simulink model "DFL_IMAP"  (R2018b)
settings: Solver=FixedStepDiscrete  StartTime=0.0  StopTime=10.0  FixedStep=0.01  RelTol=1e-3
(part 3 of 5)

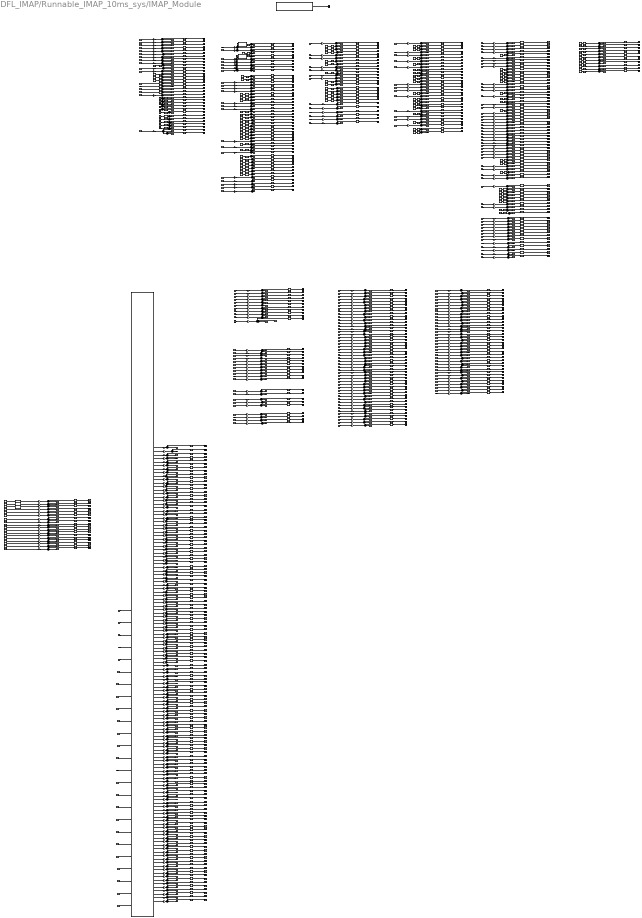
== system DFL_IMAP/Runnable_IMAP_10ms_sys/IMAP_Module ==
  note: SDFA_Lane_Back
  note: SDFA_Lane
  note: SDFA_Obj
  note: SDFA_Sensor_Status
  note: ORI
  note: EMS
  note: BCM
  note: ESC
  note: MP5
  note: EPS
  note: DMS
  SWINve_y_ABS_in_regulation : Inport
  SWINve_g_ACCEL_LONGI_CALIB : Inport  Port=2
  SWINve_y_ASR_ESP_disconnected : Inport  Port=3
  SWINve_y_ASR_in_regulation : Inport  Port=4
  SWINve_y_BCM_State_Front_Wiper : Inport  Port=5
  SWINve_y_Brake_secondary_contact : Inport  Port=6
  SWINve_y_EMS_ACC_Effecitive_EMS : Inport  Port=7
  SWINve_y_EMS_ACCcontrol_Available : Inport  Port=8
  SWINve_g_EMS_Acceleration_pedal_position : Inport  Port=9
  SWINve_g_EMS_Actual_torque : Inport  Port=10
  SWINve_d_EMS_Engine_RPM : Inport  Port=11
  SWINve_y_EMS_Engine_state : Inport  Port=12
  SWINve_g_EMS_WhlTrq_max : Inport  Port=13
  SWINve_g_EMS_WhlTrq_min : Inport  Port=14
  SWINve_y_ESP_in_regulation : Inport  Port=15
  SWINve_y_Front_Left_pulse_malfunction : Inport  Port=16
  SWINve_y_Front_right_pulse_malfunction : Inport  Port=17
  SWINve_y_GW_BCM_SEV_main_state : Inport  Port=18
  SWINve_y_GW_EMS_EMS_Status_ACC : Inport  Port=19
  SWINve_y_GW_Mp5_ISA_Switch : Inport  Port=20
  SWINve_y_GW_Mp5_TSR_Switch : Inport  Port=21
  SWINve_y_High_beam_state : Inport  Port=22
  SWINve_y_IC_Fcw_Activation_Config : Inport  Port=23
  SWINve_y_IC_FCW_Sensitivity : Inport  Port=24
  SWINve_y_IC_passengerBeltSwitchSig : Inport  Port=25
  SWINve_y_IC_seat_bealt_driver_state : Inport  Port=26
  SWINve_y_Internal_SWS_status : Inport  Port=27
  SWINve_g_Lateral_acceleration : Inport  Port=28
  SWINve_y_LC_Mode : Inport  Port=29
  SWINve_y_LKA_main_switch : Inport  Port=30
  SWINve_y_MP5_AEB_Activation_Config : Inport  Port=31
  SWINve_g_No_filtered_front_left_speed : Inport  Port=32
  SWINve_g_No_filtered_front_right_speed : Inport  Port=33
  SWINve_g_No_filtered_rear_left_speed : Inport  Port=34
  SWINve_g_No_filtered_rear_rignt_speed : Inport  Port=35
  SWINve_g_number_of_kilometer : Inport  Port=36
  SWINve_y_Park_brake_function_status : Inport  Port=37
  SWINve_g_Pulse_counter_front_left_wheel : Inport  Port=38
  SWINve_g_Pulse_counter_front_right_wheel : Inport  Port=39
  SWINve_g_Pulse_counter_rearleft_wheel : Inport  Port=40
  SWINve_g_Pulse_counter_rearright_wheel : Inport  Port=41
  SWINve_y_Rear_Left_pulse_malfunction : Inport  Port=42
  SWINve_y_Rear_Right_pulse_malfunction : Inport  Port=43
  SWINve_y_Request_to_light_fault_lamp : Inport  Port=44
  SWINve_y_State_indicating_steer_or_not : Inport  Port=45
  SWINve_y_State_of_EPS_for_LKA_function : Inport  Port=46
  SWINve_g_Steering_wheel_angle : Inport  Port=47
  SWINve_g_Steering_wheel_rotation_speed : Inport  Port=48
  SWINve_y_SWS_calibration : Inport  Port=49
  SWINve_y_SWS_trim : Inport  Port=50
  SWINve_y_TCU_AGB_Target_position : Inport  Port=51
  SWINve_y_TCU_ATFailure : Inport  Port=52
  SWINve_y_TCU_Gear_lever_position : Inport  Port=53
  SWINve_g_TMC_pressure : Inport  Port=54
  SWINve_y_Vehicle_Hold_Status : Inport  Port=55
  SWINve_g_Vehicle_speed_of_wheelsensor : Inport  Port=56
  SWINve_g_Yaw_speed : Inport  Port=57
  System_Clock : Inport  Port=58
  SDFAve_d_sensor_status : Inport  Port=59
  SDFAve_d_sen_sta_LF_radar : Inport  Port=60
  SDFAve_d_sen_sta_RF_radar : Inport  Port=61
  SDFAve_d_sen_sta_LB_radar : Inport  Port=62
  SDFAve_d_sen_sta_RB_radar : Inport  Port=63
  SDFAve_d_fusion_status : Inport  Port=64
  SDFAve_g_fusion_time_stamp : Inport  Port=65
  SDFAve_d_obj_Num : Inport  Port=66
  SDFAva_y_obj_id : Inport  Port=67
  SDFAva_g_obj_pos_x : Inport  Port=68
  SDFAva_g_obj_pos_y : Inport  Port=69
  SDFAva_g_obj_vel_x : Inport  Port=70
  SDFAva_g_obj_vel_y : Inport  Port=71
  SDFAva_g_obj_acc_x : Inport  Port=72
  SDFAva_g_obj_acc_y : Inport  Port=73
  SDFAva_g_obj_pos_var_x : Inport  Port=74
  SDFAva_g_obj_pos_var_y : Inport  Port=75
  SDFAva_g_obj_pos_var_xy : Inport  Port=76
  SDFAva_g_obj_width : Inport  Port=77
  SDFAva_g_obj_length : Inport  Port=78
  SDFAva_y_obj_class : Inport  Port=79
  SDFAva_y_obj_lane : Inport  Port=80
  SDFAva_y_obj_status : Inport  Port=81
  SDFAva_d_obj_age : Inport  Port=82
  SDFAva_y_obj_TurnLight : Inport  Port=83
  SDFAva_y_obj_BrakeLight : Inport  Port=84
  SDFAva_y_obj_MotionStatus : Inport  Port=85
  SDFAve_y_LANE_DETECT_ACTIV : Inport  Port=86
  SDFAve_y_ROAD_TYPE : Inport  Port=87
  SDFAve_y_CONSTRUCTION_AREA : Inport  Port=88
  SDFAve_g_L0_C0_COEF : Inport  Port=89
  SDFAve_g_L0_C1_COEF : Inport  Port=90
  SDFAve_g_L0_C2_COEF : Inport  Port=91
  SDFAve_g_L0_C3_COEF : Inport  Port=92
  SDFAve_g_L0_VIEW_RANGE : Inport  Port=93
  SDFAve_y_L0_DETECT_QUALITY : Inport  Port=94
  SDFAve_d_L0_LINE_TYPE : Inport  Port=95
  SDFAve_g_L0_LINE_COFIDENCE : Inport  Port=96
  SDFAve_g_L0_MARK_WIDTH : Inport  Port=97
  SDFAve_g_L0_TLC : Inport  Port=98
  SDFAve_y_L0_LANE_CHANGE : Inport  Port=99
  SDFAve_g_R0_C0_COEF : Inport  Port=100
  SDFAve_g_R0_C1_COEF : Inport  Port=101
  SDFAve_g_R0_C2_COEF : Inport  Port=102
  SDFAve_g_R0_C3_COEF : Inport  Port=103
  SDFAve_g_R0_VIEW_RANGE : Inport  Port=104
  SDFAve_y_R0_DETECT_QUALITY : Inport  Port=105
  SDFAve_d_R0_LINE_TYPE : Inport  Port=106
  SDFAve_g_R0_LINE_COFIDENCE : Inport  Port=107
  SDFAve_g_R0_MARK_WIDTH : Inport  Port=108
  SDFAve_g_R0_TLC : Inport  Port=109
  SDFAve_y_R0_LANE_CHANGE : Inport  Port=110
  SDFAve_g_L1_C0_COEF : Inport  Port=111
  SDFAve_g_L1_C1_COEF : Inport  Port=112
  SDFAve_g_L1_C2_COEF : Inport  Port=113
  SDFAve_g_L1_C3_COEF : Inport  Port=114
  SDFAve_g_L1_VIEW_RANGE : Inport  Port=115
  SDFAve_y_L1_DETECT_QUALITY : Inport  Port=116
  SDFAve_d_L1_LINE_TYPE : Inport  Port=117
  SDFAve_g_L1_LINE_COFIDENCE : Inport  Port=118
  SDFAve_g_L1_MARK_WIDTH : Inport  Port=119
  SDFAve_g_L1_TLC : Inport  Port=120
  SDFAve_y_L1_LANE_CHANGE : Inport  Port=121
  SDFAve_g_R1_C0_COEF : Inport  Port=122
  SDFAve_g_R1_C1_COEF : Inport  Port=123
  SDFAve_g_R1_C2_COEF : Inport  Port=124
  SDFAve_g_R1_C3_COEF : Inport  Port=125
  SDFAve_g_R1_VIEW_RANGE : Inport  Port=126
  SDFAve_y_R1_DETECT_QUALITY : Inport  Port=127
  SDFAve_d_R1_LINE_TYPE : Inport  Port=128
  SDFAve_g_R1_LINE_COFIDENCE : Inport  Port=129
  SDFAve_g_R1_MARK_WIDTH : Inport  Port=130
  SDFAve_g_R1_TLC : Inport  Port=131
  SDFAve_y_R1_LANE_CHANGE : Inport  Port=132
  SDFAve_g_L0_C0_BACK_COEF : Inport  Port=133
  SDFAve_g_L0_C1_BACK_COEF : Inport  Port=134
  SDFAve_g_L0_C2_BACK_COEF : Inport  Port=135
  SDFAve_g_L0_C3_BACK_COEF : Inport  Port=136
  SDFAve_g_L0_BACK_RANGE : Inport  Port=137
  SDFAve_g_L0_C0_FR_PRE_COEF : Inport  Port=138
  SDFAve_g_L0_C1_FR_PRE_COEF : Inport  Port=139
  SDFAve_g_L0_C2_FR_PRE_COEF : Inport  Port=140
  SDFAve_g_L0_FR_PRED_RANGE : Inport  Port=141
  SDFAve_g_R0_C0_BACK_COEF : Inport  Port=142
  SDFAve_g_R0_C1_BACK_COEF : Inport  Port=143
  SDFAve_g_R0_C2_BACK_COEF : Inport  Port=144
  SDFAve_g_R0_C3_BACK_COEF : Inport  Port=145
  SDFAve_g_R0_BACK_RANGE : Inport  Port=146
  SDFAve_g_R0_C0_FR_PRE_COEF : Inport  Port=147
  SDFAve_g_R0_C1_FR_PRE_COEF : Inport  Port=148
  SDFAve_g_R0_C2_FR_PRE_COEF : Inport  Port=149
  SDFAve_g_R0_FR_PRED_RANGE : Inport  Port=150
  SDFAve_g_L1_C0_BACK_COEF : Inport  Port=151
  SDFAve_g_L1_C1_BACK_COEF : Inport  Port=152
  SDFAve_g_L1_C2_BACK_COEF : Inport  Port=153
  SDFAve_g_L1_C3_BACK_COEF : Inport  Port=154
  SDFAve_g_L1_BACK_RANGE : Inport  Port=155
  SDFAve_g_L1_C0_FR_PRE_COEF : Inport  Port=156
  SDFAve_g_L1_C1_FR_PRE_COEF : Inport  Port=157
  SDFAve_g_L1_C2_FR_PRE_COEF : Inport  Port=158
  SDFAve_g_L1_FR_PRED_RANGE : Inport  Port=159
  SDFAve_g_R1_C0_BACK_COEF : Inport  Port=160
  SDFAve_g_R1_C1_BACK_COEF : Inport  Port=161
  SDFAve_g_R1_C2_BACK_COEF : Inport  Port=162
  SDFAve_g_R1_C3_BACK_COEF : Inport  Port=163
  SDFAve_g_R1_BACK_RANGE : Inport  Port=164
  SDFAve_g_R1_C0_FR_PRE_COEF : Inport  Port=165
  SDFAve_g_R1_C1_FR_PRE_COEF : Inport  Port=166
  SDFAve_g_R1_C2_FR_PRE_COEF : Inport  Port=167
  SDFAve_g_R1_FR_PRED_RANGE : Inport  Port=168
  SDFAve_y_SIGN_ISA_Value : Inport  Port=169
  SDFAve_y_TSR_Sign_Type : Inport  Port=170
  SDFAve_y_CameraSignalFault : Inport  Port=171
  SWINve_y_ESC_FLWDirection : Inport  Port=172  OutDataTypeStr=uint8  PortDimensions=1
  SWINve_y_ESC_FRWDirection : Inport  Port=173  OutDataTypeStr=uint8  PortDimensions=1
  SWINve_y_ESC_TCSErrorStatus : Inport  Port=174  OutDataTypeStr=uint8  PortDimensions=1
  SWINve_y_ESC-RLWDirection : Inport  Port=175  OutDataTypeStr=uint8  PortDimensions=1
  SWINve_y_ESC_RRWDirection : Inport  Port=176  OutDataTypeStr=uint8  PortDimensions=1
  SWINve_y_ESC_EPBErrorStatus : Inport  Port=177  OutDataTypeStr=uint8  PortDimensions=1
  SWINve_y_MP5_AutoPilotSwitch : Inport  Port=178  OutDataTypeStr=uint8
  SWINve_y_Mp5_ISAMode : Inport  Port=179  OutDataTypeStr=uint8  PortDimensions=1
  SWINve_y_Mp5_LDWWarningMode : Inport  Port=180  OutDataTypeStr=uint8  PortDimensions=1
  SWINve_y_MP5_TLCModeSelection : Inport  Port=181  OutDataTypeStr=uint8  PortDimensions=1
  SWINve_y_MP5_ESASwitch : Inport  Port=182  OutDataTypeStr=uint8  PortDimensions=1
  SWINve_y_MP5_BSD_LCW_Activation : Inport  Port=183  OutDataTypeStr=uint8  PortDimensions=1
  SWINve_y_MP5_FCTAActivation : Inport  Port=184  OutDataTypeStr=uint8  PortDimensions=1
  SWINve_y_MP5_RCTAActivation : Inport  Port=185  OutDataTypeStr=uint8  PortDimensions=1
  SWINve_y_MP5_DOWActivation : Inport  Port=186  OutDataTypeStr=uint8  PortDimensions=1
  SWINve_y_MP5_JASwitch : Inport  Port=187  OutDataTypeStr=uint8
  SWINve_y_BCM_DoorLockSt : Inport  Port=188  OutDataTypeStr=uint8  PortDimensions=1
  SWINve_y_BCM_LowBeamStatus : Inport  Port=189
  SWINve_g_AC_AmbTemp : Inport  Port=190
  SWINve_y_ESC_LateralAccelarationValidity : Inport  Port=191  OutDataTypeStr=uint8  PortDimensions=1
  SWINve_y_ESC_YawrateValidity : Inport  Port=192  OutDataTypeStr=uint8
  SWINve_y_ESC_LongitudinalAccelerationValidity : Inport  Port=193  OutDataTypeStr=uint8
  SWINve_y_ESC_ABSValidity : Inport  Port=194  OutDataTypeStr=uint8
  SWINve_y_ESC_FLWHeelSpdFaultSignal : Inport  Port=195  OutDataTypeStr=uint8
  SWINve_y_ESC_FRWHeelSpdFaultSignal : Inport  Port=196  OutDataTypeStr=uint8
  SWINve_y_ESC_RLWHeelSpdFaultSignal : Inport  Port=197  OutDataTypeStr=uint8
  SWINve_y_ESC_RRWHeelSpdFaultSignal : Inport  Port=198  OutDataTypeStr=uint8
  SWINve_y_ESC_AEBAvailable : Inport  Port=199  OutDataTypeStr=uint8
  SWINve_y_ESC_AEBActive : Inport  Port=200  OutDataTypeStr=uint8
  SWINve_y_ESC_ACCAvailable : Inport  Port=201  OutDataTypeStr=uint8
  SWINve_y_ESC_ACCActive : Inport  Port=202  OutDataTypeStr=uint8
  SWINve_y_ESC_EBDAlarmSig : Inport  Port=203  OutDataTypeStr=uint8
  SWINve_y_BCM_LeftlightSt : Inport  Port=204  OutDataTypeStr=uint8  PortDimensions=1
  SWINve_y_BCM_RightlightSt : Inport  Port=205  OutDataTypeStr=uint8  PortDimensions=1
  SWINve_y_BCM_TrunkSt : Inport  Port=206  OutDataTypeStr=uint8  PortDimensions=1
  SWINve_y_BCM_LFDoorSwitchSt : Inport  Port=207  OutDataTypeStr=uint8  PortDimensions=1
  SWINve_y_BCM_RFDoorSwitchSt : Inport  Port=208  OutDataTypeStr=uint8  PortDimensions=1
  SWINve_y_BCM_RRDoorSwitchSt : Inport  Port=209  OutDataTypeStr=uint8  PortDimensions=1
  SWINve_y_BCM_LRDoorSwitchSt : Inport  Port=210  OutDataTypeStr=uint8  PortDimensions=1
  SWINve_y_High_Beam_Status : Inport  Port=211
  SWINve_y_Front_Fog_Lamp_Status : Inport  Port=212
  SWINve_y_Rear_Fog_Lamp_Status : Inport  Port=213
  SWINve_y_BCM1_Rain_Intensity : Inport  Port=214
  SWINve_y_BCM1_IND_OvertakinglampSwt_OnOff : Inport  Port=215
  SWINve_y_kick_down : Inport  Port=216
  SWINve_g_Mech_Loss_Eng_Trq : Inport  Port=217
  SWINve_y_Powertrain_Torque_Validity : Inport  Port=218
  SWINve_y_ESP_Status_ACCInfo_Error : Inport  Port=219
  SWINve_y_ESP_Status_Prefill_Response : Inport  Port=220
  SWINve_y_ESP_Status_AEBJerk_Response : Inport  Port=221
  SWINve_y_ESP_Status_FCW_DBS_Response : Inport  Port=222
  SWINve_y_ESP_Status_AEBJerk_Available : Inport  Port=223
  SWINve_y_ESP_Status_FCW_DBS_Available : Inport  Port=224
  SWINve_y_ESP_Status_Prefill_Available : Inport  Port=225
  SWINve_g_EPS1_IND_LKAOverlayTorque_Value : Inport  Port=226
  SWINve_g_EPS1_IND_DriverTorque_Value : Inport  Port=227
  SWINve_y_EPS1_Status_HandsoffValid : Inport  Port=228
  CAFDva_y_F_CameraData600 : Inport  Port=229  OutDataTypeStr=uint8  PortDimensions=66
  CAFDva_y_F_CameraData424 : Inport  Port=230  OutDataTypeStr=uint8  PortDimensions=66
  CAFDva_y_F_CameraData425 : Inport  Port=231  OutDataTypeStr=uint8  PortDimensions=66
  CAFDva_y_F_CameraData450 : Inport  Port=232  OutDataTypeStr=uint8  PortDimensions=66
  CAFDva_y_F_CameraData459 : Inport  Port=233  OutDataTypeStr=uint8  PortDimensions=66
  CAFDva_y_F_CameraData45A : Inport  Port=234  OutDataTypeStr=uint8  PortDimensions=66
  CAFDva_y_F_CameraData45B : Inport  Port=235  OutDataTypeStr=uint8  PortDimensions=66
  CAFDva_y_F_CameraData45C : Inport  Port=236  OutDataTypeStr=uint8  PortDimensions=66
  CAFDva_y_F_CameraData45D : Inport  Port=237  OutDataTypeStr=uint8  PortDimensions=66
  CAFDva_y_F_CameraData45E : Inport  Port=238  OutDataTypeStr=uint8  PortDimensions=66
  CAFDva_y_F_CameraData45F : Inport  Port=239  OutDataTypeStr=uint8  PortDimensions=66
  CAFDva_y_F_CameraData420 : Inport  Port=240  OutDataTypeStr=uint8  PortDimensions=66
  CAFDva_y_F_CameraData421 : Inport  Port=241  OutDataTypeStr=uint8  PortDimensions=66
  CAFDva_y_F_CameraData422 : Inport  Port=242  OutDataTypeStr=uint8  PortDimensions=66
  CAFDva_y_F_CameraData451 : Inport  Port=243  OutDataTypeStr=uint8  PortDimensions=66
  CAFDva_y_F_CameraData423 : Inport  Port=244  OutDataTypeStr=uint8  PortDimensions=66
  CAFDva_y_F_CameraData452 : Inport  Port=245  OutDataTypeStr=uint8  PortDimensions=66
  CAFDva_y_F_CameraData453 : Inport  Port=246  OutDataTypeStr=uint8  PortDimensions=66
  CAFDva_y_F_CameraData454 : Inport  Port=247  OutDataTypeStr=uint8  PortDimensions=66
  CAFDva_y_F_CameraData455 : Inport  Port=248  OutDataTypeStr=uint8  PortDimensions=66
  CAFDva_y_F_CameraData456 : Inport  Port=249  OutDataTypeStr=uint8  PortDimensions=66
  CAFDva_y_F_CameraData457 : Inport  Port=250  OutDataTypeStr=uint8  PortDimensions=66
  CAFDva_y_F_CameraData458 : Inport  Port=251  OutDataTypeStr=uint8  PortDimensions=66
  CAFDva_y_F_CameraData426 : Inport  Port=252  OutDataTypeStr=uint8  PortDimensions=66
  CAFDva_y_F_CameraData47E : Inport  Port=253  OutDataTypeStr=uint8  PortDimensions=66
  Constant{1..6,8..17,22..23,29,31..32,34,37,43,48..49,51,54,57..59,61,66,71..74,77..90,92..158,163..164} (120 alike) : Constant  Value=0  OutDataTypeStr=uint16  SampleTime=-1
  Constant7 : Constant  Value=0  OutDataTypeStr=uint32  SampleTime=-1
  Data Type Conversion{,8..12,14..17,137,332..333,339,347..348,355..359,372..373,402,424,432..433,435..440,442,444..457,460..466,468,470,473..483,500..521} (90 alike) : DataTypeConversion  OutDataTypeStr=uint16
  Data Type Conversion{1..7,18..136,138..331,342..346,349..354,360..371,374..401,403..423,425..428,458,467,484..499,523..590} (482 alike) : DataTypeConversion
  Data Type Conversion13 : DataTypeConversion  OutDataTypeStr=uint32
  Data Type Conversion{334..338,340..341,429..430,434,441,443,459,469,471..472,522} (17 alike) : DataTypeConversion  OutDataTypeStr=single
  Gain{,288,354..357,359..360,364..370,380..381,384,386..387,390,392,396..397,400..403,405..406,408..416,421..427,432..434} (49 alike) : Gain  OutDataTypeStr=single  SaturateOnIntegerOverflow=on  ParamDataTypeStr=Inherit: Same as input
  Gain{1..2,4..5,8,12..16,19,23,25..30,32,34..37,39..58,63..68,71..72,74..78,81,83..85,87..93,101..103,108..109,138,142,149,155..156,162..163,169..170,176..177,181..189,195..197,203..206,216..218,228..233,235..236,240..241,245,248..249,253,255,259,263,268,272..273,276,279,286..287,289..290,292,304..305,307..308,314,317,336,342..348,350..353,373..374,378..379,385,391,443} (154 alike) : Gain  OutDataTypeStr=uint16
  Gain{3,6..7,9..11,17..18,20..22,24,31,33,38,59..62,69..70,73,104..107,110..137,139..141,143..148,150..154,157..161,164..168,171..175,178..180,191,198..200,213..214,219..227,234,238..239,242..244,246..247,250..252,254,256..258,260,262,264,266..267,270..271,274..275,277..278,281,283,375..377,444} (133 alike) : Gain  OutDataTypeStr=single
  Gain100 : Gain  OutDataTypeStr=uint32
  Gain{237,261,265,269} (4 alike) : Gain  Gain=0.5  OutDataTypeStr=single
  Gain{358,361..363,371..372,382..383,388..389,393..395,398,404,407,417..420,428..431,435..441} (31 alike) : Gain  OutDataTypeStr=uint16  SaturateOnIntegerOverflow=on  ParamDataTypeStr=Inherit: Same as input
  Gain399 : Gain  SaturateOnIntegerOverflow=on  OutDataTypeStr=Inherit: Same as input  ParamDataTypeStr=Inherit: Same as input
  Terminator{1..483} (483 alike) : Terminator
  Version : Constant  Value=331  OutDataTypeStr=uint16
  array_transfer : MATLAB Function  TreatAsAtomicUnit=on
  array_transfer10 : MATLAB Function  TreatAsAtomicUnit=on
  array_transfer11 : MATLAB Function  TreatAsAtomicUnit=on
  array_transfer3 : MATLAB Function  TreatAsAtomicUnit=on
  array_transfer8 : MATLAB Function  TreatAsAtomicUnit=on
  message_unpack : MATLAB Function  TreatAsAtomicUnit=on
  IMAPve_d_LKA_Main_Switch : Outport
  IMAPve_d_LKA_Mode : Outport  Port=2
  IMAPve_d_AEB_Switch : Outport  Port=3
  IMAPve_d_FCW_Switch : Outport  Port=4
  IMAPve_d_FCW_Sensitivity : Outport  Port=5
  IMAPve_d_ISA_Switch : Outport  Port=6
  IMAPve_d_TSR_Switch : Outport  Port=7
  IMAPve_d_ISA_ISLC_Mode : Outport  Port=8
  IMAPve_d_LDW_Warn_Mode : Outport  Port=9
  IMAPve_d_Speed_Limit : Outport  Port=10
  IMAPve_d_ALC_TLC_Mode : Outport  Port=11
  IMAPve_d_ESA_Switch : Outport  Port=12
  IMAPve_d_ELK_Switch : Outport  Port=13
  IMAPve_d_APA_Command : Outport  Port=14
  IMAPve_d_PEPS_RKE_Command : Outport  Port=15
  IMAPve_d_BSD_LCW_Switch : Outport  Port=16
  IMAPve_d_FCTA_Switch : Outport  Port=17
  IMAPve_d_RCTA_Swtich : Outport  Port=18
  IMAPve_d_DOW_Switch : Outport  Port=19
  IMAPve_d_JA_Brake_Switch : Outport  Port=20
  IMAPve_d_JA_Alert_Switch : Outport  Port=21
  IMAPve_d_JA_Alert_Sensitivity : Outport  Port=22
  IMAPve_d_LF_Switch : Outport  Port=23
  IMAPve_d_ICA_Config : Outport  Port=24
  IMAPve_d_ALC_Sensitivity : Outport  Port=25
  IMAPve_d_EPS_LKA_State : Outport  Port=26
  IMAPve_g_EPS_SW_Trq : Outport  Port=27
  IMAPve_d_EPS_Error_State : Outport  Port=28
  IMAPve_d_EPS_Trq_State : Outport  Port=29
  IMAPve_d_SAS_Clb_State : Outport  Port=30
  IMAPve_d_SAS_Trim_State : Outport  Port=31
  IMAPve_d_EPS_TrqLim_State : Outport  Port=32
  IMAPve_g_EPS_LKA_Current : Outport  Port=33
  IMAPve_g_ESC_LatAcc : Outport  Port=34
  IMAPve_d_ESC_LatAcc_Valid : Outport  Port=35
  IMAPve_g_ESC_YawRate : Outport  Port=36
  IMAPve_d_ESC_YawRate_Valid : Outport  Port=37
  IMAPve_g_ESC_UnYawRate : Outport  Port=38
  IMAPve_g_ESC_VehSpd : Outport  Port=39
  IMAPve_g_ESC_LonAcc : Outport  Port=40
  IMAPve_d_ESC_LonAcc_Valid : Outport  Port=41
  IMAPve_g_ESC_Brake_Press : Outport  Port=42
  IMAPve_g_ESC_Static_Slope : Outport  Port=43
  IMAPve_g_ESC_DySlope_Accuracy : Outport  Port=44
  IMAPve_g_ESC_DySlope : Outport  Port=45
  IMAPve_g_SW_Angle : Outport  Port=46
  IMAPve_g_SW_Angle_Speed : Outport  Port=47
  IMAPve_d_BCM_HazardLamp : Outport  Port=48
  IMAPve_d_BCM_Left_Light : Outport  Port=49
  IMAPve_d_BCM_Right_Light : Outport  Port=50
  IMAPve_d_ESC_BrakeLamp_Req : Outport  Port=51
  IMAPve_d_BCM_Opening_State : Outport  Port=52
  IMAPve_d_BCM_Trunk_State : Outport  Port=53
  IMAPve_d_BCM_LF_Door_State : Outport  Port=54
  IMAPve_d_BCM_RF_Door_State : Outport  Port=55
  IMAPve_d_BCM_RR_Door_State : Outport  Port=56
  IMAPve_d_BCM_LR_Door_State : Outport  Port=57
  IMAPve_d_SCC_Right_SwitchSig : Outport  Port=58
  IMAPve_d_PEPS_Door_Lock_Req : Outport  Port=59
  IMAPve_d_BCM_Door_Lock_State : Outport  Port=60
  IMAPve_d_EMS_ACC_Status : Outport  Port=61
  IMAPve_g_EMS_Pot_WhlT_Max : Outport  Port=62
  IMAPve_g_EMS_Pot_WhlT_Min : Outport  Port=63
  IMAPve_g_EMS_RealPedal : Outport  Port=64
  IMAPve_g_EMS_MaxTWhl : Outport  Port=65
  IMAPve_g_EMS_MaxTWhl_Offset : Outport  Port=66
  IMAPve_g_EMS_MinTWhl : Outport  Port=67
  IMAPve_g_EMS_MinTWhl_Offset : Outport  Port=68
  IMAPve_g_EMS_Actual_FlwT : Outport  Port=69
  IMAPve_g_EMS_Actual_IndT : Outport  Port=70
  IMAPve_g_EMS_Realize_TWhl : Outport  Port=71
  IMAPve_g_EMS_ACC_VirtualPedal : Outport  Port=72
  IMAPve_d_EMS_AccPedal_Fault : Outport  Port=73
  IMAPve_g_EMS_Driver_Torque : Outport  Port=74
  IMAPve_d_ESC_Brake_Effort : Outport  Port=75
  IMAPve_g_EMS_Engine_Speed : Outport  Port=76
  IMAPve_d_ESC_Veh_Standstill : Outport  Port=77
  IMAPve_d_TCU_Actual_Gear : Outport  Port=78
  IMAPve_d_TCU_Target_Gear : Outport  Port=79
  IMAPve_d_TCU_PRND_State : Outport  Port=80
  IMAPve_d_BCM_Ignition_State : Outport  Port=81
  IMAPve_d_ACU_Driver_Belt : Outport  Port=82
  IMAPve_d_SWS_Fault_Code : Outport  Port=83
  IMAPve_d_SWS_Failure_Status : Outport  Port=84
  IMAPve_d_ESC_OFF : Outport  Port=85
  IMAPve_d_ESC_AlarmSig : Outport  Port=86
  IMAPve_d_Speed_Limit_Switch : Outport  Port=87
  IMAPve_d_ESC_ESC_Active : Outport  Port=88
  IMAPve_d_ESC_MSR_Active : Outport  Port=89
  IMAPve_d_ESC_TCS_Active : Outport  Port=90
  IMAPve_d_ESC_VehSpd_Valid : Outport  Port=91
  IMAPve_d_Brake_Pedal_Fault : Outport  Port=92
  IMAPve_d_ESC_ABS_Active : Outport  Port=93
  IMAPve_d_ESC_ABS_Valid : Outport  Port=94
  IMAPve_d_ESC_ABS_AlarmSig : Outport  Port=95
  IMAPve_d_ESC_FL_WheelPulVal : Outport  Port=96
  IMAPve_d_ESC_FR_WheelPulVal : Outport  Port=97
  IMAPve_d_ESC_RL_WheelPulVal : Outport  Port=98
  IMAPve_d_ESC_RR_WheelPulVal : Outport  Port=99
  IMAPve_g_ESC_FL_WhlSpd : Outport  Port=100
  IMAPve_d_ESC_FL_WhlSpd_Fault : Outport  Port=101
  IMAPve_g_ESC_FR_WhlSpd : Outport  Port=102
  IMAPve_d_ESC_FR_WhlSpd_Fault : Outport  Port=103
  IMAPve_g_ESC_RL_WhlSpd : Outport  Port=104
  IMAPve_d_ESC_RL_WhlSpd_Fault : Outport  Port=105
  IMAPve_g_ESC_RR_WhlSpd : Outport  Port=106
  IMAPve_d_ESC_RR_WhlSpd_Fault : Outport  Port=107
  IMAPve_d_ESC_FL_Wheel_Pulse : Outport  Port=108
  IMAPve_d_ESC_FR_Wheel_Pulse : Outport  Port=109
  IMAPve_d_ESC_RL_Wheel_Pulse : Outport  Port=110
  IMAPve_d_ESC_RR_Wheel_Pulse : Outport  Port=111
  IMAPve_d_TCU_AT_Failure : Outport  Port=112
  IMAPve_d_TCU_Shift_Valid : Outport  Port=113
  IMAPve_d_TCU_DCT_Clutch_State : Outport  Port=114
  IMAPve_d_TCU_Gear_Engage : Outport  Port=115
  IMAPve_d_TCU_Select_ATMode : Outport  Port=116
  IMAPve_d_EMS_Engine_Status : Outport  Port=117
  IMAPve_d_EMS_Gearbox_CtlAvail : Outport  Port=118
  IMAPve_d_ESC_Brake_Failsafe : Outport  Port=119
  IMAPve_d_ESC_AEB_Status : Outport  Port=120
  IMAPve_d_ESC_AEB_Available : Outport  Port=121
  IMAPve_d_ESC_AEB_Active : Outport  Port=122
  IMAPve_d_ESC_ACC_Status : Outport  Port=123
  IMAPve_d_ESC_ACC_Available : Outport  Port=124
  IMAPve_d_ESC_ACC_Active : Outport  Port=125
  IMAPve_d_EMS_ACC_Effective : Outport  Port=126
  IMAPve_d_BCM_FrontWiper_State : Outport  Port=127
  IMAPve_d_BCM_CHMSL_Status : Outport  Port=128
  IMAPve_d_BCM_BrakeLamp_State : Outport  Port=129
  IMAPve_d_GW_Brake_Only_Req : Outport  Port=130
  IMAPve_d_ACU_Passenger_Belt : Outport  Port=131
  IMAPve_d_EMS_ACC_CtlAvail : Outport  Port=132
  IMAPve_d_EMS_ACC_Inhibited : Outport  Port=133
  IMAPve_d_EMS_Brake_Pedal : Outport  Port=134
  IMAPve_d_BCM_LowBeam_State : Outport  Port=135
  IMAPve_d_BCM_HighBeam_State : Outport  Port=136
  IMAPve_d_EPB_Status : Outport  Port=137
  IMAPve_d_EPB_Display_Req : Outport  Port=138
  IMAPve_d_EPB_Warn_Req : Outport  Port=139
  IMAPve_d_EPB_Switch_State : Outport  Port=140
  IMAPve_d_EPB_Switch_Valid : Outport  Port=141
  IMAPve_d_ESC_Drive_Direction : Outport  Port=142
  IMAPve_d_ESC_Hold_State : Outport  Port=143
  IMAPve_d_EPS_Steer_Hold_State : Outport  Port=144
  IMAPve_d_EPS_Warning_State : Outport  Port=145
  IMAPve_g_EPS_PowerCon : Outport  Port=146
  IMAPve_d_ESC_EBD_AlarmSig : Outport  Port=147
  IMAPve_d_ESC_AVH_Status : Outport  Port=148
  IMAPve_d_Radar_Detective_Req : Outport  Port=149
  IMAPve_g_BCM_Battery_Voltage : Outport  Port=150
  IMAPve_d_TBOX_LocalTimeY : Outport  Port=151
  IMAPve_d_TBOX_LocalTimeM : Outport  Port=152
  IMAPve_d_TBOX_LocalTimeD : Outport  Port=153
  IMAPve_d_TBOX_LocalTimeH : Outport  Port=154
  IMAPve_d_TBOX_LocalTimeMin : Outport  Port=155
  IMAPve_d_TBOX_LocalTimeS : Outport  Port=156
  IMAPve_d_TBOX_LocalTime_Valid : Outport  Port=157
  IMAPve_d_TPMS_Warn_Indicate : Outport  Port=158
  IMAPve_d_Radar_State : Outport  Port=159
  IMAPve_d_ACC_Desired_Headway : Outport  Port=160
  IMAPve_d_Time_System_Clock : Outport  Port=161
  IMAPve_d_Signal_Time_Stamp : Outport  Port=162
  IMAPve_g_GW_IC_Odometer : Outport  Port=163
  IMAPve_g_FAPA_State : Outport  Port=164
  IMAPve_d_Outside_Temp : Outport  Port=165
  IMAPve_d_ORI_CIPV_ID : Outport  Port=166
  IMAPve_d_ORI_Obj_Num : Outport  Port=167
  IMAPva_g_ORI_Probability : Outport  Port=168
  IMAPva_d_ORI_Obj_Class : Outport  Port=169
  IMAPva_d_ORI_Obj_Motion : Outport  Port=170
  IMAPva_g_ORI_Obj_RelVel : Outport  Port=171
  IMAPva_g_ORI_Obj_LongDis : Outport  Port=172
  IMAPva_d_ORI_Obj_Lane : Outport  Port=173
  IMAPva_g_ORI_Obj_LAngle : Outport  Port=174
  IMAPva_g_ORI_Obj_RAngle : Outport  Port=175
  IMAPva_g_ORI_Obj_Width : Outport  Port=176
  IMAPva_d_ORI_Obj_ID : Outport  Port=177
  IMAPve_d_ORI_Lane_Valid : Outport  Port=178
  IMAPve_d_ORI_Lane_ConsArea : Outport  Port=179
  IMAPve_d_ORI_Lane_RoadType : Outport  Port=180
  IMAPve_g_ORI_L0_C3 : Outport  Port=181
  IMAPve_g_ORI_L0_C2 : Outport  Port=182
  IMAPve_g_ORI_L0_C1 : Outport  Port=183
  IMAPve_g_ORI_L0_C0 : Outport  Port=184
  IMAPve_d_ORI_L0_Q : Outport  Port=185
  IMAPve_d_ORI_L0_Type : Outport  Port=186
  IMAPve_g_ORI_L0_VR : Outport  Port=187
  IMAPve_g_ORI_L0_TLC : Outport  Port=188
  IMAPve_g_ORI_L0_W : Outport  Port=189
  IMAPve_d_ORI_L0_LC : Outport  Port=190
  IMAPve_g_ORI_L1_C3 : Outport  Port=191
  IMAPve_g_ORI_L1_C2 : Outport  Port=192
  IMAPve_g_ORI_L1_C1 : Outport  Port=193
  IMAPve_g_ORI_L1_C0 : Outport  Port=194
  IMAPve_d_ORI_L1_Q : Outport  Port=195
  IMAPve_d_ORI_L1_Type : Outport  Port=196
  IMAPve_g_ORI_L1_VR : Outport  Port=197
  IMAPve_g_ORI_L1_TLC : Outport  Port=198
  IMAPve_g_ORI_L1_W : Outport  Port=199
  IMAPve_d_ORI_L1_LC : Outport  Port=200
  IMAPve_g_ORI_R0_C3 : Outport  Port=201
  IMAPve_g_ORI_R0_C2 : Outport  Port=202
  IMAPve_g_ORI_R0_C1 : Outport  Port=203
  IMAPve_g_ORI_R0_C0 : Outport  Port=204
  IMAPve_d_ORI_R0_Q : Outport  Port=205
  IMAPve_d_ORI_R0_LT : Outport  Port=206
  IMAPve_g_ORI_R0_VR : Outport  Port=207
  IMAPve_g_ORI_R0_TLC : Outport  Port=208
  IMAPve_g_ORI_R0_W : Outport  Port=209
  IMAPve_d_ORI_R0_LC : Outport  Port=210
  IMAPve_g_ORI_R1_C3 : Outport  Port=211
  IMAPve_g_ORI_R1_C2 : Outport  Port=212
  IMAPve_g_ORI_R1_C1 : Outport  Port=213
  IMAPve_g_ORI_R1_C0 : Outport  Port=214
  IMAPve_d_ORI_R1_Q : Outport  Port=215
  IMAPve_d_ORI_R1_LT : Outport  Port=216
  IMAPve_g_ORI_R1_VR : Outport  Port=217
  IMAPve_g_ORI_R1_TLC : Outport  Port=218
  IMAPve_g_ORI_R1_W : Outport  Port=219
  IMAPve_d_ORI_R1_LC : Outport  Port=220
  IMAPve_d_Sensor_Status : Outport  Port=221
  IMAPve_d_LF_Radar_Status : Outport  Port=222
  IMAPve_d_RF_Radar_Status : Outport  Port=223
  IMAPve_d_LR_Radar_Status : Outport  Port=224
  IMAPve_d_RR_Radar_Status : Outport  Port=225
  IMAPve_d_Fusion_Status : Outport  Port=226
  IMAPve_g_Fusion_Time_Stamp : Outport  Port=227
  IMAPve_d_obj_Num : Outport  Port=228
  IMAPva_d_obj_id : Outport  Port=229
  IMAPva_g_obj_pos_x : Outport  Port=230
  IMAPva_g_obj_pos_y : Outport  Port=231
  IMAPva_g_obj_vel_x : Outport  Port=232
  IMAPva_g_obj_vel_y : Outport  Port=233
  IMAPva_g_obj_acc_x : Outport  Port=234
  IMAPva_g_obj_acc_y : Outport  Port=235
  IMAPva_g_obj_pos_var_x : Outport  Port=236
  IMAPva_g_obj_pos_var_y : Outport  Port=237
  IMAPva_g_obj_pos_var_xy : Outport  Port=238
  IMAPva_g_obj_width : Outport  Port=239
  IMAPva_g_obj_length : Outport  Port=240
  IMAPva_d_obj_class : Outport  Port=241
  IMAPva_d_obj_lane : Outport  Port=242
  IMAPva_d_obj_status : Outport  Port=243
  IMAPva_d_obj_age : Outport  Port=244
  IMAPva_d_obj_TurnLight : Outport  Port=245
  IMAPva_d_obj_BrakeLight : Outport  Port=246
  IMAPva_d_obj_MotionStatus : Outport  Port=247
  IMAPve_d_Lane_Valid : Outport  Port=248
  IMAPve_d_Road_Type : Outport  Port=249
  IMAPve_d_ConsArea : Outport  Port=250
  IMAPve_g_L0_C0 : Outport  Port=251
  IMAPve_g_L0_C1 : Outport  Port=252
  IMAPve_g_L0_C2 : Outport  Port=253
  IMAPve_g_L0_C3 : Outport  Port=254
  IMAPve_g_L0_VR : Outport  Port=255
  IMAPve_d_L0_Q : Outport  Port=256
  IMAPve_d_L0_Type : Outport  Port=257
  IMAPve_g_L0_Confidence : Outport  Port=258
  IMAPve_g_L0_W : Outport  Port=259
  IMAPve_g_L0_TLC : Outport  Port=260
  IMAPve_d_L0_LC : Outport  Port=261
  IMAPve_g_R0_C0 : Outport  Port=262
  IMAPve_g_R0_C1 : Outport  Port=263
  IMAPve_g_R0_C2 : Outport  Port=264
  IMAPve_g_R0_C3 : Outport  Port=265
  IMAPve_g_R0_VR : Outport  Port=266
  IMAPve_d_R0_Q : Outport  Port=267
  IMAPve_d_R0_Type : Outport  Port=268
  IMAPve_g_R0_Confidence : Outport  Port=269
  IMAPve_g_R0_W : Outport  Port=270
  IMAPve_g_R0_TLC : Outport  Port=271
  IMAPve_d_R0_LC : Outport  Port=272
  IMAPve_g_L1_C0 : Outport  Port=273
  IMAPve_g_L1_C1 : Outport  Port=274
  IMAPve_g_L1_C2 : Outport  Port=275
  IMAPve_g_L1_C3 : Outport  Port=276
  IMAPve_g_L1_VR : Outport  Port=277
  IMAPve_d_L1_Q : Outport  Port=278
  IMAPve_d_L1_Type : Outport  Port=279
  IMAPve_g_L1_Confidence : Outport  Port=280
  IMAPve_g_L1_W : Outport  Port=281
  IMAPve_g_L1_TLC : Outport  Port=282
  IMAPve_d_L1_LC : Outport  Port=283
  IMAPve_g_R1_C0 : Outport  Port=284
  IMAPve_g_R1_C1 : Outport  Port=285
  IMAPve_g_R1_C2 : Outport  Port=286
  IMAPve_g_R1_C3 : Outport  Port=287
  IMAPve_g_R1_VR : Outport  Port=288
  IMAPve_d_R1_Q : Outport  Port=289
  IMAPve_d_R1_Type : Outport  Port=290
  IMAPve_g_R1_Confidence : Outport  Port=291
  IMAPve_g_R1_W : Outport  Port=292
  IMAPve_g_R1_TLC : Outport  Port=293
  IMAPve_d_R1_LC : Outport  Port=294
  IMAPve_g_L0_C0_Back : Outport  Port=295
  IMAPve_g_L0_C1_Back : Outport  Port=296
  IMAPve_g_L0_C2_Back : Outport  Port=297
  IMAPve_g_L0_C3_Back : Outport  Port=298
  IMAPve_g_L0_Range_Back : Outport  Port=299
  IMAPve_g_L0_C0_FR_Pred : Outport  Port=300
  IMAPve_g_L0_C1_FR_Pred : Outport  Port=301
  IMAPve_g_L0_C2_FR_Pred : Outport  Port=302
  IMAPve_g_L0_Range_FR_Pred : Outport  Port=303
  IMAPve_g_R0_C0_Back : Outport  Port=304
  IMAPve_g_R0_C1_Back : Outport  Port=305
  IMAPve_g_R0_C2_Back : Outport  Port=306
  IMAPve_g_R0_C3_Back : Outport  Port=307
  IMAPve_g_R0_Range_Back : Outport  Port=308
  IMAPve_g_R0_C0_FR_Pred : Outport  Port=309
  IMAPve_g_R0_C1_FR_Pred : Outport  Port=310
  IMAPve_g_R0_C2_FR_Pred : Outport  Port=311
  IMAPve_g_R0_Range_FR_Pred : Outport  Port=312
  IMAPve_g_L1_C0_Back : Outport  Port=313
  IMAPve_g_L1_C1_Back : Outport  Port=314
  IMAPve_g_L1_C2_Back : Outport  Port=315
  IMAPve_g_L1_C3_Back : Outport  Port=316
  IMAPve_g_L1_Range_Back : Outport  Port=317
  IMAPve_g_L1_C0_FR_Pred : Outport  Port=318
  IMAPve_g_L1_C1_FR_Pred : Outport  Port=319
  IMAPve_g_L1_C2_FR_Pred : Outport  Port=320
  IMAPve_g_L1_Range_FR_Pred : Outport  Port=321
  IMAPve_g_R1_C0_Back : Outport  Port=322
  IMAPve_g_R1_C1_Back : Outport  Port=323
  IMAPve_g_R1_C2_Back : Outport  Port=324
  IMAPve_g_R1_C3_Back : Outport  Port=325
  IMAPve_g_R1_Range_Back : Outport  Port=326
  IMAPve_g_R1_C0_FR_Pred : Outport  Port=327
  IMAPve_g_R1_C1_FR_Pred : Outport  Port=328
  IMAPve_g_R1_C2_FR_Pred : Outport  Port=329
  IMAPve_g_R1_Range_FR_Pred : Outport  Port=330
  IMAPve_d_Sign_ISA_Value : Outport  Port=331
  IMAPve_d_TSR_Sign_Type : Outport  Port=332
  IMAPve_d_Camera_Signal_Fault : Outport  Port=333
  IMAPve_d_Radar_Status : Outport  Port=334
  IMAPve_d_Camera_Status : Outport  Port=335
  IMAPve_d_ESC_FLW_Direction : Outport  Port=336
  IMAPve_d_ESC_FRW_Direction : Outport  Port=337
  IMAPve_d_ESC_TCS_ErrorStatus : Outport  Port=338
  IMAPve_d_ESC_RLW_Direction : Outport  Port=339
  IMAPve_d_ESC_RRW_Direction : Outport  Port=340
  IMAPve_d_ESC_EPB_ErrorStatus : Outport  Port=341
  IMAPve_d_EPS_SteeringAngle_Flag : Outport  Port=342
  IMAPve_g_EPS_SteeringAngle : Outport  Port=343
  IMAPve_d_EPS_Driver_Override : Outport  Port=344
  IMAPve_d_EPS_Driver_Active_ESA : Outport  Port=345
  IMAPve_d_EPS_ESA_State : Outport  Port=346
  IMAPve_d_ACU_RearLeft_Belt : Outport  Port=347
  IMAPve_d_ACU_RearMiddle_Belt : Outport  Port=348
  IMAPve_d_ACU_RearRight_Belt : Outport  Port=349
  IMAPve_d_EMS_PowertrainCtl_State : Outport  Port=350
  IMAPve_d_TCU_TCU_Available : Outport  Port=351
  IMAPve_d_BCM_LeftTurn_Switch : Outport  Port=352
  IMAPve_d_BCM_RightTurn_Switch : Outport  Port=353
  IMAPve_d_BCM_FrontWiper_Switch : Outport  Port=354
  IMAPve_d_BCM_IHBC_Enabled : Outport  Port=355
  IMAPve_d_MP5_Work_State : Outport  Port=356
  IMAPve_d_MP5_APA_ModeSelect : Outport  Port=357
  IMAPve_d_MP5_LanguageSet : Outport  Port=358
  IMAPve_d_MP5_UPA_Switch : Outport  Port=359
  IMAPve_d_MP5_FLK_Activation : Outport  Port=360
  IMAPve_d_MP5_AutoPilot_Switch : Outport  Port=361
  IMAPve_d_SCC_Left_SwitchSig : Outport  Port=362
  IMAPve_d_MP5_DMS_MessageType : Outport  Port=363
  IMAPve_d_MP5_DMS_SystemEnable : Outport  Port=364
  IMAPve_d_MP5_DMS_DelUserNum : Outport  Port=365
  IMAPve_d_MP5_DMS_Sensity : Outport  Port=366
  IMAPve_d_MP5_DMS_EyeFatigue : Outport  Port=367
  IMAPve_d_MP5_DMS_LongtimeDrive : Outport  Port=368
  IMAPve_d_MP5_DMS_SideView : Outport  Port=369
  IMAPve_d_MP5_DMS_UsingPhone : Outport  Port=370
  IMAPve_d_MP5_DMS_Smoking : Outport  Port=371
  IMAPve_d_MP5_DMS_DrinkWater : Outport  Port=372
  IMAPve_d_MP5_DMS_UserAccount : Outport  Port=373
  IMAPve_d_High_Beam_State : Outport  Port=374
  IMAPve_d_Front_Fog_Lamp_State : Outport  Port=375
  IMAPve_d_Rear_Fog_Lamp_State : Outport  Port=376
  IMAPve_d_BCM_Rain_Intensity : Outport  Port=377
  IMAPve_d_BCM_OvertakinglampSwt : Outport  Port=378
  IMAPve_d_EMS_Kickdown : Outport  Port=379
  IMAPve_g_EMS_Mech_Loss_Trq : Outport  Port=380
  IMAPve_d_Powertrain_Torque_Valid : Outport  Port=381
  IMAPve_d_ESC_ACCInfo_Error : Outport  Port=382
  IMAPve_d_ESC_Prefill_Response : Outport  Port=383
  IMAPve_d_ESC_AEBJerk_Response : Outport  Port=384
  IMAPve_d_ESC_FCW_DBS_Response : Outport  Port=385
  IMAPve_d_ESC_AEBJerk_Available : Outport  Port=386
  IMAPve_d_ESC_FCW_DBS_Available : Outport  Port=387
  IMAPve_d_ESC_Prefill_Available : Outport  Port=388
  IMAPve_g_EPS_LKAOverlay_Trq : Outport  Port=389
  IMAPve_g_EPS_DriverTorque : Outport  Port=390
  IMAPve_d_EPS_Steer_Hold_State_Valid : Outport  Port=391
  IMAPva_d_ORI_Obj_TimeStamp : Outport  Port=392  OutDataTypeStr=uint16  PortDimensions=20
  IMAPve_d_ORI_FS_OutOfCalib : Outport  Port=393  OutDataTypeStr=uint16
  IMAPve_d_ORI_FS_Rain : Outport  Port=394  OutDataTypeStr=uint16
  IMAPve_d_ORI_FS_Fog : Outport  Port=395  OutDataTypeStr=uint16
  IMAPve_d_ORI_FS_Splashes0 : Outport  Port=396  OutDataTypeStr=uint16
  IMAPve_d_ORI_FS_SunRay0 : Outport  Port=397  OutDataTypeStr=uint16
  IMAPve_d_ORI_FS_LowSun0 : Outport  Port=398  OutDataTypeStr=uint16
  IMAPve_d_ORI_FS_BlurImage0 : Outport  Port=399  OutDataTypeStr=uint16
  IMAPve_d_ORI_FS_PartialBlockage0 : Outport  Port=400  OutDataTypeStr=uint16
  IMAPve_d_ORI_FS_FullBlockage0 : Outport  Port=401  OutDataTypeStr=uint16
  IMAPve_d_ORI_FS_FrozenWindshield0 : Outport  Port=402  OutDataTypeStr=uint16
  IMAPve_d_ORI_FS_OutOfFocus0 : Outport  Port=403  OutDataTypeStr=uint16
  IMAPva_g_ORI_Obj_AbsAx : Outport  Port=404  OutDataTypeStr=single  PortDimensions=20
  IMAPva_g_ORI_Obj_AbsAy : Outport  Port=405  OutDataTypeStr=single  PortDimensions=20
  IMAPva_g_ORI_Obj_TTIPCStdDev : Outport  Port=406  OutDataTypeStr=single  PortDimensions=20
  IMAPva_g_ORI_Obj_RelVely : Outport  Port=407  OutDataTypeStr=single  PortDimensions=20
  IMAPva_g_ORI_Obj_LateralDis : Outport  Port=408  OutDataTypeStr=single  PortDimensions=20
  IMAPva_g_ORI_Obj_AbsAxStdDev : Outport  Port=409  OutDataTypeStr=single  PortDimensions=20
  IMAPva_g_ORI_Obj_AbsAyStdDev : Outport  Port=410  OutDataTypeStr=single  PortDimensions=20
  IMAPva_g_ORI_Obj_RelVelStdDev : Outport  Port=411  OutDataTypeStr=single  PortDimensions=20
  IMAPva_g_ORI_Obj_RelVelyStdDev : Outport  Port=412  OutDataTypeStr=single  PortDimensions=20
  IMAPva_g_ORI_Obj_LongDisStdDev : Outport  Port=413  OutDataTypeStr=single  PortDimensions=20
  IMAPva_g_ORI_Obj_LateralDisStdDev : Outport  Port=414  OutDataTypeStr=single  PortDimensions=20
  IMAPva_d_ORI_Obj_RelVelValid : Outport  Port=415  OutDataTypeStr=uint16  PortDimensions=20
  IMAPva_d_ORI_Obj_RelVelyValid : Outport  Port=416  OutDataTypeStr=uint16  PortDimensions=20
  IMAPva_d_ORI_Obj_RelVelStdDevValid : Outport  Port=417  OutDataTypeStr=uint16  PortDimensions=20
  IMAPva_d_ORI_Obj_RelVelyStdDevValid : Outport  Port=418  OutDataTypeStr=uint16  PortDimensions=20
  IMAPva_g_ORI_Obj_ExistProb : Outport  Port=419  OutDataTypeStr=single  PortDimensions=20
  IMAPva_g_ORI_Obj_ClassProb : Outport  Port=420  OutDataTypeStr=single  PortDimensions=20
  IMAPva_g_ORI_Obj_Height : Outport  Port=421  OutDataTypeStr=single  PortDimensions=20
  IMAPva_g_ORI_Obj_LengthStdDev : Outport  Port=422  OutDataTypeStr=single  PortDimensions=20
  IMAPva_g_ORI_Obj_WidthStdDev : Outport  Port=423  OutDataTypeStr=single  PortDimensions=20
  IMAPva_g_ORI_Obj_HeightStdDev : Outport  Port=424  OutDataTypeStr=single  PortDimensions=20
  IMAPva_g_ORI_Obj_3DAngle : Outport  Port=425  OutDataTypeStr=single  PortDimensions=20
  IMAPva_g_ORI_Obj_LAngleStdDev : Outport  Port=426  OutDataTypeStr=single  PortDimensions=20
  IMAPva_g_ORI_Obj_RAngleStdDev : Outport  Port=427  OutDataTypeStr=single  PortDimensions=20
  IMAPva_g_ORI_Obj_3DAngleStdDev : Outport  Port=428  OutDataTypeStr=single  PortDimensions=20
  IMAPva_g_ORI_Obj_AngleRate : Outport  Port=429  OutDataTypeStr=single  PortDimensions=20
  IMAPva_g_ORI_Obj_AngleRateStdDev : Outport  Port=430  OutDataTypeStr=single  PortDimensions=20
  IMAPva_g_ORI_Obj_PhiBottom : Outport  Port=431  OutDataTypeStr=single  PortDimensions=20
  IMAPva_g_ORI_Obj_PhiBottomStdDev : Outport  Port=432  OutDataTypeStr=single  PortDimensions=20
  IMAPva_d_ORI_Obj_Measured : Outport  Port=433  OutDataTypeStr=uint16  PortDimensions=20
  IMAPva_g_ORI_Obj_Heading : Outport  Port=434  OutDataTypeStr=single  PortDimensions=20
  IMAPva_g_ORI_Obj_HeadingStdDev : Outport  Port=435  OutDataTypeStr=single  PortDimensions=20
  IMAPva_d_ORI_Obj_HeadOrientation : Outport  Port=436  OutDataTypeStr=uint16  PortDimensions=20
  IMAPva_g_ORI_Obj_TTIPC : Outport  Port=437  OutDataTypeStr=single  PortDimensions=20
  IMAPva_d_ORI_Obj_DirectionIndicator : Outport  Port=438  OutDataTypeStr=uint16  PortDimensions=20
  IMAPva_d_ORI_Obj_BrakeLight : Outport  Port=439  OutDataTypeStr=uint16  PortDimensions=20
  IMAPve_d_ORI_L0_ID : Outport  Port=440  OutDataTypeStr=uint16
  IMAPve_g_ORI_L0_ExistProb : Outport  Port=441  OutDataTypeStr=single
  IMAPve_g_ORI_L0_DxStart : Outport  Port=442  OutDataTypeStr=single
  IMAPve_d_ORI_L0_ColorClass : Outport  Port=443  OutDataTypeStr=uint16
  IMAPve_d_ORI_L0_MeasureType : Outport  Port=444  OutDataTypeStr=uint16
  IMAPve_g_ORI_L0_TypeConf : Outport  Port=445  OutDataTypeStr=single
  IMAPve_d_ORI_R0_ID : Outport  Port=446  OutDataTypeStr=uint16
  IMAPve_g_ORI_R0_ExistProb : Outport  Port=447  OutDataTypeStr=single
  IMAPve_g_ORI_R0_Dxstart : Outport  Port=448  OutDataTypeStr=single
  IMAPve_d_ORI_R0_ColorClass : Outport  Port=449  OutDataTypeStr=uint16
  IMAPve_d_ORI_R0_MeasureType : Outport  Port=450  OutDataTypeStr=uint16
  IMAPve_g_ORI_R0_TypeConf : Outport  Port=451  OutDataTypeStr=single
  IMAPve_d_ORI_L1_ID : Outport  Port=452  OutDataTypeStr=uint16
  IMAPve_g_ORI_L1_ExistProb : Outport  Port=453  OutDataTypeStr=single
  IMAPve_g_ORI_L1_Dxstart : Outport  Port=454  OutDataTypeStr=single
  IMAPve_d_ORI_L1_ColorClass : Outport  Port=455  OutDataTypeStr=uint16
  IMAPve_d_ORI_L1_MeasureType : Outport  Port=456  OutDataTypeStr=uint16
  IMAPve_g_ORI_L1_TypeConf : Outport  Port=457  OutDataTypeStr=single
  IMAPve_d_ORI_R1_ID : Outport  Port=458  OutDataTypeStr=uint16
  IMAPve_g_ORI_R1_ExistProb : Outport  Port=459  OutDataTypeStr=single
  IMAPve_g_ORI_R1_Dxstart : Outport  Port=460  OutDataTypeStr=single
  IMAPve_d_ORI_R1_ColorClass : Outport  Port=461  OutDataTypeStr=uint16
  IMAPve_d_ORI_R1_MeasureType : Outport  Port=462  OutDataTypeStr=uint16
  IMAPve_g_ORI_R1_TypeConf : Outport  Port=463  OutDataTypeStr=single
  IMAPve_d_ORI_RoadedgeL0_ID : Outport  Port=464  OutDataTypeStr=uint16
  IMAPve_g_ORI_RoadedgeL0_ExistProb : Outport  Port=465  OutDataTypeStr=single
  IMAPve_g_ORI_RoadedgeL0_DxStart : Outport  Port=466  OutDataTypeStr=single
  IMAPve_g_ORI_RoadedgeL0_DxEnd : Outport  Port=467  OutDataTypeStr=single
  IMAPve_g_ORI_RoadedgeL0_C1 : Outport  Port=468  OutDataTypeStr=single
  IMAPve_g_ORI_RoadedgeL0_C0 : Outport  Port=469  OutDataTypeStr=single
  IMAPve_g_ORI_RoadedgeL0_C3 : Outport  Port=470  OutDataTypeStr=single
  IMAPve_g_ORI_RoadedgeL0_C2 : Outport  Port=471  OutDataTypeStr=single
  IMAPve_d_ORI_RoadedgeL0_MeasureType : Outport  Port=472  OutDataTypeStr=uint16
  IMAPve_d_ORI_RoadedgeL0_Type : Outport  Port=473  OutDataTypeStr=uint16
  IMAPve_d_ORI_RoadedgeR0_ID : Outport  Port=474  OutDataTypeStr=uint16
  IMAPve_g_ORI_RoadedgeR0_ExistProb : Outport  Port=475  OutDataTypeStr=single
  IMAPve_g_ORI_RoadedgeR0_DxStart : Outport  Port=476  OutDataTypeStr=single
  IMAPve_g_ORI_RoadedgeR0_DxEnd : Outport  Port=477  OutDataTypeStr=single
  IMAPve_g_ORI_RoadedgeR0_C1 : Outport  Port=478  OutDataTypeStr=single
  IMAPve_g_ORI_RoadedgeR0_C0 : Outport  Port=479  OutDataTypeStr=single
  IMAPve_g_ORI_RoadedgeR0_C3 : Outport  Port=480  OutDataTypeStr=single
  IMAPve_g_ORI_RoadedgeR0_C2 : Outport  Port=481  OutDataTypeStr=single
  IMAPve_d_ORI_RoadedgeR0_MeasureType : Outport  Port=482  OutDataTypeStr=uint16
  IMAPve_d_ORI_RoadedgeR0_Type : Outport  Port=483  OutDataTypeStr=uint16
  wires:
  SWINve_y_GW_Mp5_ISA_Switch/1 -> Gain187/1
  SWINve_y_LKA_main_switch/1 -> Gain182/1
  SWINve_y_LC_Mode/1 -> Gain183/1
  SWINve_y_GW_Mp5_TSR_Switch/1 -> Gain188/1
  SWINve_y_IC_FCW_Sensitivity/1 -> Gain186/1
  SWINve_y_MP5_AEB_Activation_Config/1 -> Gain184/1
  SWINve_y_IC_Fcw_Activation_Config/1 -> Gain185/1
  Gain182/1 -> Data Type Conversion34/1, IMAPve_d_LKA_Main_Switch/1  "IMAPve_d_LKA_Main_Switch"
  message_unpack/43(IFC_ObjHdr_ObjCount) -> Gain2/1
  Gain1/1 -> Data Type Conversion139/1, IMAPve_d_ORI_CIPV_ID/1  "IMAPve_d_ORI_CIPV_ID"
  Gain2/1 -> Data Type Conversion140/1, IMAPve_d_ORI_Obj_Num/1  "IMAPve_d_ORI_Obj_Num"
  Gain3/1 -> Data Type Conversion141/1, IMAPva_g_ORI_Probability/1  "IMAPva_g_ORI_Probability"
  Gain4/1 -> Data Type Conversion142/1, IMAPva_d_ORI_Obj_Class/1  "IMAPva_d_ORI_Obj_Class"
  Gain5/1 -> Data Type Conversion143/1, IMAPva_d_ORI_Obj_Motion/1  "IMAPva_d_ORI_Obj_Motion"
  Gain6/1 -> Data Type Conversion144/1, IMAPva_g_ORI_Obj_RelVel/1  "IMAPva_g_ORI_Obj_RelVel"
  Gain7/1 -> Data Type Conversion145/1, IMAPva_g_ORI_Obj_LongDis/1  "IMAPva_g_ORI_Obj_LongDis"
  Gain8/1 -> Data Type Conversion146/1, IMAPva_d_ORI_Obj_Lane/1  "IMAPva_d_ORI_Obj_Lane"
  Gain12/1 -> Data Type Conversion150/1, IMAPva_d_ORI_Obj_ID/1  "IMAPva_d_ORI_Obj_ID"
  Gain14/1 -> Data Type Conversion152/1, IMAPve_d_ORI_Lane_ConsArea/1  "IMAPve_d_ORI_Lane_ConsArea"
  Gain13/1 -> Data Type Conversion151/1, IMAPve_d_ORI_Lane_Valid/1  "IMAPve_d_ORI_Lane_Valid"
  Constant31/1 -> Gain13/1
  Constant32/1 -> Gain14/1
  Data Type Conversion522/1 -> Data Type Conversion65/1, IMAPve_g_EPS_SW_Trq/1
  Gain189/1 -> Data Type Conversion64/1, IMAPve_d_EPS_LKA_State/1  "IMAPve_d_EPS_LKA_State"
  SWINve_y_State_of_EPS_for_LKA_function/1 -> Gain189/1
  SWINve_y_SWS_trim/1 -> Gain16/1
  SWINve_y_SWS_calibration/1 -> Gain15/1
  Gain17/1 -> Data Type Conversion100/1, IMAPve_g_ESC_LatAcc/1  "IMAPve_g_ESC_LatAcc"
  SWINve_g_Lateral_acceleration/1 -> Gain17/1
  SWINve_g_Yaw_speed/1 -> Gain18/1
  Gain18/1 -> Data Type Conversion101/1, IMAPve_g_ESC_YawRate/1  "IMAPve_g_ESC_YawRate"
  Data Type Conversion441/1 -> Data Type Conversion102/1, IMAPve_g_ESC_UnYawRate/1
  SWINve_g_Vehicle_speed_of_wheelsensor/1 -> Gain20/1
  Gain20/1 -> Data Type Conversion103/1, IMAPve_g_ESC_VehSpd/1  "IMAPve_g_ESC_VehSpd"
  Gain21/1 -> Data Type Conversion104/1, IMAPve_g_ESC_LonAcc/1  "IMAPve_g_ESC_LonAcc"
  SWINve_g_ACCEL_LONGI_CALIB/1 -> Gain21/1
  Gain22/1 -> Data Type Conversion105/1, IMAPve_g_ESC_Brake_Press/1  "IMAPve_g_ESC_Brake_Press"
  SWINve_g_TMC_pressure/1 -> Gain22/1
  Data Type Conversion434/1 -> Data Type Conversion106/1, IMAPve_g_ESC_Static_Slope/1
  SWINve_g_Steering_wheel_rotation_speed/1 -> Gain24/1
  Data Type Conversion334/1 -> Data Type Conversion108/1, IMAPve_g_ESC_DySlope/1
  Data Type Conversion335/1 -> Data Type Conversion107/1, IMAPve_g_ESC_DySlope_Accuracy/1
  Gain29/1 -> Data Type Conversion75/1, IMAPve_d_EMS_ACC_Status/1  "IMAPve_d_EMS_ACC_Status"
  SWINve_y_GW_EMS_EMS_Status_ACC/1 -> Gain29/1
  Data Type Conversion429/1 -> Data Type Conversion76/1, IMAPve_g_EMS_Pot_WhlT_Max/1
  Gain31/1 -> Data Type Conversion79/1, IMAPve_g_EMS_MaxTWhl/1  "IMAPve_g_EMS_MaxTWhl"
  SWINve_g_EMS_WhlTrq_max/1 -> Gain31/1
  Data Type Conversion340/1 -> Data Type Conversion80/1, IMAPve_g_EMS_MaxTWhl_Offset/1
  SWINve_g_EMS_WhlTrq_min/1 -> Gain33/1
  Data Type Conversion430/1 -> Data Type Conversion77/1, IMAPve_g_EMS_Pot_WhlT_Min/1
  Gain38/1 -> Data Type Conversion87/1, IMAPve_g_EMS_Engine_Speed/1  "IMAPve_g_EMS_Engine_Speed"
  SWINve_d_EMS_Engine_RPM/1 -> Gain38/1
  Data Type Conversion439/1 -> Data Type Conversion110/1, IMAPve_d_ESC_Veh_Standstill/1
  Data Type Conversion338/1 -> Data Type Conversion86/1, IMAPve_g_EMS_Driver_Torque/1
  Data Type Conversion137/1 -> Data Type Conversion109/1, IMAPve_d_ESC_Brake_Effort/1
  SWINve_y_Internal_SWS_status/1 -> Gain43/1
  Gain40/1 -> Data Type Conversion52/1, IMAPve_d_BCM_Ignition_State/1  "IMAPve_d_BCM_Ignition_State"
  SWINve_y_GW_BCM_SEV_main_state/1 -> Gain40/1
  Gain41/1 -> Data Type Conversion53/1, IMAPve_d_ACU_Driver_Belt/1  "IMAPve_d_ACU_Driver_Belt"
  SWINve_y_IC_seat_bealt_driver_state/1 -> Gain41/1
  Gain45/1 -> Data Type Conversion95/1, IMAPve_d_TCU_Target_Gear/1  "IMAPve_d_TCU_Target_Gear"
  Gain44/1 -> Data Type Conversion88/1, IMAPve_d_TCU_Actual_Gear/1  "IMAPve_d_TCU_Actual_Gear"
  SWINve_y_TCU_AGB_Target_position/1 -> Gain45/1
  SWINve_y_TCU_Gear_lever_position/1 -> Gain44/1
  Gain47/1 -> Data Type Conversion112/1, IMAPve_d_ESC_AlarmSig/1  "IMAPve_d_ESC_AlarmSig"
  SWINve_y_ASR_ESP_disconnected/1 -> Gain46/1
  SWINve_y_ESP_in_regulation/1 -> Gain49/1
  Gain46/1 -> Data Type Conversion111/1, IMAPve_d_ESC_OFF/1  "IMAPve_d_ESC_OFF"
  SWINve_y_Request_to_light_fault_lamp/1 -> Gain47/1
  Gain49/1 -> Data Type Conversion113/1, IMAPve_d_ESC_ESC_Active/1  "IMAPve_d_ESC_ESC_Active"
  Data Type Conversion482/1 -> Data Type Conversion114/1, IMAPve_d_ESC_MSR_Active/1
  Data Type Conversion12/1 -> Data Type Conversion117/1, IMAPve_d_Brake_Pedal_Fault/1
  Gain54/1 -> Data Type Conversion118/1, IMAPve_d_ESC_ABS_Active/1  "IMAPve_d_ESC_ABS_Active"
  SWINve_y_ASR_in_regulation/1 -> Gain51/1
  Data Type Conversion483/1 -> Data Type Conversion116/1, IMAPve_d_ESC_VehSpd_Valid/1
  SWINve_y_ABS_in_regulation/1 -> Gain54/1
  Gain51/1 -> Data Type Conversion115/1, IMAPve_d_ESC_TCS_Active/1  "IMAPve_d_ESC_TCS_Active"
  Gain56/1 -> Data Type Conversion120/1, IMAPve_d_ESC_FR_WheelPulVal/1  "IMAPve_d_ESC_FR_WheelPulVal"
  Gain58/1 -> Data Type Conversion122/1, IMAPve_d_ESC_RR_WheelPulVal/1  "IMAPve_d_ESC_RR_WheelPulVal"
  Gain55/1 -> Data Type Conversion119/1, IMAPve_d_ESC_FL_WheelPulVal/1  "IMAPve_d_ESC_FL_WheelPulVal"
  Gain57/1 -> Data Type Conversion121/1, IMAPve_d_ESC_RL_WheelPulVal/1  "IMAPve_d_ESC_RL_WheelPulVal"
  Gain59/1 -> Data Type Conversion123/1, IMAPve_g_ESC_FL_WhlSpd/1  "IMAPve_g_ESC_FL_WhlSpd"
  SWINve_y_Rear_Left_pulse_malfunction/1 -> Gain57/1
  SWINve_g_No_filtered_front_left_speed/1 -> Gain59/1
  SWINve_y_Front_right_pulse_malfunction/1 -> Gain56/1
  SWINve_y_Rear_Right_pulse_malfunction/1 -> Gain58/1
  SWINve_y_Front_Left_pulse_malfunction/1 -> Gain55/1
  Gain60/1 -> Data Type Conversion124/1, IMAPve_g_ESC_FR_WhlSpd/1  "IMAPve_g_ESC_FR_WhlSpd"
  SWINve_g_No_filtered_front_right_speed/1 -> Gain60/1
  Gain61/1 -> Data Type Conversion125/1, IMAPve_g_ESC_RL_WhlSpd/1  "IMAPve_g_ESC_RL_WhlSpd"
  SWINve_g_No_filtered_rear_left_speed/1 -> Gain61/1
  Gain62/1 -> Data Type Conversion126/1, IMAPve_g_ESC_RR_WhlSpd/1  "IMAPve_g_ESC_RR_WhlSpd"
  SWINve_g_No_filtered_rear_rignt_speed/1 -> Gain62/1
  SWINve_g_Pulse_counter_rearright_wheel/1 -> Gain66/1
  SWINve_g_Pulse_counter_rearleft_wheel/1 -> Gain65/1
  SWINve_y_TCU_ATFailure/1 -> Gain67/1
  SWINve_g_Pulse_counter_front_left_wheel/1 -> Gain63/1
  Gain63/1 -> Data Type Conversion127/1, IMAPve_d_ESC_FL_Wheel_Pulse/1  "IMAPve_d_ESC_FL_Wheel_Pulse"
  SWINve_g_Pulse_counter_front_right_wheel/1 -> Gain64/1
  Gain64/1 -> Data Type Conversion128/1, IMAPve_d_ESC_FR_Wheel_Pulse/1  "IMAPve_d_ESC_FR_Wheel_Pulse"
  Gain65/1 -> Data Type Conversion129/1, IMAPve_d_ESC_RL_Wheel_Pulse/1  "IMAPve_d_ESC_RL_Wheel_Pulse"
  Gain66/1 -> Data Type Conversion130/1, IMAPve_d_ESC_RR_Wheel_Pulse/1  "IMAPve_d_ESC_RR_Wheel_Pulse"
  Gain67/1 -> Data Type Conversion96/1, IMAPve_d_TCU_AT_Failure/1  "IMAPve_d_TCU_AT_Failure"
  Gain71/1 -> Data Type Conversion89/1, IMAPve_d_EMS_Engine_Status/1  "IMAPve_d_EMS_Engine_Status"
  Data Type Conversion437/1 -> Data Type Conversion98/1, IMAPve_d_TCU_Gear_Engage/1
  Data Type Conversion435/1 -> Data Type Conversion97/1, IMAPve_d_TCU_DCT_Clutch_State/1
  Data Type Conversion436/1 -> Data Type Conversion99/1, IMAPve_d_TCU_Select_ATMode/1
  Data Type Conversion332/1 -> Data Type Conversion56/1, IMAPve_d_BCM_BrakeLamp_State/1
  Data Type Conversion14/1 -> Data Type Conversion57/1, IMAPve_d_GW_Brake_Only_Req/1
  Gain78/1 -> Data Type Conversion54/1, IMAPve_d_BCM_FrontWiper_State/1  "IMAPve_d_BCM_FrontWiper_State"
  Gain77/1 -> Data Type Conversion91/1, IMAPve_d_EMS_ACC_Effective/1  "IMAPve_d_EMS_ACC_Effective"
  SWINve_y_BCM_State_Front_Wiper/1 -> Gain78/1
  SWINve_y_EMS_ACC_Effecitive_EMS/1 -> Gain77/1
  Data Type Conversion333/1 -> Data Type Conversion55/1, IMAPve_d_BCM_CHMSL_Status/1
  SWINve_y_EMS_ACCcontrol_Available/1 -> Gain81/1
  Gain81/1 -> Data Type Conversion92/1, IMAPve_d_EMS_ACC_CtlAvail/1  "IMAPve_d_EMS_ACC_CtlAvail"
  Data Type Conversion424/1 -> Data Type Conversion93/1, IMAPve_d_EMS_ACC_Inhibited/1
  SWINve_y_IC_passengerBeltSwitchSig/1 -> Gain75/1
  SWINve_y_Brake_secondary_contact/1 -> Gain83/1
  Gain83/1 -> Data Type Conversion94/1, IMAPve_d_EMS_Brake_Pedal/1  "IMAPve_d_EMS_Brake_Pedal"
  Gain290/1 -> Data Type Conversion134/1, IMAPve_d_EPB_Status/1  "IMAPve_d_EPB_Status"
  SWINve_y_Park_brake_function_status/1 -> Gain290/1
  SWINve_y_High_beam_state/1 -> Gain85/1
  Gain87/1 -> Data Type Conversion136/1, IMAPve_d_ESC_Hold_State/1  "IMAPve_d_ESC_Hold_State"
  SWINve_y_Vehicle_Hold_Status/1 -> Gain87/1
  Data Type Conversion440/1 -> IMAPve_d_ESC_Drive_Direction/1, Data Type Conversion135/1
  SWINve_y_State_indicating_steer_or_not/1 -> Gain88/1
  SWINve_g_number_of_kilometer/1 -> Gain100/1
  Constant73/1 -> Gain102/1
  Gain109/1 -> Data Type Conversion201/1, IMAPve_d_TSR_Sign_Type/1  "IMAPve_d_TSR_Sign_Type"
  Gain106/1 -> Data Type Conversion316/1, IMAPve_g_R1_C2_FR_Pred/1  "IMAPve_g_R1_C2_FR_Pred"
  Gain103/1 -> Data Type Conversion204/1, IMAPve_d_Camera_Status/1  "IMAPve_d_Camera_Status"
  Gain101/1 -> Data Type Conversion202/1, IMAPve_d_Camera_Signal_Fault/1  "IMAPve_d_Camera_Signal_Fault"
  SDFAve_y_SIGN_ISA_Value/1 -> Gain108/1
  SDFAve_g_R1_FR_PRED_RANGE/1 -> Gain107/1
  Gain108/1 -> Data Type Conversion200/1, IMAPve_d_Sign_ISA_Value/1  "IMAPve_d_Sign_ISA_Value"
  message_unpack/42(IFC_State) -> Gain103/1
  Gain102/1 -> Data Type Conversion203/1, IMAPve_d_Radar_State/1, IMAPve_d_Radar_Status/1  "IMAPve_d_Radar_Status"
  SDFAve_y_CameraSignalFault/1 -> Gain101/1
  Gain107/1 -> Data Type Conversion317/1, IMAPve_g_R1_Range_FR_Pred/1  "IMAPve_g_R1_Range_FR_Pred"
  SDFAve_y_TSR_Sign_Type/1 -> Gain109/1
  SDFAve_g_R1_C2_FR_PRE_COEF/1 -> Gain106/1
  SDFAve_g_R1_C3_BACK_COEF/1 -> Gain114/1
  SDFAve_g_R1_C1_FR_PRE_COEF/1 -> Gain110/1
  SDFAve_g_R1_C0_FR_PRE_COEF/1 -> Gain105/1
  SDFAve_g_R1_C2_BACK_COEF/1 -> Gain113/1
  Gain105/1 -> Data Type Conversion314/1, IMAPve_g_R1_C0_FR_Pred/1  "IMAPve_g_R1_C0_FR_Pred"
  Gain113/1 -> Data Type Conversion311/1, IMAPve_g_R1_C2_Back/1  "IMAPve_g_R1_C2_Back"
  Gain111/1 -> Data Type Conversion309/1, IMAPve_g_R1_C0_Back/1  "IMAPve_g_R1_C0_Back"
  Gain110/1 -> Data Type Conversion315/1, IMAPve_g_R1_C1_FR_Pred/1  "IMAPve_g_R1_C1_FR_Pred"
  Gain104/1 -> Data Type Conversion313/1, IMAPve_g_R1_Range_Back/1  "IMAPve_g_R1_Range_Back"
  SDFAve_g_R1_C0_BACK_COEF/1 -> Gain111/1
  Gain114/1 -> Data Type Conversion312/1, IMAPve_g_R1_C3_Back/1  "IMAPve_g_R1_C3_Back"
  SDFAve_g_R1_C1_BACK_COEF/1 -> Gain112/1
  SDFAve_g_R1_BACK_RANGE/1 -> Gain104/1
  Gain112/1 -> Data Type Conversion310/1, IMAPve_g_R1_C1_Back/1  "IMAPve_g_R1_C1_Back"
  SDFAve_g_L1_C0_FR_PRE_COEF/1 -> Gain123/1
  SDFAve_g_L1_FR_PRED_RANGE/1 -> Gain117/1
  SDFAve_g_L1_BACK_RANGE/1 -> Gain122/1
  SDFAve_g_R0_C0_FR_PRE_COEF/1 -> Gain126/1
  SDFAve_g_L1_C0_BACK_COEF/1 -> Gain119/1
  SDFAve_g_R0_FR_PRED_RANGE/1 -> Gain118/1
  SDFAve_g_L1_C1_BACK_COEF/1 -> Gain124/1
  SDFAve_g_L1_C2_FR_PRE_COEF/1 -> Gain116/1
  SDFAve_g_R0_C1_FR_PRE_COEF/1 -> Gain127/1
  SDFAve_g_R0_BACK_RANGE/1 -> Gain125/1
  SDFAve_g_R0_C2_FR_PRE_COEF/1 -> Gain128/1
  Gain124/1 -> Data Type Conversion301/1, IMAPve_g_L1_C1_Back/1  "IMAPve_g_L1_C1_Back"
  Gain119/1 -> Data Type Conversion300/1, IMAPve_g_L1_C0_Back/1  "IMAPve_g_L1_C0_Back"
  Gain126/1 -> Data Type Conversion296/1, IMAPve_g_R0_C0_FR_Pred/1  "IMAPve_g_R0_C0_FR_Pred"
  Gain127/1 -> Data Type Conversion297/1, IMAPve_g_R0_C1_FR_Pred/1  "IMAPve_g_R0_C1_FR_Pred"
  Gain128/1 -> Data Type Conversion298/1, IMAPve_g_R0_C2_FR_Pred/1  "IMAPve_g_R0_C2_FR_Pred"
  Gain116/1 -> Data Type Conversion307/1, IMAPve_g_L1_C2_FR_Pred/1  "IMAPve_g_L1_C2_FR_Pred"
  Gain125/1 -> Data Type Conversion295/1, IMAPve_g_R0_Range_Back/1  "IMAPve_g_R0_Range_Back"
  Gain122/1 -> Data Type Conversion304/1, IMAPve_g_L1_Range_Back/1  "IMAPve_g_L1_Range_Back"
  Gain118/1 -> Data Type Conversion299/1, IMAPve_g_R0_Range_FR_Pred/1  "IMAPve_g_R0_Range_FR_Pred"
  Gain120/1 -> Data Type Conversion302/1, IMAPve_g_L1_C2_Back/1  "IMAPve_g_L1_C2_Back"
  Gain117/1 -> Data Type Conversion308/1, IMAPve_g_L1_Range_FR_Pred/1  "IMAPve_g_L1_Range_FR_Pred"
  Gain115/1 -> Data Type Conversion306/1, IMAPve_g_L1_C1_FR_Pred/1  "IMAPve_g_L1_C1_FR_Pred"
  SDFAve_g_L1_C2_BACK_COEF/1 -> Gain120/1
  Gain123/1 -> Data Type Conversion305/1, IMAPve_g_L1_C0_FR_Pred/1  "IMAPve_g_L1_C0_FR_Pred"
  SDFAve_g_L1_C3_BACK_COEF/1 -> Gain121/1
  SDFAve_g_L1_C1_FR_PRE_COEF/1 -> Gain115/1
  Gain121/1 -> Data Type Conversion303/1, IMAPve_g_L1_C3_Back/1  "IMAPve_g_L1_C3_Back"
  Gain134/1 -> Data Type Conversion291/1, IMAPve_g_R0_C0_Back/1  "IMAPve_g_R0_C0_Back"
  Gain135/1 -> Data Type Conversion292/1, IMAPve_g_R0_C1_Back/1  "IMAPve_g_R0_C1_Back"
  Gain137/1 -> Data Type Conversion294/1, IMAPve_g_R0_C3_Back/1  "IMAPve_g_R0_C3_Back"
  Gain136/1 -> Data Type Conversion293/1, IMAPve_g_R0_C2_Back/1  "IMAPve_g_R0_C2_Back"
  SDFAve_g_L0_C1_FR_PRE_COEF/1 -> Gain131/1
  Gain132/1 -> Data Type Conversion289/1, IMAPve_g_L0_C2_FR_Pred/1  "IMAPve_g_L0_C2_FR_Pred"
  Gain133/1 -> Data Type Conversion290/1, IMAPve_g_L0_Range_FR_Pred/1  "IMAPve_g_L0_Range_FR_Pred"
  Gain129/1 -> Data Type Conversion286/1, IMAPve_g_L0_Range_Back/1  "IMAPve_g_L0_Range_Back"
  Gain130/1 -> Data Type Conversion287/1, IMAPve_g_L0_C0_FR_Pred/1  "IMAPve_g_L0_C0_FR_Pred"
  SDFAve_g_L0_BACK_RANGE/1 -> Gain129/1
  SDFAve_g_L0_C2_FR_PRE_COEF/1 -> Gain132/1
  SDFAve_g_R0_C3_BACK_COEF/1 -> Gain137/1
  SDFAve_g_L0_FR_PRED_RANGE/1 -> Gain133/1
  SDFAve_g_R0_C1_BACK_COEF/1 -> Gain135/1
  SDFAve_g_R0_C0_BACK_COEF/1 -> Gain134/1
  SDFAve_g_L0_C0_FR_PRE_COEF/1 -> Gain130/1
  SDFAve_g_R0_C2_BACK_COEF/1 -> Gain136/1
  Gain131/1 -> Data Type Conversion288/1, IMAPve_g_L0_C1_FR_Pred/1  "IMAPve_g_L0_C1_FR_Pred"
  Gain143/1 -> Data Type Conversion282/1, IMAPve_g_L0_C0_Back/1  "IMAPve_g_L0_C0_Back"
  Gain144/1 -> Data Type Conversion283/1, IMAPve_g_L0_C1_Back/1  "IMAPve_g_L0_C1_Back"
  Gain146/1 -> Data Type Conversion285/1, IMAPve_g_L0_C3_Back/1  "IMAPve_g_L0_C3_Back"
  Gain145/1 -> Data Type Conversion284/1, IMAPve_g_L0_C2_Back/1  "IMAPve_g_L0_C2_Back"
  SDFAve_g_R1_MARK_WIDTH/1 -> Gain140/1
  Gain141/1 -> Data Type Conversion280/1, IMAPve_g_R1_TLC/1  "IMAPve_g_R1_TLC"
  Gain142/1 -> Data Type Conversion281/1, IMAPve_d_R1_LC/1  "IMAPve_d_R1_LC"
  Gain138/1 -> Data Type Conversion277/1, IMAPve_d_R1_Type/1  "IMAPve_d_R1_Type"
  Gain139/1 -> Data Type Conversion278/1, IMAPve_g_R1_Confidence/1  "IMAPve_g_R1_Confidence"
  SDFAve_d_R1_LINE_TYPE/1 -> Gain138/1
  SDFAve_g_R1_TLC/1 -> Gain141/1
  SDFAve_g_L0_C3_BACK_COEF/1 -> Gain146/1
  SDFAve_y_R1_LANE_CHANGE/1 -> Gain142/1
  SDFAve_g_L0_C1_BACK_COEF/1 -> Gain144/1
  SDFAve_g_L0_C0_BACK_COEF/1 -> Gain143/1
  SDFAve_g_R1_LINE_COFIDENCE/1 -> Gain139/1
  SDFAve_g_L0_C2_BACK_COEF/1 -> Gain145/1
  Gain140/1 -> Data Type Conversion279/1, IMAPve_g_R1_W/1  "IMAPve_g_R1_W"
  Gain152/1 -> Data Type Conversion273/1, IMAPve_g_R1_C2/1  "IMAPve_g_R1_C2"
  Gain153/1 -> Data Type Conversion274/1, IMAPve_g_R1_C3/1  "IMAPve_g_R1_C3"
  Gain155/1 -> Data Type Conversion276/1, IMAPve_d_R1_Q/1  "IMAPve_d_R1_Q"
  Gain154/1 -> Data Type Conversion275/1, IMAPve_g_R1_VR/1  "IMAPve_g_R1_VR"
  SDFAve_y_L1_LANE_CHANGE/1 -> Gain149/1
  Gain150/1 -> Data Type Conversion271/1, IMAPve_g_R1_C0/1  "IMAPve_g_R1_C0"
  Gain151/1 -> Data Type Conversion272/1, IMAPve_g_R1_C1/1  "IMAPve_g_R1_C1"
  Gain147/1 -> Data Type Conversion268/1, IMAPve_g_L1_W/1  "IMAPve_g_L1_W"
  Gain148/1 -> Data Type Conversion269/1, IMAPve_g_L1_TLC/1  "IMAPve_g_L1_TLC"
  SDFAve_g_L1_MARK_WIDTH/1 -> Gain147/1
  SDFAve_g_R1_C0_COEF/1 -> Gain150/1
  SDFAve_y_R1_DETECT_QUALITY/1 -> Gain155/1
  SDFAve_g_R1_C1_COEF/1 -> Gain151/1
  SDFAve_g_R1_C3_COEF/1 -> Gain153/1
  SDFAve_g_R1_C2_COEF/1 -> Gain152/1
  SDFAve_g_L1_TLC/1 -> Gain148/1
  SDFAve_g_R1_VIEW_RANGE/1 -> Gain154/1
  Gain149/1 -> Data Type Conversion270/1, IMAPve_d_L1_LC/1  "IMAPve_d_L1_LC"
  Gain161/1 -> Data Type Conversion264/1, IMAPve_g_L1_VR/1  "IMAPve_g_L1_VR"
  Gain162/1 -> Data Type Conversion265/1, IMAPve_d_L1_Q/1  "IMAPve_d_L1_Q"
  Gain164/1 -> Data Type Conversion267/1, IMAPve_g_L1_Confidence/1  "IMAPve_g_L1_Confidence"
  Gain163/1 -> Data Type Conversion266/1, IMAPve_d_L1_Type/1  "IMAPve_d_L1_Type"
  SDFAve_g_L1_C1_COEF/1 -> Gain158/1
  Gain159/1 -> Data Type Conversion262/1, IMAPve_g_L1_C2/1  "IMAPve_g_L1_C2"
  Gain160/1 -> Data Type Conversion263/1, IMAPve_g_L1_C3/1  "IMAPve_g_L1_C3"
  Gain156/1 -> Data Type Conversion259/1, IMAPve_d_R0_LC/1  "IMAPve_d_R0_LC"
  Gain157/1 -> Data Type Conversion260/1, IMAPve_g_L1_C0/1  "IMAPve_g_L1_C0"
  SDFAve_y_R0_LANE_CHANGE/1 -> Gain156/1
  SDFAve_g_L1_C2_COEF/1 -> Gain159/1
  SDFAve_g_L1_LINE_COFIDENCE/1 -> Gain164/1
  SDFAve_g_L1_C3_COEF/1 -> Gain160/1
  SDFAve_y_L1_DETECT_QUALITY/1 -> Gain162/1
  SDFAve_g_L1_VIEW_RANGE/1 -> Gain161/1
  SDFAve_g_L1_C0_COEF/1 -> Gain157/1
  SDFAve_d_L1_LINE_TYPE/1 -> Gain163/1
  Gain158/1 -> Data Type Conversion261/1, IMAPve_g_L1_C1/1  "IMAPve_g_L1_C1"
  Gain170/1 -> Data Type Conversion255/1, IMAPve_d_R0_Type/1  "IMAPve_d_R0_Type"
  Gain171/1 -> Data Type Conversion256/1, IMAPve_g_R0_Confidence/1  "IMAPve_g_R0_Confidence"
  Gain173/1 -> Data Type Conversion258/1, IMAPve_g_R0_TLC/1  "IMAPve_g_R0_TLC"
  Gain172/1 -> Data Type Conversion257/1, IMAPve_g_R0_W/1  "IMAPve_g_R0_W"
  SDFAve_g_R0_C3_COEF/1 -> Gain167/1
  Gain168/1 -> Data Type Conversion253/1, IMAPve_g_R0_VR/1  "IMAPve_g_R0_VR"
  Gain169/1 -> Data Type Conversion254/1, IMAPve_d_R0_Q/1  "IMAPve_d_R0_Q"
  Gain165/1 -> Data Type Conversion250/1, IMAPve_g_R0_C1/1  "IMAPve_g_R0_C1"
  Gain166/1 -> Data Type Conversion251/1, IMAPve_g_R0_C2/1  "IMAPve_g_R0_C2"
  SDFAve_g_R0_C1_COEF/1 -> Gain165/1
  SDFAve_g_R0_VIEW_RANGE/1 -> Gain168/1
  SDFAve_g_R0_TLC/1 -> Gain173/1
  SDFAve_y_R0_DETECT_QUALITY/1 -> Gain169/1
  SDFAve_g_R0_LINE_COFIDENCE/1 -> Gain171/1
  SDFAve_d_R0_LINE_TYPE/1 -> Gain170/1
  SDFAve_g_R0_C2_COEF/1 -> Gain166/1
  SDFAve_g_R0_MARK_WIDTH/1 -> Gain172/1
  Gain167/1 -> Data Type Conversion252/1, IMAPve_g_R0_C3/1  "IMAPve_g_R0_C3"
  Gain179/1 -> Data Type Conversion246/1, IMAPve_g_L0_W/1  "IMAPve_g_L0_W"
  Gain180/1 -> Data Type Conversion247/1, IMAPve_g_L0_TLC/1  "IMAPve_g_L0_TLC"
  Gain191/1 -> Data Type Conversion249/1, IMAPve_g_R0_C0/1  "IMAPve_g_R0_C0"
  Gain181/1 -> Data Type Conversion248/1, IMAPve_d_L0_LC/1  "IMAPve_d_L0_LC"
  SDFAve_y_L0_DETECT_QUALITY/1 -> Gain176/1
  Gain177/1 -> Data Type Conversion244/1, IMAPve_d_L0_Type/1  "IMAPve_d_L0_Type"
  Gain178/1 -> Data Type Conversion245/1, IMAPve_g_L0_Confidence/1  "IMAPve_g_L0_Confidence"
  Gain174/1 -> Data Type Conversion241/1, IMAPve_g_L0_C3/1  "IMAPve_g_L0_C3"
  Gain175/1 -> Data Type Conversion242/1, IMAPve_g_L0_VR/1  "IMAPve_g_L0_VR"
  SDFAve_g_L0_C3_COEF/1 -> Gain174/1
  SDFAve_d_L0_LINE_TYPE/1 -> Gain177/1
  SDFAve_g_R0_C0_COEF/1 -> Gain191/1
  SDFAve_g_L0_LINE_COFIDENCE/1 -> Gain178/1
  SDFAve_g_L0_TLC/1 -> Gain180/1
  SDFAve_g_L0_MARK_WIDTH/1 -> Gain179/1
  SDFAve_g_L0_VIEW_RANGE/1 -> Gain175/1
  SDFAve_y_L0_LANE_CHANGE/1 -> Gain181/1
  Gain176/1 -> Data Type Conversion243/1, IMAPve_d_L0_Q/1  "IMAPve_d_L0_Q"
  Gain197/1 -> Data Type Conversion237/1, IMAPve_d_ConsArea/1  "IMAPve_d_ConsArea"
  Gain198/1 -> Data Type Conversion238/1, IMAPve_g_L0_C0/1  "IMAPve_g_L0_C0"
  Gain200/1 -> Data Type Conversion240/1, IMAPve_g_L0_C2/1  "IMAPve_g_L0_C2"
  Gain199/1 -> Data Type Conversion239/1, IMAPve_g_L0_C1/1  "IMAPve_g_L0_C1"
  Gain195/1 -> Data Type Conversion235/1, IMAPve_d_Lane_Valid/1  "IMAPve_d_Lane_Valid"
  Gain196/1 -> Data Type Conversion236/1, IMAPve_d_Road_Type/1  "IMAPve_d_Road_Type"
  SDFAve_y_LANE_DETECT_ACTIV/1 -> Gain195/1
  SDFAve_g_L0_C2_COEF/1 -> Gain200/1
  SDFAve_y_ROAD_TYPE/1 -> Gain196/1
  SDFAve_g_L0_C0_COEF/1 -> Gain198/1
  SDFAve_y_CONSTRUCTION_AREA/1 -> Gain197/1
  SDFAve_g_L0_C1_COEF/1 -> Gain199/1
  Gain206/1 -> Data Type Conversion230/1, IMAPva_d_obj_MotionStatus/1  "IMAPva_d_obj_MotionStatus"
  SDFAva_d_obj_age/1 -> Gain203/1
  Gain204/1 -> Data Type Conversion228/1, IMAPva_d_obj_TurnLight/1  "IMAPva_d_obj_TurnLight"
  Gain205/1 -> Data Type Conversion229/1, IMAPva_d_obj_BrakeLight/1  "IMAPva_d_obj_BrakeLight"
  SDFAva_y_obj_TurnLight/1 -> Gain204/1
  SDFAva_y_obj_BrakeLight/1 -> Gain205/1
  SDFAva_y_obj_MotionStatus/1 -> Gain206/1
  Gain203/1 -> Data Type Conversion227/1, IMAPva_d_obj_age/1  "IMAPva_d_obj_age"
  Gain216/1 -> Data Type Conversion222/1, IMAPva_d_obj_class/1  "IMAPva_d_obj_class"
  Gain218/1 -> Data Type Conversion224/1, IMAPva_d_obj_status/1  "IMAPva_d_obj_status"
  Gain217/1 -> Data Type Conversion223/1, IMAPva_d_obj_lane/1  "IMAPva_d_obj_lane"
  Gain213/1 -> Data Type Conversion219/1, IMAPva_g_obj_width/1  "IMAPva_g_obj_width"
  Gain214/1 -> Data Type Conversion220/1, IMAPva_g_obj_length/1  "IMAPva_g_obj_length"
  SDFAva_g_obj_width/1 -> Gain213/1
  SDFAva_y_obj_status/1 -> Gain218/1
  SDFAva_g_obj_length/1 -> Gain214/1
  SDFAva_y_obj_class/1 -> Gain216/1
  SDFAva_y_obj_lane/1 -> Gain217/1
  Gain224/1 -> Data Type Conversion212/1, IMAPva_g_obj_acc_y/1  "IMAPva_g_obj_acc_y"
  Gain225/1 -> Data Type Conversion213/1, IMAPva_g_obj_pos_var_x/1  "IMAPva_g_obj_pos_var_x"
  Gain227/1 -> Data Type Conversion215/1, IMAPva_g_obj_pos_var_xy/1  "IMAPva_g_obj_pos_var_xy"
  Gain226/1 -> Data Type Conversion214/1, IMAPva_g_obj_pos_var_y/1  "IMAPva_g_obj_pos_var_y"
  SDFAva_g_obj_vel_x/1 -> Gain221/1
  Gain222/1 -> Data Type Conversion210/1, IMAPva_g_obj_vel_y/1  "IMAPva_g_obj_vel_y"
  Gain223/1 -> Data Type Conversion211/1, IMAPva_g_obj_acc_x/1  "IMAPva_g_obj_acc_x"
  Gain219/1 -> Data Type Conversion207/1, IMAPva_g_obj_pos_x/1  "IMAPva_g_obj_pos_x"
  Gain220/1 -> Data Type Conversion208/1, IMAPva_g_obj_pos_y/1  "IMAPva_g_obj_pos_y"
  SDFAva_g_obj_pos_x/1 -> Gain219/1
  SDFAva_g_obj_vel_y/1 -> Gain222/1
  SDFAva_g_obj_pos_var_xy/1 -> Gain227/1
  SDFAva_g_obj_acc_x/1 -> Gain223/1
  SDFAva_g_obj_pos_var_x/1 -> Gain225/1
  SDFAva_g_obj_acc_y/1 -> Gain224/1
  SDFAva_g_obj_pos_y/1 -> Gain220/1
  SDFAva_g_obj_pos_var_y/1 -> Gain226/1
  Gain221/1 -> Data Type Conversion209/1, IMAPva_g_obj_vel_x/1  "IMAPva_g_obj_vel_x"
  Gain233/1 -> Data Type Conversion198/1, IMAPve_d_Fusion_Status/1  "IMAPve_d_Fusion_Status"
  Gain234/1 -> Data Type Conversion199/1, IMAPve_g_Fusion_Time_Stamp/1  "IMAPve_g_Fusion_Time_Stamp"
  Gain236/1 -> Data Type Conversion206/1, IMAPva_d_obj_id/1  "IMAPva_d_obj_id"
  Gain235/1 -> Data Type Conversion205/1, IMAPve_d_obj_Num/1  "IMAPve_d_obj_Num"
  SDFAve_d_sen_sta_RF_radar/1 -> Gain230/1
  Gain231/1 -> Data Type Conversion196/1, IMAPve_d_LR_Radar_Status/1  "IMAPve_d_LR_Radar_Status"
  Gain232/1 -> Data Type Conversion197/1, IMAPve_d_RR_Radar_Status/1  "IMAPve_d_RR_Radar_Status"
  Gain228/1 -> Data Type Conversion193/1, IMAPve_d_Sensor_Status/1  "IMAPve_d_Sensor_Status"
  Gain229/1 -> Data Type Conversion194/1, IMAPve_d_LF_Radar_Status/1  "IMAPve_d_LF_Radar_Status"
  SDFAve_d_sensor_status/1 -> Gain228/1
  SDFAve_d_sen_sta_LB_radar/1 -> Gain231/1
  SDFAva_y_obj_id/1 -> Gain236/1
  SDFAve_d_sen_sta_RB_radar/1 -> Gain232/1
  SDFAve_g_fusion_time_stamp/1 -> Gain234/1
  SDFAve_d_fusion_status/1 -> Gain233/1
  SDFAve_d_sen_sta_LF_radar/1 -> Gain229/1
  SDFAve_d_obj_Num/1 -> Gain235/1
  Gain230/1 -> Data Type Conversion195/1, IMAPve_d_RF_Radar_Status/1  "IMAPve_d_RF_Radar_Status"
  Gain242/1 -> Data Type Conversion190/1, IMAPve_g_ORI_R1_VR/1  "IMAPve_g_ORI_R1_VR"
  Gain243/1 -> IMAPve_g_ORI_R1_TLC/1, Data Type Conversion191/1  "IMAPve_g_ORI_R1_TLC"
  Gain244/1 -> Data Type Conversion192/1, IMAPve_g_ORI_R1_W/1  "IMAPve_g_ORI_R1_W"
  Gain240/1 -> Data Type Conversion188/1, IMAPve_d_ORI_R1_Q/1  "IMAPve_d_ORI_R1_Q"
  Gain241/1 -> Data Type Conversion189/1, IMAPve_d_ORI_R1_LT/1  "IMAPve_d_ORI_R1_LT"
  Gain237/1 -> Data Type Conversion185/1, IMAPve_g_ORI_R1_C2/1  "IMAPve_g_ORI_R1_C2"
  Gain238/1 -> Data Type Conversion186/1, IMAPve_g_ORI_R1_C1/1  "IMAPve_g_ORI_R1_C1"
  message_unpack/146(IFC_Line04_Curv) -> Gain237/1
  Constant71/1 -> Gain240/1
  Constant72/1 -> Gain245/1
  message_unpack/149(IFC_Line04_Type) -> Gain241/1
  Constant74/1 -> Gain243/1
  message_unpack/142(IFC_Line04_DxEnd) -> Gain242/1
  message_unpack/143(IFC_Line04_HeadingAngle) -> Gain238/1
  message_unpack/148(IFC_Line04_LineWidth) -> Gain244/1
  Gain239/1 -> Data Type Conversion187/1, IMAPve_g_ORI_R1_C0/1  "IMAPve_g_ORI_R1_C0"
  Gain251/1 -> Data Type Conversion181/1, IMAPve_g_ORI_R0_TLC/1  "IMAPve_g_ORI_R0_TLC"
  Gain252/1 -> Data Type Conversion182/1, IMAPve_g_ORI_R0_W/1  "IMAPve_g_ORI_R0_W"
  Gain254/1 -> Data Type Conversion184/1, IMAPve_g_ORI_R1_C3/1  "IMAPve_g_ORI_R1_C3"
  Gain253/1 -> Data Type Conversion183/1, IMAPve_d_ORI_R0_LC/1  "IMAPve_d_ORI_R0_LC"
  Constant54/1 -> Gain248/1
  Gain249/1 -> Data Type Conversion179/1, IMAPve_d_ORI_R0_LT/1  "IMAPve_d_ORI_R0_LT"
  Gain250/1 -> Data Type Conversion180/1, IMAPve_g_ORI_R0_VR/1  "IMAPve_g_ORI_R0_VR"
  Gain246/1 -> Data Type Conversion176/1, IMAPve_g_ORI_R0_C1/1  "IMAPve_g_ORI_R0_C1"
  Gain247/1 -> Data Type Conversion177/1, IMAPve_g_ORI_R0_C0/1  "IMAPve_g_ORI_R0_C0"
  message_unpack/117(IFC_Line02_HeadingAngle) -> Gain246/1
  message_unpack/123(IFC_Line02_Type) -> Gain249/1
  message_unpack/145(IFC_Line04_CurvChange) -> Gain254/1
  message_unpack/116(IFC_Line02_DxEnd) -> Gain250/1
  message_unpack/122(IFC_Line02_LineWidth) -> Gain252/1
  Constant59/1 -> Gain251/1
  message_unpack/118(IFC_Line02_Dy) -> Gain247/1
  Constant66/1 -> Gain253/1
  Gain248/1 -> Data Type Conversion178/1, IMAPve_d_ORI_R0_Q/1  "IMAPve_d_ORI_R0_Q"
  Gain260/1 -> Data Type Conversion174/1, IMAPve_g_ORI_R0_C3/1  "IMAPve_g_ORI_R0_C3"
  Gain261/1 -> Data Type Conversion175/1, IMAPve_g_ORI_R0_C2/1  "IMAPve_g_ORI_R0_C2"
  Constant51/1 -> Gain257/1
  Gain258/1 -> Data Type Conversion172/1, IMAPve_g_ORI_L1_W/1  "IMAPve_g_ORI_L1_W"
  Gain256/1 -> Data Type Conversion170/1, IMAPve_g_ORI_L1_VR/1  "IMAPve_g_ORI_L1_VR"
  Gain255/1 -> Data Type Conversion169/1, IMAPve_d_ORI_L1_Type/1  "IMAPve_d_ORI_L1_Type"
  Gain257/1 -> Data Type Conversion171/1, IMAPve_g_ORI_L1_TLC/1  "IMAPve_g_ORI_L1_TLC"
  Constant49/1 -> Gain259/1
  message_unpack/136(IFC_Line03_Type) -> Gain255/1
  message_unpack/135(IFC_Line03_LineWidth) -> Gain258/1
  message_unpack/120(IFC_Line02_Curv) -> Gain261/1
  message_unpack/119(IFC_Line02_CurvChange) -> Gain260/1
  message_unpack/129(IFC_Line03_DxEnd) -> Gain256/1
  Gain259/1 -> Data Type Conversion173/1, IMAPve_d_ORI_L1_LC/1  "IMAPve_d_ORI_L1_LC"
  Gain267/1 -> Data Type Conversion167/1, IMAPve_g_ORI_L1_C0/1  "IMAPve_g_ORI_L1_C0"
  Gain268/1 -> IMAPve_d_ORI_L1_Q/1, Data Type Conversion168/1  "IMAPve_d_ORI_L1_Q"
  message_unpack/132(IFC_Line03_CurvChange) -> Gain264/1
  Gain265/1 -> Data Type Conversion165/1, IMAPve_g_ORI_L1_C2/1  "IMAPve_g_ORI_L1_C2"
  Gain263/1 -> Data Type Conversion163/1, IMAPve_d_ORI_L0_LC/1  "IMAPve_d_ORI_L0_LC"
  Gain262/1 -> Data Type Conversion162/1, IMAPve_g_ORI_L0_W/1  "IMAPve_g_ORI_L0_W"
  Gain264/1 -> Data Type Conversion164/1, IMAPve_g_ORI_L1_C3/1  "IMAPve_g_ORI_L1_C3"
  message_unpack/130(IFC_Line03_HeadingAngle) -> Gain266/1
  message_unpack/109(IFC_Line01_LineWidth) -> Gain262/1
  message_unpack/133(IFC_Line03_Curv) -> Gain265/1
  Constant48/1 -> Gain268/1
  message_unpack/131(IFC_Line03_Dy) -> Gain267/1
  Constant43/1 -> Gain263/1
  Gain266/1 -> Data Type Conversion166/1, IMAPve_g_ORI_L1_C1/1  "IMAPve_g_ORI_L1_C1"
  Gain274/1 -> Data Type Conversion160/1, IMAPve_g_ORI_L0_VR/1  "IMAPve_g_ORI_L0_VR"
  Gain275/1 -> Data Type Conversion161/1, IMAPve_g_ORI_L0_TLC/1  "IMAPve_g_ORI_L0_TLC"
  message_unpack/105(IFC_Line01_Dy) -> Gain271/1
  Gain272/1 -> Data Type Conversion158/1, IMAPve_d_ORI_L0_Q/1  "IMAPve_d_ORI_L0_Q"
  Gain270/1 -> Data Type Conversion156/1, IMAPve_g_ORI_L0_C1/1  "IMAPve_g_ORI_L0_C1"
  Gain269/1 -> IMAPve_g_ORI_L0_C2/1, Data Type Conversion155/1  "IMAPve_g_ORI_L0_C2"
  Gain271/1 -> Data Type Conversion157/1, IMAPve_g_ORI_L0_C0/1  "IMAPve_g_ORI_L0_C0"
  message_unpack/110(IFC_Line01_Type) -> Gain273/1
  message_unpack/107(IFC_Line01_Curv) -> Gain269/1
  Constant34/1 -> Gain272/1
  Constant37/1 -> Gain275/1
  message_unpack/103(IFC_Line01_DxEnd) -> Gain274/1
  message_unpack/104(IFC_Line01_HeadingAngle) -> Gain270/1
  Gain273/1 -> Data Type Conversion159/1, IMAPve_d_ORI_L0_Type/1  "IMAPve_d_ORI_L0_Type"
  Constant29/1 -> Gain276/1
  message_unpack/106(IFC_Line01_CurvChange) -> Gain277/1
  Gain277/1 -> Data Type Conversion154/1, IMAPve_g_ORI_L0_C3/1  "IMAPve_g_ORI_L0_C3"
  Gain276/1 -> Data Type Conversion153/1, IMAPve_d_ORI_Lane_RoadType/1  "IMAPve_d_ORI_Lane_RoadType"
  SWINve_g_EMS_Acceleration_pedal_position/1 -> Gain278/1
  Gain278/1 -> Data Type Conversion78/1, IMAPve_g_EMS_RealPedal/1  "IMAPve_g_EMS_RealPedal"
  Constant58/1 -> Data Type Conversion372/1
  Constant57/1 -> Data Type Conversion402/1
  Data Type Conversion15/1 -> Data Type Conversion66/1, IMAPve_d_EPS_Error_State/1
  SWINve_g_Steering_wheel_angle/1 -> Gain281/1
  SWINve_g_EMS_Actual_torque/1 -> Gain283/1
  Gain283/1 -> Data Type Conversion83/1, IMAPve_g_EMS_Actual_FlwT/1  "IMAPve_g_EMS_Actual_FlwT"
  Data Type Conversion336/1 -> Data Type Conversion84/1, IMAPve_g_EMS_Realize_TWhl/1
  Data Type Conversion337/1 -> Data Type Conversion85/1, IMAPve_g_EMS_ACC_VirtualPedal/1
  System_Clock/1 -> Gain287/1
  array_transfer11/1(output) -> Data Type Conversion/1
  Data Type Conversion339/1 -> Data Type Conversion90/1, IMAPve_d_EMS_Gearbox_CtlAvail/1
  Data Type Conversion433/1 -> Data Type Conversion131/1, IMAPve_d_ESC_Brake_Failsafe/1
  array_transfer10/1(output) -> Data Type Conversion8/1
  Constant61/1 -> Data Type Conversion373/1
  SWINve_y_EMS_Engine_state/1 -> Gain71/1
  Constant17/1 -> array_transfer/1(input)
  message_unpack/59(IFC_obj_Rel_Vx) -> Gain6/1
  message_unpack/61(IFC_obj_Dx) -> Gain7/1
  Constant22/1 -> array_transfer3/1(input)
  message_unpack/80(IFC_obj_PhiLeft) -> Gain9/1
  message_unpack/81(IFC_obj_PhiRight) -> Gain10/1
  message_unpack/75(IFC_obj_Width) -> Gain11/1
  message_unpack/94(IFC_obj_Type) -> Gain4/1
  Constant23/1 -> array_transfer8/1(input)
  message_unpack/95(IFC_obj_ID) -> Gain12/1
  Data Type Conversion34/1 -> Terminator24/1  "ob_IMAPve_d_LKA_Main_Switch"
  Data Type Conversion35/1 -> Terminator25/1  "ob_IMAPve_d_LKA_Mode"
  Gain183/1 -> Data Type Conversion35/1, IMAPve_d_LKA_Mode/1  "IMAPve_d_LKA_Mode"
  Gain184/1 -> Data Type Conversion36/1, IMAPve_d_AEB_Switch/1  "IMAPve_d_AEB_Switch"
  Data Type Conversion36/1 -> Terminator27/1  "ob_IMAPve_d_AEB_Switch"
  Data Type Conversion39/1 -> Terminator30/1  "ob_IMAPve_d_ISA_Switch"
  Gain185/1 -> Data Type Conversion37/1, IMAPve_d_FCW_Switch/1  "IMAPve_d_FCW_Switch"
  Gain187/1 -> Data Type Conversion39/1, IMAPve_d_ISA_Switch/1  "IMAPve_d_ISA_Switch"
  Gain186/1 -> Data Type Conversion38/1, IMAPve_d_FCW_Sensitivity/1  "IMAPve_d_FCW_Sensitivity"
  Data Type Conversion38/1 -> Terminator29/1  "ob_IMAPve_d_FCW_Sensitivity"
  Data Type Conversion37/1 -> Terminator28/1  "ob_IMAPve_d_FCW_Switch"
  Data Type Conversion40/1 -> Terminator31/1  "ob_IMAPve_d_TSR_Switch"
  Gain188/1 -> Data Type Conversion40/1, IMAPve_d_TSR_Switch/1  "IMAPve_d_TSR_Switch"
  Data Type Conversion16/1 -> Data Type Conversion41/1, IMAPve_d_Speed_Limit_Switch/1
  Data Type Conversion41/1 -> Terminator32/1  "ob_IMAPve_d_Speed_Limit_Switch"
  Data Type Conversion44/1 -> Terminator35/1  "ob_IMAPve_d_BCM_LF_Door_State"
  Gain76/1 -> array_transfer11/2(LF_Door), Data Type Conversion44/1, IMAPve_d_BCM_LF_Door_State/1  "IMAPve_d_BCM_LF_Door_State"
  Data Type Conversion46/1 -> Terminator37/1  "ob_IMAPve_d_BCM_RR_Door_State"
  Data Type Conversion47/1 -> Terminator38/1  "ob_IMAPve_d_BCM_LR_Door_State"
  Data Type Conversion/1 -> Data Type Conversion42/1, IMAPve_d_BCM_Opening_State/1
  Gain53/1 -> array_transfer11/1(Trunk_State), Data Type Conversion43/1, IMAPve_d_BCM_Trunk_State/1  "IMAPve_d_BCM_Trunk_State"
  Gain289/1 -> Data Type Conversion46/1, IMAPve_d_BCM_RR_Door_State/1, array_transfer11/4(RR_Door)  "IMAPve_d_BCM_RR_Door_State"
  Data Type Conversion43/1 -> Terminator34/1  "ob_IMAPve_d_BCM_Trunk_State"
  Data Type Conversion42/1 -> Terminator33/1  "ob_IMAPve_d_BCM_Opening_State"
  Data Type Conversion45/1 -> Terminator36/1  "ob_IMAPve_d_BCM_RF_Door_State"
  Gain353/1 -> array_transfer11/5(LR_Door), Data Type Conversion47/1, IMAPve_d_BCM_LR_Door_State/1  "IMAPve_d_BCM_LR_Door_State"
  Gain279/1 -> array_transfer11/3(RF_Door), Data Type Conversion45/1, IMAPve_d_BCM_RF_Door_State/1  "IMAPve_d_BCM_RF_Door_State"
  Gain48/1 -> IMAPve_d_BCM_Right_Light/1, Data Type Conversion51/1, array_transfer10/2(Right_Light)  "IMAPve_d_BCM_Right_Light"
  Data Type Conversion49/1 -> Terminator40/1  "ob_IMAPve_d_BCM_HazardLamp"
  Data Type Conversion51/1 -> Terminator42/1  "ob_IMAPve_d_BCM_Right_Light"
  Gain42/1 -> array_transfer10/1(Left_Light), Data Type Conversion50/1, IMAPve_d_BCM_Left_Light/1  "IMAPve_d_BCM_Left_Light"
  Data Type Conversion8/1 -> Data Type Conversion49/1, IMAPve_d_BCM_HazardLamp/1
  Data Type Conversion50/1 -> Terminator41/1  "ob_IMAPve_d_BCM_Left_Light"
  Gain75/1 -> Data Type Conversion58/1, IMAPve_d_ACU_Passenger_Belt/1  "IMAPve_d_ACU_Passenger_Belt"
  Data Type Conversion52/1 -> Terminator43/1  "ob_IMAPve_d_BCM_Ignition_State"
  Data Type Conversion53/1 -> Terminator44/1  "ob_IMAPve_d_ACU_Driver_Belt"
  Data Type Conversion58/1 -> Terminator49/1  "ob_IMAPve_d_ACU_Passenger_Belt"
  Data Type Conversion54/1 -> Terminator45/1  "ob_IMAPve_d_BCM_FrontWiper_State"
  Data Type Conversion55/1 -> Terminator46/1  "ob_IMAPve_d_BCM_CHMSL_Status"
  Data Type Conversion57/1 -> Terminator48/1  "ob_IMAPve_d_GW_Brake_Only_Req"
  Data Type Conversion56/1 -> Terminator47/1  "ob_IMAPve_d_BCM_BrakeLamp_State"
  Data Type Conversion432/1 -> Data Type Conversion59/1, IMAPve_d_SCC_Right_SwitchSig/1
  Data Type Conversion59/1 -> Terminator50/1  "ob_IMAPve_d_SCC_Right_SwitchSig"
  Gain287/1 -> Data Type Conversion61/1, IMAPve_d_Time_System_Clock/1  "IMAPve_d_Time_System_Clock"
  Data Type Conversion60/1 -> Terminator51/1  "ob_IMAPve_d_BCM_HighBeam_State"
  Data Type Conversion61/1 -> Terminator52/1  "ob_IMAPve_d_Time_System_Clock"
  Data Type Conversion13/1 -> Data Type Conversion63/1, IMAPve_g_FAPA_State/1
  Data Type Conversion62/1 -> Terminator53/1  "ob_IMAPve_g_GW_IC_Odometer"
  Data Type Conversion63/1 -> Terminator54/1  "ob_IMAPve_g_FAPA_State"
  Gain100/1 -> Data Type Conversion62/1, IMAPve_g_GW_IC_Odometer/1  "IMAPve_g_GW_IC_Odometer"
  Gain85/1 -> Data Type Conversion60/1, IMAPve_d_BCM_HighBeam_State/1  "IMAPve_d_BCM_HighBeam_State"
  Data Type Conversion65/1 -> Terminator56/1  "ob_IMAPve_g_EPS_SW_Trq"
  Data Type Conversion64/1 -> Terminator55/1  "ob_IMAPve_d_EPS_LKA_State"
  Data Type Conversion66/1 -> Terminator57/1  "ob_IMAPve_d_EPS_Error_State"
  Data Type Conversion438/1 -> Data Type Conversion69/1, IMAPve_d_EPS_TrqLim_State/1
  Data Type Conversion67/1 -> Terminator58/1  "ob_IMAPve_d_SAS_Clb_State"
  Data Type Conversion68/1 -> Terminator59/1  "ob_IMAPve_d_SAS_Trim_State"
  Gain15/1 -> Data Type Conversion67/1, IMAPve_d_SAS_Clb_State/1  "IMAPve_d_SAS_Clb_State"
  Data Type Conversion69/1 -> Terminator60/1  "ob_IMAPve_d_EPS_TrqLim_State"
  Gain16/1 -> Data Type Conversion68/1, IMAPve_d_SAS_Trim_State/1  "IMAPve_d_SAS_Trim_State"
  Gain24/1 -> Data Type Conversion71/1, IMAPve_g_SW_Angle_Speed/1  "IMAPve_g_SW_Angle_Speed"
  Data Type Conversion17/1 -> Data Type Conversion72/1, IMAPve_d_SWS_Fault_Code/1
  Gain281/1 -> Data Type Conversion70/1, IMAPve_g_SW_Angle/1  "IMAPve_g_SW_Angle"
  Data Type Conversion72/1 -> Terminator63/1  "ob_IMAPve_d_SWS_Fault_Code"
  Data Type Conversion71/1 -> Terminator62/1  "ob_IMAPve_g_SW_Angle_Speed"
  Data Type Conversion70/1 -> Terminator61/1  "ob_IMAPve_g_SW_Angle"
  Gain43/1 -> Data Type Conversion73/1, IMAPve_d_SWS_Failure_Status/1  "IMAPve_d_SWS_Failure_Status"
  Data Type Conversion74/1 -> Terminator65/1  "ob_IMAPve_d_EPS_Steer_Hold_State"
  Gain88/1 -> Data Type Conversion74/1, IMAPve_d_EPS_Steer_Hold_State/1  "IMAPve_d_EPS_Steer_Hold_State"
  Data Type Conversion73/1 -> Terminator64/1  "ob_IMAPve_d_SWS_Failure_Status"
  Data Type Conversion82/1 -> Terminator73/1  "ob_IMAPve_g_EMS_MinTWhl_Offset"
  Gain33/1 -> Data Type Conversion81/1, IMAPve_g_EMS_MinTWhl/1  "IMAPve_g_EMS_MinTWhl"
  Data Type Conversion341/1 -> Data Type Conversion82/1, IMAPve_g_EMS_MinTWhl_Offset/1
  Data Type Conversion75/1 -> Terminator66/1  "ob_IMAPve_d_EMS_ACC_Status"
  Data Type Conversion76/1 -> Terminator67/1  "ob_IMAPve_g_EMS_Pot_WhlT_Max"
  Data Type Conversion81/1 -> Terminator72/1  "ob_IMAPve_g_EMS_MinTWhl"
  Data Type Conversion77/1 -> Terminator68/1  "ob_IMAPve_g_EMS_Pot_WhlT_Min"
  Data Type Conversion78/1 -> Terminator69/1  "ob_IMAPve_g_EMS_RealPedal"
  Data Type Conversion80/1 -> Terminator71/1  "ob_IMAPve_g_EMS_MaxTWhl_Offset"
  Data Type Conversion79/1 -> Terminator70/1  "ob_IMAPve_g_EMS_MaxTWhl"
  Data Type Conversion83/1 -> Terminator74/1  "ob_IMAPve_g_EMS_Actual_FlwT"
  Data Type Conversion84/1 -> Terminator75/1  "ob_IMAPve_g_EMS_Realize_TWhl"
  Data Type Conversion85/1 -> Terminator76/1  "ob_IMAPve_g_EMS_ACC_VirtualPedal"
  Data Type Conversion86/1 -> Terminator77/1  "ob_IMAPve_g_EMS_Driver_Torque"
  Data Type Conversion88/1 -> Terminator79/1  "ob_IMAPve_d_TCU_Actual_Gear"
  Data Type Conversion87/1 -> Terminator78/1  "ob_IMAPve_g_EMS_Engine_Speed"
  Data Type Conversion89/1 -> Terminator80/1  "ob_IMAPve_d_EMS_Engine_Status"
  Data Type Conversion90/1 -> Terminator81/1  "ob_IMAPve_d_EMS_Gearbox_CtlAvail"
  Data Type Conversion91/1 -> Terminator82/1  "ob_IMAPve_d_EMS_ACC_Effective"
  Data Type Conversion92/1 -> Terminator83/1  "ob_IMAPve_d_EMS_ACC_CtlAvail"
  Data Type Conversion94/1 -> Terminator85/1  "ob_IMAPve_d_EMS_Brake_Pedal"
  Data Type Conversion93/1 -> Terminator84/1  "ob_IMAPve_d_EMS_ACC_Inhibited"
  Data Type Conversion95/1 -> Terminator86/1  "ob_IMAPve_d_TCU_Target_Gear"
  Data Type Conversion97/1 -> Terminator88/1  "ob_IMAPve_d_TCU_DCT_Clutch_State"
  Data Type Conversion98/1 -> Terminator89/1  "ob_IMAPve_d_TCU_Gear_Engage"
  Data Type Conversion96/1 -> Terminator87/1  "ob_IMAPve_d_TCU_AT_Failure"
  Data Type Conversion99/1 -> Terminator90/1  "ob_IMAPve_d_TCU_Select_ATMode"
  Data Type Conversion105/1 -> Terminator96/1  "ob_IMAPve_g_ESC_Brake_Press"
  Data Type Conversion104/1 -> Terminator95/1  "ob_IMAPve_g_ESC_LonAcc"
  Data Type Conversion101/1 -> Terminator92/1  "ob_IMAPve_g_ESC_YawRate"
  Data Type Conversion102/1 -> Terminator93/1  "ob_IMAPve_g_ESC_UnYawRate"
  Data Type Conversion100/1 -> Terminator91/1  "ob_IMAPve_g_ESC_LatAcc"
  Data Type Conversion103/1 -> Terminator94/1  "ob_IMAPve_g_ESC_VehSpd"
  Data Type Conversion106/1 -> Terminator97/1  "ob_IMAPve_g_ESC_Static_Slope"
  Data Type Conversion108/1 -> Terminator99/1  "ob_IMAPve_g_ESC_DySlope"
  Data Type Conversion109/1 -> Terminator100/1  "ob_IMAPve_d_ESC_Brake_Effort"
  Data Type Conversion107/1 -> Terminator98/1  "ob_IMAPve_g_ESC_DySlope_Accuracy"
  Data Type Conversion112/1 -> Terminator104/1  "ob_IMAPve_d_ESC_AlarmSig"
  Data Type Conversion114/1 -> Terminator101/1  "ob_IMAPve_d_ESC_MSR_Active"
  Data Type Conversion111/1 -> Terminator103/1  "ob_IMAPve_d_ESC_OFF"
  Data Type Conversion113/1 -> Terminator105/1  "ob_IMAPve_d_ESC_ESC_Active"
  Data Type Conversion110/1 -> Terminator102/1  "ob_IMAPve_d_ESC_Veh_Standstill"
  Data Type Conversion117/1 -> Terminator109/1  "ob_IMAPve_d_Brake_Pedal_Fault"
  Data Type Conversion119/1 -> Terminator106/1  "ob_IMAPve_d_ESC_FL_WheelPulVal"
  Data Type Conversion116/1 -> Terminator108/1  "ob_IMAPve_d_ESC_VehSpd_Valid"
  Data Type Conversion118/1 -> Terminator110/1  "ob_IMAPve_d_ESC_ABS_Active"
  Data Type Conversion115/1 -> Terminator107/1  "ob_IMAPve_d_ESC_TCS_Active"
  Data Type Conversion122/1 -> Terminator114/1  "ob_IMAPve_d_ESC_RR_WheelPulVal"
  Data Type Conversion124/1 -> Terminator111/1  "ob_IMAPve_g_ESC_FR_WhlSpd"
  Data Type Conversion121/1 -> Terminator113/1  "ob_IMAPve_d_ESC_RL_WheelPulVal"
  Data Type Conversion123/1 -> Terminator115/1  "ob_IMAPve_g_ESC_FL_WhlSpd"
  Data Type Conversion120/1 -> Terminator112/1  "ob_IMAPve_d_ESC_FR_WheelPulVal"
  Data Type Conversion127/1 -> Terminator119/1  "ob_IMAPve_d_ESC_FL_Wheel_Pulse"
  Data Type Conversion129/1 -> Terminator116/1  "ob_IMAPve_d_ESC_RL_Wheel_Pulse"
  Data Type Conversion126/1 -> Terminator118/1  "ob_IMAPve_g_ESC_RR_WhlSpd"
  Data Type Conversion128/1 -> Terminator120/1  "ob_IMAPve_d_ESC_FR_Wheel_Pulse"
  Data Type Conversion125/1 -> Terminator117/1  "ob_IMAPve_g_ESC_RL_WhlSpd"
  Data Type Conversion132/1 -> Terminator124/1  "ob_IMAPve_d_ESC_AEB_Status"
  Data Type Conversion134/1 -> Terminator121/1  "ob_IMAPve_d_EPB_Status"
  Data Type Conversion131/1 -> Terminator123/1  "ob_IMAPve_d_ESC_Brake_Failsafe"
  Data Type Conversion133/1 -> Terminator125/1  "ob_IMAPve_d_ESC_ACC_Status"
  Data Type Conversion130/1 -> Terminator122/1  "ob_IMAPve_d_ESC_RR_Wheel_Pulse"
  Data Type Conversion135/1 -> Terminator126/1  "ob_IMAPve_d_ESC_Drive_Direction"
  Data Type Conversion136/1 -> Terminator127/1  "ob_IMAPve_d_ESC_Hold_State"
  Data Type Conversion144/1 -> Terminator135/1  "ob_IMAPva_g_ORI_Obj_RelVel"
  Data Type Conversion143/1 -> Terminator134/1  "ob_IMAPva_d_ORI_Obj_Motion"
  Data Type Conversion141/1 -> Terminator132/1  "ob_IMAPva_g_ORI_Probability"
  Data Type Conversion139/1 -> Terminator130/1  "ob_IMAPve_d_ORI_CIPV_ID"
  Data Type Conversion142/1 -> Terminator133/1  "ob_IMAPva_d_ORI_Obj_Class"
  Data Type Conversion140/1 -> Terminator131/1  "ob_IMAPve_d_ORI_Obj_Num"
  Gain11/1 -> Data Type Conversion149/1, IMAPva_g_ORI_Obj_Width/1  "IMAPva_g_ORI_Obj_Width"
  Gain9/1 -> IMAPva_g_ORI_Obj_LAngle/1, Data Type Conversion147/1  "IMAPva_g_ORI_Obj_LAngle"
  Data Type Conversion146/1 -> Terminator137/1  "ob_IMAPva_d_ORI_Obj_Lane"
  Data Type Conversion148/1 -> Terminator139/1  "ob_IMAPva_g_ORI_Obj_RAngle"
  Data Type Conversion147/1 -> Terminator138/1  "ob_IMAPva_g_ORI_Obj_LAngle"
  Data Type Conversion149/1 -> Terminator140/1  "ob_IMAPva_g_ORI_Obj_Width"
  Gain10/1 -> Data Type Conversion148/1, IMAPva_g_ORI_Obj_RAngle/1  "IMAPva_g_ORI_Obj_RAngle"
  Data Type Conversion150/1 -> Terminator141/1  "ob_IMAPva_d_ORI_Obj_ID"
  Data Type Conversion145/1 -> Terminator136/1  "ob_IMAPva_g_ORI_Obj_LongDis"
  Data Type Conversion156/1 -> Terminator147/1  "ob_IMAPve_g_ORI_L0_C1"
  Data Type Conversion155/1 -> Terminator146/1  "ob_IMAPve_g_ORI_L0_C2"
  Data Type Conversion153/1 -> Terminator144/1  "ob_IMAPve_d_ORI_Lane_RoadType"
  Data Type Conversion151/1 -> Terminator142/1  "ob_IMAPve_d_ORI_Lane_Valid"
  Data Type Conversion154/1 -> Terminator145/1  "ob_IMAPve_g_ORI_L0_C3"
  Data Type Conversion152/1 -> Terminator143/1  "ob_IMAPve_d_ORI_Lane_ConsArea"
  Data Type Conversion162/1 -> Terminator153/1  "ob_IMAPve_g_ORI_L0_W"
  Data Type Conversion161/1 -> Terminator152/1  "ob_IMAPve_g_ORI_L0_TLC"
  Data Type Conversion159/1 -> Terminator150/1  "ob_IMAPve_d_ORI_L0_Type"
  Data Type Conversion157/1 -> Terminator148/1  "ob_IMAPve_g_ORI_L0_C0"
  Data Type Conversion160/1 -> Terminator151/1  "ob_IMAPve_g_ORI_L0_VR"
  Data Type Conversion158/1 -> Terminator149/1  "ob_IMAPve_d_ORI_L0_Q"
  Data Type Conversion168/1 -> Terminator159/1  "ob_IMAPve_d_ORI_L1_Q"
  Data Type Conversion167/1 -> Terminator158/1  "ob_IMAPve_g_ORI_L1_C0"
  Data Type Conversion165/1 -> Terminator156/1  "ob_IMAPve_g_ORI_L1_C2"
  Data Type Conversion163/1 -> Terminator154/1  "ob_IMAPve_d_ORI_L0_LC"
  Data Type Conversion166/1 -> Terminator157/1  "ob_IMAPve_g_ORI_L1_C1"
  Data Type Conversion164/1 -> Terminator155/1  "ob_IMAPve_g_ORI_L1_C3"
  Data Type Conversion174/1 -> Terminator165/1  "ob_IMAPve_g_ORI_R0_C3"
  Data Type Conversion173/1 -> Terminator164/1  "ob_IMAPve_d_ORI_L1_LC"
  Data Type Conversion171/1 -> Terminator162/1  "ob_IMAPve_g_ORI_L1_TLC"
  Data Type Conversion169/1 -> Terminator160/1  "ob_IMAPve_d_ORI_L1_Type"
  Data Type Conversion172/1 -> Terminator163/1  "ob_IMAPve_g_ORI_L1_W"
  Data Type Conversion170/1 -> Terminator161/1  "ob_IMAPve_g_ORI_L1_VR"
  Data Type Conversion180/1 -> Terminator171/1  "ob_IMAPve_g_ORI_R0_VR"
  Data Type Conversion179/1 -> Terminator170/1  "ob_IMAPve_d_ORI_R0_LT"
  Data Type Conversion177/1 -> Terminator168/1  "ob_IMAPve_g_ORI_R0_C0"
  Data Type Conversion175/1 -> Terminator166/1  "ob_IMAPve_g_ORI_R0_C2"
  Data Type Conversion178/1 -> Terminator169/1  "ob_IMAPve_d_ORI_R0_Q"
  Data Type Conversion176/1 -> Terminator167/1  "ob_IMAPve_g_ORI_R0_C1"
  Data Type Conversion186/1 -> Terminator177/1  "ob_IMAPve_g_ORI_R1_C1"
  Data Type Conversion185/1 -> Terminator176/1  "ob_IMAPve_g_ORI_R1_C2"
  Data Type Conversion183/1 -> Terminator174/1  "ob_IMAPve_d_ORI_R0_LC"
  Data Type Conversion181/1 -> Terminator172/1  "ob_IMAPve_g_ORI_R0_TLC"
  Data Type Conversion184/1 -> Terminator175/1  "ob_IMAPve_g_ORI_R1_C3"
  Data Type Conversion182/1 -> Terminator173/1  "ob_IMAPve_g_ORI_R0_W"
  Data Type Conversion192/1 -> Terminator183/1  "ob_IMAPve_g_ORI_R1_W"
  Data Type Conversion191/1 -> Terminator182/1  "ob_IMAPve_g_ORI_R1_TLC"
  Data Type Conversion189/1 -> Terminator180/1  "ob_IMAPve_d_ORI_R1_LT"
  Data Type Conversion187/1 -> Terminator178/1  "ob_IMAPve_g_ORI_R1_C0"
  Data Type Conversion190/1 -> Terminator181/1  "ob_IMAPve_g_ORI_R1_VR"
  Data Type Conversion188/1 -> Terminator179/1  "ob_IMAPve_d_ORI_R1_Q"
  Data Type Conversion198/1 -> Terminator189/1  "ob_IMAPve_d_Fusion_Status"
  Data Type Conversion197/1 -> Terminator188/1  "ob_IMAPve_d_RR_Radar_Status"
  Data Type Conversion195/1 -> Terminator186/1  "ob_IMAPve_d_RF_Radar_Status"
  Data Type Conversion193/1 -> Terminator184/1  "ob_IMAPve_d_Sensor_Status"
  Data Type Conversion196/1 -> Terminator187/1  "ob_IMAPve_d_LR_Radar_Status"
  Data Type Conversion194/1 -> Terminator185/1  "ob_IMAPve_d_LF_Radar_Status"
  Data Type Conversion204/1 -> Terminator195/1  "ob_IMAPve_d_Camera_Status"
  Data Type Conversion203/1 -> Terminator194/1  "ob_IMAPve_d_Radar_Status"
  Data Type Conversion201/1 -> Terminator192/1  "ob_IMAPve_d_TSR_Sign_Type"
  Data Type Conversion199/1 -> Terminator190/1  "ob_IMAPve_g_Fusion_Time_Stamp"
  Data Type Conversion202/1 -> Terminator193/1  "ob_IMAPve_d_Camera_Signal_Fault"
  Data Type Conversion200/1 -> Terminator191/1  "ob_IMAPve_d_Sign_ISA_Value"
  Data Type Conversion210/1 -> Terminator201/1  "ob_IMAPva_g_obj_vel_y"
  Data Type Conversion209/1 -> Terminator200/1  "ob_IMAPva_g_obj_vel_x"
  Data Type Conversion207/1 -> Terminator198/1  "ob_IMAPva_g_obj_pos_x"
  Data Type Conversion205/1 -> Terminator196/1  "ob_IMAPve_d_obj_Num"
  Data Type Conversion208/1 -> Terminator199/1  "ob_IMAPva_g_obj_pos_y"
  Data Type Conversion206/1 -> Terminator197/1  "ob_IMAPva_d_obj_id"
  Data Type Conversion215/1 -> Terminator206/1  "ob_IMAPva_g_obj_pos_var_xy"
  Data Type Conversion213/1 -> Terminator204/1  "ob_IMAPva_g_obj_pos_var_x"
  Data Type Conversion211/1 -> Terminator202/1  "ob_IMAPva_g_obj_acc_x"
  Data Type Conversion214/1 -> Terminator205/1  "ob_IMAPva_g_obj_pos_var_y"
  Data Type Conversion212/1 -> Terminator203/1  "ob_IMAPva_g_obj_acc_y"
  Data Type Conversion222/1 -> Terminator213/1  "ob_IMAPva_d_obj_class"
  Data Type Conversion219/1 -> Terminator210/1  "ob_IMAPva_g_obj_width"
  Data Type Conversion220/1 -> Terminator211/1  "ob_IMAPva_g_obj_length"
  Data Type Conversion228/1 -> Terminator219/1  "ob_IMAPva_d_obj_TurnLight"
  Data Type Conversion227/1 -> Terminator218/1  "ob_IMAPva_d_obj_age"
  Data Type Conversion223/1 -> Terminator214/1  "ob_IMAPva_d_obj_lane"
  Data Type Conversion224/1 -> Terminator215/1  "ob_IMAPva_d_obj_status"
  Data Type Conversion229/1 -> Terminator220/1  "ob_IMAPva_d_obj_BrakeLight"
  Data Type Conversion230/1 -> Terminator221/1  "ob_IMAPva_d_obj_MotionStatus"
  Data Type Conversion240/1 -> Terminator231/1  "ob_IMAPve_g_L0_C2"
  Data Type Conversion239/1 -> Terminator230/1  "ob_IMAPve_g_L0_C1"
  Data Type Conversion237/1 -> Terminator228/1  "ob_IMAPve_d_ConsArea"
  Data Type Conversion235/1 -> Terminator226/1  "ob_IMAPve_d_Lane_Valid"
  Data Type Conversion238/1 -> Terminator229/1  "ob_IMAPve_g_L0_C0"
  Data Type Conversion236/1 -> Terminator227/1  "ob_IMAPve_d_Road_Type"
  Data Type Conversion246/1 -> Terminator237/1  "ob_IMAPve_g_L0_W"
  Data Type Conversion245/1 -> Terminator236/1  "ob_IMAPve_g_L0_Confidence"
  Data Type Conversion243/1 -> Terminator234/1  "ob_IMAPve_d_L0_Q"
  Data Type Conversion241/1 -> Terminator232/1  "ob_IMAPve_g_L0_C3"
  Data Type Conversion244/1 -> Terminator235/1  "ob_IMAPve_d_L0_Type"
  Data Type Conversion242/1 -> Terminator233/1  "ob_IMAPve_g_L0_VR"
  Data Type Conversion252/1 -> Terminator243/1  "ob_IMAPve_g_R0_C3"
  Data Type Conversion251/1 -> Terminator242/1  "ob_IMAPve_g_R0_C2"
  Data Type Conversion249/1 -> Terminator240/1  "ob_IMAPve_g_R0_C0"
  Data Type Conversion247/1 -> Terminator238/1  "ob_IMAPve_g_L0_TLC"
  Data Type Conversion250/1 -> Terminator241/1  "ob_IMAPve_g_R0_C1"
  Data Type Conversion248/1 -> Terminator239/1  "ob_IMAPve_d_L0_LC"
  Data Type Conversion258/1 -> Terminator249/1  "ob_IMAPve_g_R0_TLC"
  Data Type Conversion257/1 -> Terminator248/1  "ob_IMAPve_g_R0_W"
  Data Type Conversion255/1 -> Terminator246/1  "ob_IMAPve_d_R0_Type"
  Data Type Conversion253/1 -> Terminator244/1  "ob_IMAPve_g_R0_VR"
  Data Type Conversion256/1 -> Terminator247/1  "ob_IMAPve_g_R0_Confidence"
  Data Type Conversion254/1 -> Terminator245/1  "ob_IMAPve_d_R0_Q"
  Data Type Conversion264/1 -> Terminator255/1  "ob_IMAPve_g_L1_VR"
  Data Type Conversion263/1 -> Terminator254/1  "ob_IMAPve_g_L1_C3"
  Data Type Conversion261/1 -> Terminator252/1  "ob_IMAPve_g_L1_C1"
  Data Type Conversion259/1 -> Terminator250/1  "ob_IMAPve_d_R0_LC"
  Data Type Conversion262/1 -> Terminator253/1  "ob_IMAPve_g_L1_C2"
  Data Type Conversion260/1 -> Terminator251/1  "ob_IMAPve_g_L1_C0"
  Data Type Conversion270/1 -> Terminator261/1  "ob_IMAPve_d_L1_LC"
  Data Type Conversion269/1 -> Terminator260/1  "ob_IMAPve_g_L1_TLC"
  Data Type Conversion267/1 -> Terminator258/1  "ob_IMAPve_g_L1_Confidence"
  Data Type Conversion265/1 -> Terminator256/1  "ob_IMAPve_d_L1_Q"
  Data Type Conversion268/1 -> Terminator259/1  "ob_IMAPve_g_L1_W"
  Data Type Conversion266/1 -> Terminator257/1  "ob_IMAPve_d_L1_Type"
  Data Type Conversion276/1 -> Terminator267/1  "ob_IMAPve_d_R1_Q"
  Data Type Conversion275/1 -> Terminator266/1  "ob_IMAPve_g_R1_VR"
  Data Type Conversion273/1 -> Terminator264/1  "ob_IMAPve_g_R1_C2"
  Data Type Conversion271/1 -> Terminator262/1  "ob_IMAPve_g_R1_C0"
  Data Type Conversion274/1 -> Terminator265/1  "ob_IMAPve_g_R1_C3"
  Data Type Conversion272/1 -> Terminator263/1  "ob_IMAPve_g_R1_C1"
  Data Type Conversion281/1 -> Terminator272/1  "ob_IMAPve_d_R1_LC"
  Data Type Conversion279/1 -> Terminator270/1  "ob_IMAPve_g_R1_W"
  Data Type Conversion277/1 -> Terminator268/1  "ob_IMAPve_d_R1_Type"
  Data Type Conversion280/1 -> Terminator271/1  "ob_IMAPve_g_R1_TLC"
  Data Type Conversion278/1 -> Terminator269/1  "ob_IMAPve_g_R1_Confidence"
  Data Type Conversion287/1 -> Terminator278/1  "ob_IMAPve_g_L0_C0_FR_Pred"
  Data Type Conversion286/1 -> Terminator277/1  "ob_IMAPve_g_L0_Range_Back"
  Data Type Conversion284/1 -> Terminator275/1  "ob_IMAPve_g_L0_C2_Back"
  Data Type Conversion282/1 -> Terminator273/1  "ob_IMAPve_g_L0_C0_Back"
  Data Type Conversion285/1 -> Terminator276/1  "ob_IMAPve_g_L0_C3_Back"
  Data Type Conversion283/1 -> Terminator274/1  "ob_IMAPve_g_L0_C1_Back"
  Data Type Conversion293/1 -> Terminator284/1  "ob_IMAPve_g_R0_C2_Back"
  Data Type Conversion292/1 -> Terminator283/1  "ob_IMAPve_g_R0_C1_Back"
  Data Type Conversion290/1 -> Terminator281/1  "ob_IMAPve_g_L0_Range_FR_Pred"
  Data Type Conversion288/1 -> Terminator279/1  "ob_IMAPve_g_L0_C1_FR_Pred"
  Data Type Conversion291/1 -> Terminator282/1  "ob_IMAPve_g_R0_C0_Back"
  Data Type Conversion289/1 -> Terminator280/1  "ob_IMAPve_g_L0_C2_FR_Pred"
  Data Type Conversion299/1 -> Terminator290/1  "ob_IMAPve_g_R0_Range_FR_Pred"
  Data Type Conversion298/1 -> Terminator289/1  "ob_IMAPve_g_R0_C2_FR_Pred"
  Data Type Conversion296/1 -> Terminator287/1  "ob_IMAPve_g_R0_C0_FR_Pred"
  Data Type Conversion294/1 -> Terminator285/1  "ob_IMAPve_g_R0_C3_Back"
  Data Type Conversion297/1 -> Terminator288/1  "ob_IMAPve_g_R0_C1_FR_Pred"
  Data Type Conversion295/1 -> Terminator286/1  "ob_IMAPve_g_R0_Range_Back"
  Data Type Conversion305/1 -> Terminator296/1  "ob_IMAPve_g_L1_C0_FR_Pred"
  Data Type Conversion304/1 -> Terminator295/1  "ob_IMAPve_g_L1_Range_Back"
  Data Type Conversion302/1 -> Terminator293/1  "ob_IMAPve_g_L1_C2_Back"
  Data Type Conversion300/1 -> Terminator291/1  "ob_IMAPve_g_L1_C0_Back"
  Data Type Conversion303/1 -> Terminator294/1  "ob_IMAPve_g_L1_C3_Back"
  Data Type Conversion301/1 -> Terminator292/1  "ob_IMAPve_g_L1_C1_Back"
  Data Type Conversion311/1 -> Terminator302/1  "ob_IMAPve_g_R1_C2_Back"
  Data Type Conversion310/1 -> Terminator301/1  "ob_IMAPve_g_R1_C1_Back"
  Data Type Conversion308/1 -> Terminator299/1  "ob_IMAPve_g_L1_Range_FR_Pred"
  Data Type Conversion306/1 -> Terminator297/1  "ob_IMAPve_g_L1_C1_FR_Pred"
  Data Type Conversion309/1 -> Terminator300/1  "ob_IMAPve_g_R1_C0_Back"
  Data Type Conversion307/1 -> Terminator298/1  "ob_IMAPve_g_L1_C2_FR_Pred"
  Data Type Conversion317/1 -> Terminator308/1  "ob_IMAPve_g_R1_Range_FR_Pred"
  Data Type Conversion316/1 -> Terminator307/1  "ob_IMAPve_g_R1_C2_FR_Pred"
  Data Type Conversion314/1 -> Terminator305/1  "ob_IMAPve_g_R1_C0_FR_Pred"
  Data Type Conversion312/1 -> Terminator303/1  "ob_IMAPve_g_R1_C3_Back"
  Data Type Conversion315/1 -> Terminator306/1  "ob_IMAPve_g_R1_C1_FR_Pred"
  Data Type Conversion313/1 -> Terminator304/1  "ob_IMAPve_g_R1_Range_Back"
  Gain245/1 -> Data Type Conversion329/1, IMAPve_d_ORI_R1_LC/1  "IMAPve_d_ORI_R1_LC"
  Data Type Conversion329/1 -> Terminator320/1  "ob_IMAPve_d_ORI_R1_LC"
  Gain305/1 -> Data Type Conversion2/1, IMAPve_d_LDW_Warn_Mode/1  "IMAPve_d_LDW_Warn_Mode"
  Data Type Conversion516/1 -> Data Type Conversion3/1, IMAPve_d_Speed_Limit/1
  Gain307/1 -> Data Type Conversion4/1, IMAPve_d_ALC_TLC_Mode/1  "IMAPve_d_ALC_TLC_Mode"
  Gain308/1 -> Data Type Conversion5/1, IMAPve_d_ESA_Switch/1  "IMAPve_d_ESA_Switch"
  Data Type Conversion347/1 -> Data Type Conversion6/1, IMAPve_d_ELK_Switch/1
  Data Type Conversion348/1 -> Data Type Conversion7/1, IMAPve_d_APA_Command/1
  Data Type Conversion517/1 -> Data Type Conversion19/1, IMAPve_d_BSD_LCW_Switch/1
  Data Type Conversion519/1 -> Data Type Conversion21/1, IMAPve_d_RCTA_Swtich/1
  Data Type Conversion518/1 -> Data Type Conversion20/1, IMAPve_d_FCTA_Switch/1
  Data Type Conversion520/1 -> Data Type Conversion22/1, IMAPve_d_DOW_Switch/1
  Gain314/1 -> Data Type Conversion23/1, IMAPve_d_JA_Brake_Switch/1  "IMAPve_d_JA_Brake_Switch"
  Data Type Conversion356/1 -> IMAPve_d_JA_Alert_Sensitivity/1
  Data Type Conversion355/1 -> IMAPve_d_JA_Alert_Switch/1
  Data Type Conversion357/1 -> IMAPve_d_LF_Switch/1
  Data Type Conversion358/1 -> IMAPve_d_ICA_Config/1
  Data Type Conversion359/1 -> IMAPve_d_ALC_Sensitivity/1
  Data Type Conversion457/1 -> Data Type Conversion30/1, IMAPve_d_PEPS_Door_Lock_Req/1
  Gain317/1 -> Data Type Conversion31/1, IMAPve_d_BCM_Door_Lock_State/1  "IMAPve_d_BCM_Door_Lock_State"
  Data Type Conversion460/1 -> Data Type Conversion342/1, IMAPve_d_TBOX_LocalTimeY/1
  Data Type Conversion461/1 -> Data Type Conversion343/1, IMAPve_d_TBOX_LocalTimeM/1
  Data Type Conversion462/1 -> Data Type Conversion344/1, IMAPve_d_TBOX_LocalTimeD/1
  Data Type Conversion463/1 -> Data Type Conversion345/1, IMAPve_d_TBOX_LocalTimeH/1
  Data Type Conversion464/1 -> Data Type Conversion346/1, IMAPve_d_TBOX_LocalTimeMin/1
  Data Type Conversion465/1 -> Data Type Conversion349/1, IMAPve_d_TBOX_LocalTimeS/1
  Data Type Conversion459/1 -> Data Type Conversion138/1, IMAPve_g_BCM_Battery_Voltage/1
  Data Type Conversion466/1 -> Data Type Conversion350/1, IMAPve_d_TBOX_LocalTime_Valid/1
  Data Type Conversion471/1 -> Data Type Conversion362/1, IMAPve_g_EPS_PowerCon/1
  Data Type Conversion470/1 -> Data Type Conversion361/1, IMAPve_d_EPS_Warning_State/1
  Data Type Conversion469/1 -> Data Type Conversion360/1, IMAPve_g_EPS_LKA_Current/1
  Data Type Conversion472/1 -> Data Type Conversion363/1, IMAPve_g_EMS_Actual_IndT/1
  Data Type Conversion473/1 -> Data Type Conversion364/1, IMAPve_d_EMS_AccPedal_Fault/1
  Data Type Conversion474/1 -> Data Type Conversion365/1, IMAPve_d_TCU_PRND_State/1
  Data Type Conversion475/1 -> Data Type Conversion366/1, IMAPve_d_TCU_Shift_Valid/1
  Gain352/1 -> Data Type Conversion367/1, IMAPve_d_ESC_LatAcc_Valid/1  "IMAPve_d_ESC_LatAcc_Valid"
  Gain351/1 -> Data Type Conversion368/1, IMAPve_d_ESC_YawRate_Valid/1  "IMAPve_d_ESC_YawRate_Valid"
  Gain350/1 -> Data Type Conversion369/1, IMAPve_d_ESC_LonAcc_Valid/1  "IMAPve_d_ESC_LonAcc_Valid"
  Gain348/1 -> Data Type Conversion370/1, IMAPve_d_ESC_ABS_Valid/1  "IMAPve_d_ESC_ABS_Valid"
  Data Type Conversion476/1 -> Data Type Conversion371/1, IMAPve_d_ESC_ABS_AlarmSig/1
  Gain347/1 -> Data Type Conversion374/1, IMAPve_d_ESC_FL_WhlSpd_Fault/1  "IMAPve_d_ESC_FL_WhlSpd_Fault"
  Gain346/1 -> Data Type Conversion375/1, IMAPve_d_ESC_FR_WhlSpd_Fault/1  "IMAPve_d_ESC_FR_WhlSpd_Fault"
  Gain286/1 -> Data Type Conversion376/1, IMAPve_d_ESC_RL_WhlSpd_Fault/1  "IMAPve_d_ESC_RL_WhlSpd_Fault"
  Gain74/1 -> Data Type Conversion377/1, IMAPve_d_ESC_RR_WhlSpd_Fault/1  "IMAPve_d_ESC_RR_WhlSpd_Fault"
  Gain342/1 -> Data Type Conversion378/1, IMAPve_d_ESC_AEB_Available/1  "IMAPve_d_ESC_AEB_Available"
  Gain343/1 -> Data Type Conversion379/1, IMAPve_d_ESC_AEB_Active/1  "IMAPve_d_ESC_AEB_Active"
  Gain344/1 -> Data Type Conversion380/1, IMAPve_d_ESC_ACC_Available/1  "IMAPve_d_ESC_ACC_Available"
  Gain345/1 -> Data Type Conversion381/1, IMAPve_d_ESC_ACC_Active/1  "IMAPve_d_ESC_ACC_Active"
  Data Type Conversion477/1 -> Data Type Conversion382/1, IMAPve_d_EPB_Display_Req/1
  Data Type Conversion478/1 -> Data Type Conversion383/1, IMAPve_d_EPB_Warn_Req/1
  Data Type Conversion479/1 -> Data Type Conversion384/1, IMAPve_d_EPB_Switch_State/1
  Data Type Conversion480/1 -> Data Type Conversion385/1, IMAPve_d_EPB_Switch_Valid/1
  Gain336/1 -> Data Type Conversion386/1, IMAPve_d_ESC_EBD_AlarmSig/1  "IMAPve_d_ESC_EBD_AlarmSig"
  Data Type Conversion481/1 -> IMAPve_d_ESC_AVH_Status/1, Data Type Conversion387/1
  Data Type Conversion456/1 -> Data Type Conversion29/1, IMAPve_d_ESC_BrakeLamp_Req/1
  SWINve_y_ESC_FLWDirection/1 -> Gain84/1
  SWINve_y_MP5_AutoPilotSwitch/1 -> Gain292/1
  SWINve_y_ESC_FRWDirection/1 -> Gain89/1
  SWINve_y_ESC_TCSErrorStatus/1 -> Gain90/1
  SWINve_y_ESC_RRWDirection/1 -> Gain92/1
  SWINve_y_ESC_EPBErrorStatus/1 -> Gain93/1
  SWINve_y_ESC-RLWDirection/1 -> Gain91/1
  Data Type Conversion521/1 -> Data Type Conversion415/1, IMAPve_d_MP5_UPA_Switch/1
  Gain91/1 -> Data Type Conversion322/1, IMAPve_d_ESC_RLW_Direction/1  "IMAPve_d_ESC_RLW_Direction"
  Data Type Conversion451/1 -> Data Type Conversion411/1, IMAPve_d_TCU_TCU_Available/1
  Data Type Conversion447/1 -> Data Type Conversion331/1, IMAPve_d_ACU_RearLeft_Belt/1
  Data Type Conversion453/1 -> Data Type Conversion407/1, IMAPve_d_BCM_RightTurn_Switch/1
  Data Type Conversion511/1 -> Data Type Conversion231/1, IMAPve_d_MP5_DMS_SideView/1
  Data Type Conversion508/1 -> Data Type Conversion221/1, IMAPve_d_MP5_DMS_Sensity/1
  Data Type Conversion503/1 -> Data Type Conversion414/1, IMAPve_d_MP5_LanguageSet/1
  Data Type Conversion509/1 -> Data Type Conversion225/1, IMAPve_d_MP5_DMS_EyeFatigue/1
  Data Type Conversion444/1 -> Data Type Conversion327/1, IMAPve_d_EPS_Driver_Override/1
  Gain93/1 -> Data Type Conversion324/1, IMAPve_d_ESC_EPB_ErrorStatus/1  "IMAPve_d_ESC_EPB_ErrorStatus"
  Data Type Conversion514/1 -> Data Type Conversion234/1, IMAPve_d_MP5_DMS_DrinkWater/1
  Data Type Conversion501/1 -> Data Type Conversion413/1, IMAPve_d_MP5_APA_ModeSelect/1
  Gain89/1 -> Data Type Conversion320/1, IMAPve_d_ESC_FRW_Direction/1  "IMAPve_d_ESC_FRW_Direction"
  Data Type Conversion502/1 -> Data Type Conversion412/1, IMAPve_d_MP5_Work_State/1
  Data Type Conversion450/1 -> Data Type Conversion410/1, IMAPve_d_EMS_PowertrainCtl_State/1
  Data Type Conversion507/1 -> Data Type Conversion218/1, IMAPve_d_MP5_DMS_DelUserNum/1
  Data Type Conversion448/1 -> Data Type Conversion404/1, IMAPve_d_ACU_RearMiddle_Belt/1
  Gain84/1 -> Data Type Conversion319/1, IMAPve_d_ESC_FLW_Direction/1  "IMAPve_d_ESC_FLW_Direction"
  Data Type Conversion445/1 -> Data Type Conversion328/1, IMAPve_d_EPS_Driver_Active_ESA/1
  Data Type Conversion454/1 -> Data Type Conversion408/1, IMAPve_d_BCM_FrontWiper_Switch/1
  Gain292/1 -> Data Type Conversion48/1, IMAPve_d_SCC_Left_SwitchSig/1, Data Type Conversion417/1, IMAPve_d_MP5_AutoPilot_Switch/1  "IMAPve_d_MP5_AutoPilot_Switch"
  Data Type Conversion515/1 -> Data Type Conversion318/1, IMAPve_d_MP5_DMS_UserAccount/1
  Gain90/1 -> Data Type Conversion321/1, IMAPve_d_ESC_TCS_ErrorStatus/1  "IMAPve_d_ESC_TCS_ErrorStatus"
  Data Type Conversion513/1 -> Data Type Conversion233/1, IMAPve_d_MP5_DMS_Smoking/1
  Data Type Conversion510/1 -> Data Type Conversion226/1, IMAPve_d_MP5_DMS_LongtimeDrive/1
  Data Type Conversion442/1 -> Data Type Conversion325/1, IMAPve_d_EPS_SteeringAngle_Flag/1
  Data Type Conversion452/1 -> Data Type Conversion406/1, IMAPve_d_BCM_LeftTurn_Switch/1
  Data Type Conversion512/1 -> Data Type Conversion232/1, IMAPve_d_MP5_DMS_UsingPhone/1
  Data Type Conversion505/1 -> IMAPve_d_MP5_DMS_MessageType/1, Data Type Conversion216/1
  Data Type Conversion443/1 -> Data Type Conversion326/1, IMAPve_g_EPS_SteeringAngle/1
  Data Type Conversion504/1 -> Data Type Conversion416/1, IMAPve_d_MP5_FLK_Activation/1
  Data Type Conversion500/1 -> Data Type Conversion409/1, IMAPve_d_BCM_IHBC_Enabled/1
  Data Type Conversion449/1 -> Data Type Conversion405/1, IMAPve_d_ACU_RearRight_Belt/1
  Data Type Conversion446/1 -> Data Type Conversion330/1, IMAPve_d_EPS_ESA_State/1
  Gain92/1 -> Data Type Conversion323/1, IMAPve_d_ESC_RRW_Direction/1  "IMAPve_d_ESC_RRW_Direction"
  Data Type Conversion216/1 -> Terminator207/1  "ob_IMAPve_d_MP5_DMS_MessageType"
  Data Type Conversion217/1 -> Terminator208/1  "ob_IMAPve_d_MP5_DMS_SystemEnable"
  Data Type Conversion506/1 -> Data Type Conversion217/1, IMAPve_d_MP5_DMS_SystemEnable/1
  Data Type Conversion218/1 -> Terminator209/1  "ob_IMAPve_d_MP5_DMS_DelUserNum"
  Data Type Conversion221/1 -> Terminator212/1  "ob_IMAPve_d_MP5_DMS_Sensity"
  Data Type Conversion232/1 -> Terminator223/1  "ob_IMAPve_d_MP5_DMS_UsingPhone"
  Data Type Conversion225/1 -> Terminator216/1  "ob_IMAPve_d_MP5_DMS_EyeFatigue"
  Data Type Conversion231/1 -> Terminator222/1  "ob_IMAPve_d_MP5_DMS_SideView"
  Data Type Conversion226/1 -> Terminator217/1  "ob_IMAPve_d_MP5_DMS_LongtimeDrive"
  Data Type Conversion233/1 -> Terminator224/1  "ob_IMAPve_d_MP5_DMS_Smoking"
  Data Type Conversion318/1 -> Terminator309/1  "ob_IMAPve_d_MP5_DMS_UserAccount"
  Data Type Conversion234/1 -> Terminator225/1  "ob_IMAPve_d_MP5_DMS_DrinkWater"
  Data Type Conversion319/1 -> Terminator310/1  "ob_IMAPve_d_ESC_FLW_Direction"
  Data Type Conversion320/1 -> Terminator311/1  "ob_IMAPve_d_ESC_FRW_Direction"
  Data Type Conversion321/1 -> Terminator312/1  "ob_IMAPve_d_ESC_TCS_ErrorStatus"
  Data Type Conversion324/1 -> Terminator315/1  "ob_IMAPve_d_ESC_EPB_ErrorStatus"
  Data Type Conversion323/1 -> Terminator314/1  "ob_IMAPve_d_ESC_RRW_Direction"
  Data Type Conversion322/1 -> Terminator313/1  "ob_IMAPve_d_ESC_RLW_Direction"
  Data Type Conversion325/1 -> Terminator316/1  "ob_IMAPve_d_EPS_SteeringAngle_Flag"
  Data Type Conversion326/1 -> Terminator317/1  "ob_IMAPve_g_EPS_SteeringAngle"
  Data Type Conversion328/1 -> Terminator319/1  "ob_IMAPve_d_EPS_Driver_Active_ESA"
  Data Type Conversion327/1 -> Terminator318/1  "ob_IMAPve_d_EPS_Driver_Override"
  Data Type Conversion330/1 -> Terminator321/1  "ob_IMAPve_d_EPS_ESA_State"
  Data Type Conversion331/1 -> Terminator322/1  "ob_IMAPve_d_ACU_RearLeft_Belt"
  Data Type Conversion404/1 -> Terminator333/1  "ob_IMAPve_d_ACU_RearMiddle_Belt"
  Data Type Conversion405/1 -> Terminator334/1  "ob_IMAPve_d_ACU_RearRight_Belt"
  Data Type Conversion406/1 -> Terminator335/1  "ob_IMAPve_d_BCM_LeftTurn_Switch"
  Data Type Conversion407/1 -> Terminator336/1  "ob_IMAPve_d_BCM_RightTurn_Switch"
  Data Type Conversion408/1 -> Terminator337/1  "ob_IMAPve_d_BCM_FrontWiper_Switch"
  Data Type Conversion409/1 -> Terminator338/1  "ob_IMAPve_d_BCM_IHBC_Enabled"
  Data Type Conversion410/1 -> Terminator339/1  "ob_IMAPve_d_EMS_PowertrainCtl_State"
  Data Type Conversion411/1 -> Terminator340/1  "ob_IMAPve_d_TCU_TCU_Available"
  Data Type Conversion412/1 -> Terminator341/1  "ob_IMAPve_d_MP5_Work_State"
  Data Type Conversion413/1 -> Terminator342/1  "ob_IMAPve_d_MP5_APA_ModeSelect"
  Data Type Conversion414/1 -> Terminator343/1  "ob_IMAPve_d_MP5_LanguageSet"
  Data Type Conversion417/1 -> Terminator346/1  "ob_IMAPve_d_MP5_AutoPilot_Switch"
  Data Type Conversion415/1 -> Terminator344/1  "ob_IMAPve_d_MP5_UPA_Switch"
  Data Type Conversion416/1 -> Terminator345/1  "ob_IMAPve_d_MP5_FLK_Activation"
  Gain304/1 -> Data Type Conversion1/1, IMAPve_d_ISA_ISLC_Mode/1  "IMAPve_d_ISA_ISLC_Mode"
  SWINve_y_Mp5_ISAMode/1 -> Gain304/1
  SWINve_y_Mp5_LDWWarningMode/1 -> Gain305/1
  SWINve_y_MP5_TLCModeSelection/1 -> Gain307/1
  SWINve_y_MP5_ESASwitch/1 -> Gain308/1
  Data Type Conversion455/1 -> Data Type Conversion18/1, IMAPve_d_PEPS_RKE_Command/1
  SWINve_y_MP5_JASwitch/1 -> Gain314/1
  SWINve_y_BCM_DoorLockSt/1 -> Gain317/1
  Constant1/1 -> Data Type Conversion9/1
  Data Type Conversion468/1 -> Data Type Conversion354/1, IMAPve_d_EPS_Trq_State/1
  SWINve_y_ESC_EBDAlarmSig/1 -> Gain336/1
  SWINve_y_ESC_ACCAvailable/1 -> Gain344/1
  SWINve_y_ESC_ACCActive/1 -> Gain345/1
  SWINve_y_ESC_AEBAvailable/1 -> Gain342/1
  SWINve_y_ESC_AEBActive/1 -> Gain343/1
  Constant2/1 -> Data Type Conversion10/1
  Data Type Conversion10/1 -> Data Type Conversion132/1, IMAPve_d_ESC_AEB_Status/1
  Constant3/1 -> Data Type Conversion11/1
  Data Type Conversion11/1 -> Data Type Conversion133/1, IMAPve_d_ESC_ACC_Status/1
  SWINve_y_ESC_RRWHeelSpdFaultSignal/1 -> Gain74/1
  SWINve_y_ESC_RLWHeelSpdFaultSignal/1 -> Gain286/1
  SWINve_y_ESC_FRWHeelSpdFaultSignal/1 -> Gain346/1
  SWINve_y_ESC_FLWHeelSpdFaultSignal/1 -> Gain347/1
  SWINve_y_ESC_ABSValidity/1 -> Gain348/1
  SWINve_y_ESC_LongitudinalAccelerationValidity/1 -> Gain350/1
  SWINve_y_ESC_YawrateValidity/1 -> Gain351/1
  SWINve_y_ESC_LateralAccelarationValidity/1 -> Gain352/1
  Version/1 -> Terminator1/1  "ob_IMAP_Version"
  Constant6/1 -> Data Type Conversion12/1
  Constant7/1 -> Data Type Conversion13/1
  Constant8/1 -> Data Type Conversion14/1
  Constant9/1 -> Data Type Conversion15/1
  Constant10/1 -> Data Type Conversion16/1
  Constant11/1 -> Data Type Conversion17/1
  SWINve_y_BCM_RightlightSt/1 -> Gain48/1
  SWINve_y_BCM_LeftlightSt/1 -> Gain42/1
  SWINve_y_BCM_LRDoorSwitchSt/1 -> Gain353/1
  SWINve_y_BCM_RRDoorSwitchSt/1 -> Gain289/1
  SWINve_y_BCM_RFDoorSwitchSt/1 -> Gain279/1
  SWINve_y_BCM_LFDoorSwitchSt/1 -> Gain76/1
  SWINve_y_BCM_TrunkSt/1 -> Gain53/1
  Data Type Conversion1/1 -> Terminator2/1  "ob_IMAPve_d_ISA_ISLC_Mode"
  Data Type Conversion2/1 -> Terminator3/1  "ob_IMAPve_d_LDW_Warn_Mode"
  Data Type Conversion3/1 -> Terminator4/1  "ob_IMAPve_d_Speed_Limit"
  Data Type Conversion4/1 -> Terminator5/1  "ob_IMAPve_d_ALC_TLC_Mode"
  Data Type Conversion5/1 -> Terminator6/1  "ob_IMAPve_d_ESA_Switch"
  Data Type Conversion6/1 -> Terminator7/1  "ob_IMAPve_d_ELK_Switch"
  Constant4/1 -> Data Type Conversion347/1
  Constant5/1 -> Data Type Conversion348/1
  Data Type Conversion7/1 -> Terminator8/1  "ob_IMAPve_d_APA_Command"
  Data Type Conversion18/1 -> Terminator9/1  "ob_IMAPve_d_PEPS_RKE_Command"
  Data Type Conversion19/1 -> Terminator10/1  "ob_IMAPve_d_BSD_LCW_Switch"
  Data Type Conversion20/1 -> Terminator11/1  "ob_IMAPve_d_FCTA_Switch"
  Data Type Conversion21/1 -> Terminator12/1  "ob_IMAPve_d_RCTA_Swtich"
  Data Type Conversion22/1 -> Terminator13/1  "ob_IMAPve_d_DOW_Switch"
  Data Type Conversion23/1 -> Terminator14/1  "ob_IMAPve_d_JA_Brake_Switch"
  Constant12/1 -> Data Type Conversion24/1, Data Type Conversion355/1
  Data Type Conversion24/1 -> Terminator15/1  "ob_IMAPve_d_JA_Alert_Switch"
  Constant13/1 -> Data Type Conversion25/1, Data Type Conversion356/1
  Data Type Conversion25/1 -> Terminator16/1  "ob_IMAPve_d_JA_Alert_Sensitivity"
  Constant14/1 -> Data Type Conversion26/1, Data Type Conversion357/1
  Data Type Conversion26/1 -> Terminator17/1  "ob_IMAPve_d_LF_Switch"
  Constant15/1 -> Data Type Conversion27/1, Data Type Conversion358/1
  Data Type Conversion27/1 -> Terminator18/1  "ob_IMAPve_d_ICA_Config"
  Constant16/1 -> Data Type Conversion28/1, Data Type Conversion359/1
  Data Type Conversion28/1 -> Terminator19/1  "ob_IMAPve_d_ALC_Sensitivity"
  Data Type Conversion29/1 -> Terminator20/1  "ob_IMAPve_d_ESC_BrakeLamp_Req"
  Data Type Conversion30/1 -> Terminator21/1  "ob_IMAPve_d_PEPS_Door_Lock_Req"
  Data Type Conversion31/1 -> Terminator22/1  "ob_IMAPve_d_BCM_Door_Lock_State"
  Data Type Conversion32/1 -> Terminator23/1  "ob_IMAPve_d_BCM_LowBeam_State"
  Data Type Conversion9/1 -> Data Type Conversion33/1, IMAPve_d_Radar_Detective_Req/1
  Data Type Conversion33/1 -> Terminator26/1  "ob_IMAPve_d_Radar_Detective_Req"
  Data Type Conversion138/1 -> Terminator129/1  "ob_IMAPve_g_BCM_Battery_Voltage"
  Data Type Conversion342/1 -> Terminator347/1  "ob_IMAPve_d_TBOX_LocalTimeY"
  Data Type Conversion343/1 -> Terminator348/1  "ob_IMAPve_d_TBOX_LocalTimeM"
  Data Type Conversion344/1 -> Terminator349/1  "ob_IMAPve_d_TBOX_LocalTimeD"
  Data Type Conversion345/1 -> Terminator350/1  "ob_IMAPve_d_TBOX_LocalTimeH"
  Data Type Conversion346/1 -> Terminator351/1  "ob_IMAPve_d_TBOX_LocalTimeMin"
  Data Type Conversion349/1 -> Terminator352/1  "ob_IMAPve_d_TBOX_LocalTimeS"
  Data Type Conversion350/1 -> Terminator353/1  "ob_IMAPve_d_TBOX_LocalTime_Valid"
  Data Type Conversion351/1 -> Terminator354/1  "ob_IMAPve_d_ACC_Desired_Headway"
  Data Type Conversion372/1 -> Data Type Conversion351/1, IMAPve_d_ACC_Desired_Headway/1
  Data Type Conversion373/1 -> Data Type Conversion352/1, IMAPve_d_Signal_Time_Stamp/1
  Data Type Conversion352/1 -> Terminator355/1  "ob_IMAPve_d_Signal_Time_Stamp"
  Data Type Conversion353/1 -> Terminator356/1  "ob_IMAPve_d_Outside_Temp"
  Data Type Conversion354/1 -> Terminator357/1  "ob_IMAPve_d_EPS_Trq_State"
  Data Type Conversion360/1 -> Terminator358/1  "ob_IMAPve_g_EPS_LKA_Current"
  Data Type Conversion362/1 -> Terminator360/1  "ob_IMAPve_g_EPS_PowerCon"
  Data Type Conversion361/1 -> Terminator359/1  "ob_IMAPve_d_EPS_Warning_State"
  Data Type Conversion363/1 -> Terminator361/1  "ob_IMAPve_g_EMS_Actual_IndT"
  Data Type Conversion364/1 -> Terminator362/1  "ob_IMAPve_d_EMS_AccPedal_Fault"
  Data Type Conversion365/1 -> Terminator363/1  "ob_IMAPve_d_TCU_PRND_State"
  Data Type Conversion366/1 -> Terminator364/1  "ob_IMAPve_d_TCU_Shift_Valid"
  Data Type Conversion367/1 -> Terminator365/1  "ob_IMAPve_d_ESC_LatAcc_Valid"
  Data Type Conversion368/1 -> Terminator366/1  "ob_IMAPve_d_ESC_YawRate_Valid"
  Data Type Conversion369/1 -> Terminator367/1  "ob_IMAPve_d_ESC_LonAcc_Valid"
  Data Type Conversion370/1 -> Terminator368/1  "ob_IMAPve_d_ESC_ABS_Valid"
  Data Type Conversion371/1 -> Terminator369/1  "ob_IMAPve_d_ESC_ABS_AlarmSig"
  Data Type Conversion374/1 -> Terminator370/1  "ob_IMAPve_d_ESC_FL_WhlSpd_Fault"
  Data Type Conversion375/1 -> Terminator371/1  "ob_IMAPve_d_ESC_FR_WhlSpd_Fault"
  Data Type Conversion376/1 -> Terminator372/1  "ob_IMAPve_d_ESC_RL_WhlSpd_Fault"
  Data Type Conversion377/1 -> Terminator373/1  "ob_IMAPve_d_ESC_RR_WhlSpd_Fault"
  Data Type Conversion378/1 -> Terminator374/1  "ob_IMAPve_d_ESC_AEB_Available"
  Data Type Conversion379/1 -> Terminator375/1  "ob_IMAPve_d_ESC_AEB_Active"
  Data Type Conversion380/1 -> Terminator376/1  "ob_IMAPve_d_ESC_ACC_Available"
  Data Type Conversion381/1 -> Terminator377/1  "ob_IMAPve_d_ESC_ACC_Active"
  Data Type Conversion383/1 -> Terminator379/1  "ob_IMAPve_d_EPB_Warn_Req"
  Data Type Conversion382/1 -> Terminator378/1  "ob_IMAPve_d_EPB_Display_Req"
  Data Type Conversion385/1 -> Terminator381/1  "ob_IMAPve_d_EPB_Switch_Valid"
  Data Type Conversion384/1 -> Terminator380/1  "ob_IMAPve_d_EPB_Switch_State"
  Data Type Conversion386/1 -> Terminator382/1  "ob_IMAPve_d_ESC_EBD_AlarmSig"
  Data Type Conversion388/1 -> Terminator384/1  "ob_IMAPve_d_TPMS_Warn_Indicate"
  Data Type Conversion402/1 -> Data Type Conversion388/1, IMAPve_d_TPMS_Warn_Indicate/1
  Data Type Conversion387/1 -> Terminator383/1  "ob_IMAPve_d_ESC_AVH_Status"
  CAFDva_y_F_CameraData600/1 -> message_unpack/26(CAFDva_y_F_CameraData600)
  CAFDva_y_F_CameraData424/1 -> message_unpack/27(CAFDva_y_F_CameraData424)
  CAFDva_y_F_CameraData450/1 -> message_unpack/29(CAFDva_y_F_CameraData450)
  CAFDva_y_F_CameraData425/1 -> message_unpack/28(CAFDva_y_F_CameraData425)
  CAFDva_y_F_CameraData45C/1 -> message_unpack/33(CAFDva_y_F_CameraData45C)
  CAFDva_y_F_CameraData45A/1 -> message_unpack/31(CAFDva_y_F_CameraData45A)
  CAFDva_y_F_CameraData459/1 -> message_unpack/30(CAFDva_y_F_CameraData459)
  CAFDva_y_F_CameraData45B/1 -> message_unpack/32(CAFDva_y_F_CameraData45B)
  CAFDva_y_F_CameraData421/1 -> message_unpack/38(CAFDva_y_F_CameraData421)
  CAFDva_y_F_CameraData422/1 -> message_unpack/39(CAFDva_y_F_CameraData422)
  CAFDva_y_F_CameraData423/1 -> message_unpack/41(CAFDva_y_F_CameraData423)
  CAFDva_y_F_CameraData420/1 -> message_unpack/37(CAFDva_y_F_CameraData420)
  CAFDva_y_F_CameraData451/1 -> message_unpack/40(CAFDva_y_F_CameraData451)
  CAFDva_y_F_CameraData45E/1 -> message_unpack/35(CAFDva_y_F_CameraData45E)
  CAFDva_y_F_CameraData45D/1 -> message_unpack/34(CAFDva_y_F_CameraData45D)
  CAFDva_y_F_CameraData45F/1 -> message_unpack/36(CAFDva_y_F_CameraData45F)
  CAFDva_y_F_CameraData452/1 -> message_unpack/42(CAFDva_y_F_CameraData452)
  CAFDva_y_F_CameraData455/1 -> message_unpack/45(CAFDva_y_F_CameraData455)
  CAFDva_y_F_CameraData456/1 -> message_unpack/46(CAFDva_y_F_CameraData456)
  CAFDva_y_F_CameraData454/1 -> message_unpack/44(CAFDva_y_F_CameraData454)
  CAFDva_y_F_CameraData426/1 -> message_unpack/49(CAFDva_y_F_CameraData426)
  CAFDva_y_F_CameraData457/1 -> message_unpack/47(CAFDva_y_F_CameraData457)
  CAFDva_y_F_CameraData453/1 -> message_unpack/43(CAFDva_y_F_CameraData453)
  CAFDva_y_F_CameraData458/1 -> message_unpack/48(CAFDva_y_F_CameraData458)
  Constant77/1 -> Data Type Conversion332/1
  Constant78/1 -> Data Type Conversion333/1
  Constant79/1 -> Data Type Conversion137/1
  Constant80/1 -> Data Type Conversion334/1
  Constant81/1 -> Data Type Conversion335/1
  Constant82/1 -> Data Type Conversion336/1
  Constant83/1 -> Data Type Conversion337/1
  Constant84/1 -> Data Type Conversion338/1
  Constant85/1 -> Data Type Conversion339/1
  Constant86/1 -> Data Type Conversion340/1
  Constant87/1 -> Data Type Conversion341/1
  Constant88/1 -> Data Type Conversion424/1
  Constant89/1 -> Data Type Conversion429/1
  Constant90/1 -> Data Type Conversion430/1
  Constant92/1 -> Data Type Conversion432/1
  Constant93/1 -> Data Type Conversion433/1
  Constant94/1 -> Data Type Conversion434/1
  Constant95/1 -> Data Type Conversion435/1
  Constant96/1 -> Data Type Conversion436/1
  Constant97/1 -> Data Type Conversion437/1
  Constant98/1 -> Data Type Conversion438/1
  Constant99/1 -> Data Type Conversion439/1
  Constant100/1 -> Data Type Conversion440/1
  Constant101/1 -> Data Type Conversion441/1
  Constant102/1 -> Data Type Conversion442/1
  Constant103/1 -> Data Type Conversion443/1
  Constant104/1 -> Data Type Conversion444/1
  Constant105/1 -> Data Type Conversion445/1
  Constant106/1 -> Data Type Conversion446/1
  Constant107/1 -> Data Type Conversion447/1
  Constant108/1 -> Data Type Conversion448/1
  Constant109/1 -> Data Type Conversion449/1
  Constant110/1 -> Data Type Conversion450/1
  Constant111/1 -> Data Type Conversion451/1
  Constant112/1 -> Data Type Conversion452/1
  Constant113/1 -> Data Type Conversion453/1
  Constant114/1 -> Data Type Conversion454/1
  Constant115/1 -> Data Type Conversion455/1
  Constant116/1 -> Data Type Conversion456/1
  Constant117/1 -> Data Type Conversion457/1
  Constant119/1 -> Data Type Conversion459/1
  Constant120/1 -> Data Type Conversion460/1
  Constant121/1 -> Data Type Conversion461/1
  Constant122/1 -> Data Type Conversion462/1
  Constant123/1 -> Data Type Conversion463/1
  Constant124/1 -> Data Type Conversion464/1
  Constant126/1 -> Data Type Conversion466/1
  Constant125/1 -> Data Type Conversion465/1
  Constant128/1 -> Data Type Conversion468/1
  Constant129/1 -> Data Type Conversion469/1
  Constant130/1 -> Data Type Conversion470/1
  Constant131/1 -> Data Type Conversion471/1
  Constant132/1 -> Data Type Conversion472/1
  Constant133/1 -> Data Type Conversion473/1
  Constant134/1 -> Data Type Conversion474/1
  Constant135/1 -> Data Type Conversion475/1
  Constant136/1 -> Data Type Conversion476/1
  Constant137/1 -> Data Type Conversion477/1
  Constant138/1 -> Data Type Conversion478/1
  Constant139/1 -> Data Type Conversion479/1
  Constant140/1 -> Data Type Conversion480/1
  Constant141/1 -> Data Type Conversion481/1
  Constant142/1 -> Data Type Conversion482/1
  Constant143/1 -> Data Type Conversion483/1
  Gain19/1 -> Data Type Conversion32/1, IMAPve_d_BCM_LowBeam_State/1  "IMAPve_d_BCM_LowBeam_State"
  SWINve_y_BCM_LowBeamStatus/1 -> Gain19/1
  SWINve_g_AC_AmbTemp/1 -> Gain23/1
  Gain23/1 -> Data Type Conversion353/1, IMAPve_d_Outside_Temp/1  "SWINve_g_AC_AmbTemp"
  SWINve_y_High_Beam_Status/1 -> Gain25/1
  Gain25/1 -> Data Type Conversion458/1, IMAPve_d_High_Beam_State/1  "IMAPve_d_High_Beam_State"
  Data Type Conversion458/1 -> Terminator128/1  "ob_IMAPve_d_High_Beam_State"
  SWINve_y_Front_Fog_Lamp_Status/1 -> Gain26/1
  Gain26/1 -> Data Type Conversion467/1, IMAPve_d_Front_Fog_Lamp_State/1  "IMAPve_d_Front_Fog_Lamp_State"
  Data Type Conversion467/1 -> Terminator323/1  "ob_IMAPve_d_Front_Fog_Lamp_State"
  Gain27/1 -> Data Type Conversion484/1, IMAPve_d_Rear_Fog_Lamp_State/1  "IMAPve_d_Rear_Fog_Lamp_State"
  SWINve_y_Rear_Fog_Lamp_Status/1 -> Gain27/1
  Data Type Conversion484/1 -> Terminator324/1  "ob_IMAPve_d_Rear_Fog_Lamp_State"
  Data Type Conversion485/1 -> Terminator325/1  "ob_IMAPve_d_BCM_Rain_Intensity"
  SWINve_y_BCM1_Rain_Intensity/1 -> Gain28/1
  Gain28/1 -> Data Type Conversion485/1, IMAPve_d_BCM_Rain_Intensity/1  "IMAPve_d_BCM_Rain_Intensity"
  SWINve_y_BCM1_IND_OvertakinglampSwt_OnOff/1 -> Gain30/1
  Gain30/1 -> Data Type Conversion486/1, IMAPve_d_BCM_OvertakinglampSwt/1  "IMAPve_d_BCM_OvertakinglampSwt"
  Data Type Conversion486/1 -> Terminator326/1  "ob_IMAPve_d_BCM_OvertakinglampSwt"
  SWINve_y_kick_down/1 -> Gain32/1
  Gain32/1 -> Data Type Conversion487/1, IMAPve_d_EMS_Kickdown/1  "IMAPve_d_EMS_Kickdown"
  Data Type Conversion487/1 -> Terminator327/1  "ob_IMAPve_d_EMS_Kickdown"
  Data Type Conversion488/1 -> Terminator328/1  "ob_IMAPve_d_Powertrain_Torque_Valid"
  Gain34/1 -> Data Type Conversion488/1, IMAPve_d_Powertrain_Torque_Valid/1  "IMAPve_d_Powertrain_Torque_Valid"
  SWINve_y_Powertrain_Torque_Validity/1 -> Gain34/1
  SWINve_y_ESP_Status_ACCInfo_Error/1 -> Gain35/1
  Gain35/1 -> Data Type Conversion489/1, IMAPve_d_ESC_ACCInfo_Error/1  "IMAPve_d_ESC_ACCInfo_Error"
  Data Type Conversion489/1 -> Terminator329/1  "ob_IMAPve_d_ESC_ACCInfo_Error"
  Data Type Conversion490/1 -> Terminator330/1  "ob_IMAPve_d_ESC_Prefill_Response"
  SWINve_y_ESP_Status_Prefill_Response/1 -> Gain36/1
  Gain36/1 -> Data Type Conversion490/1, IMAPve_d_ESC_Prefill_Response/1  "IMAPve_d_ESC_Prefill_Response"
  Gain37/1 -> Data Type Conversion491/1, IMAPve_d_ESC_AEBJerk_Response/1  "IMAPve_d_ESC_AEBJerk_Response"
  SWINve_y_ESP_Status_AEBJerk_Response/1 -> Gain37/1
  Data Type Conversion491/1 -> Terminator331/1  "ob_IMAPve_d_ESC_AEBJerk_Response"
  Data Type Conversion492/1 -> Terminator332/1  "ob_IMAPve_d_ESC_FCW_DBS_Response"
  Gain39/1 -> Data Type Conversion492/1, IMAPve_d_ESC_FCW_DBS_Response/1  "IMAPve_d_ESC_FCW_DBS_Response"
  SWINve_y_ESP_Status_FCW_DBS_Response/1 -> Gain39/1
  Data Type Conversion493/1 -> Terminator404/1  "ob_IMAPve_d_ESC_AEBJerk_Available"
  Gain50/1 -> Data Type Conversion493/1, IMAPve_d_ESC_AEBJerk_Available/1  "IMAPve_d_ESC_AEBJerk_Available"
  SWINve_y_ESP_Status_AEBJerk_Available/1 -> Gain50/1
  Data Type Conversion494/1 -> Terminator409/1  "ob_IMAPve_d_ESC_FCW_DBS_Available"
  Gain52/1 -> Data Type Conversion494/1, IMAPve_d_ESC_FCW_DBS_Available/1  "IMAPve_d_ESC_FCW_DBS_Available"
  SWINve_y_ESP_Status_FCW_DBS_Available/1 -> Gain52/1
  Data Type Conversion495/1 -> Terminator410/1  "ob_IMAPve_d_ESC_Prefill_Available"
  Gain68/1 -> Data Type Conversion495/1, IMAPve_d_ESC_Prefill_Available/1  "IMAPve_d_ESC_Prefill_Available"
  SWINve_y_ESP_Status_Prefill_Available/1 -> Gain68/1
  Gain69/1 -> Data Type Conversion496/1, IMAPve_g_EPS_LKAOverlay_Trq/1  "IMAPve_g_EPS_LKAOverlay_Trq"
  SWINve_g_EPS1_IND_LKAOverlayTorque_Value/1 -> Gain69/1
  Data Type Conversion496/1 -> Terminator411/1  "ob_IMAPve_g_EPS_LKAOverlay_Trq"
  Gain70/1 -> Data Type Conversion497/1, IMAPve_g_EPS_DriverTorque/1  "IMAPve_g_EPS_DriverTorque"
  Data Type Conversion497/1 -> Terminator412/1  "ob_IMAPve_g_EPS_DriverTorque"
  SWINve_g_EPS1_IND_DriverTorque_Value/1 -> Gain70/1
  SWINve_y_EPS1_Status_HandsoffValid/1 -> Gain72/1
  Gain72/1 -> Data Type Conversion498/1, IMAPve_d_EPS_Steer_Hold_State_Valid/1  "IMAPve_d_EPS_Steer_Hold_State_Valid"
  Data Type Conversion498/1 -> Terminator413/1  "ob_IMAPve_d_EPS_Steer_Hold_State_Valid"
  SWINve_g_Mech_Loss_Eng_Trq/1 -> Gain73/1
  Gain73/1 -> Data Type Conversion499/1, IMAPve_g_EMS_Mech_Loss_Trq/1  "IMAPve_g_EMS_Mech_Loss_Trq"
  Data Type Conversion499/1 -> Terminator414/1  "ob_IMAPve_g_EMS_Mech_Loss_Trq"
  Constant118/1 -> Data Type Conversion500/1
  Constant127/1 -> Data Type Conversion501/1
  Constant144/1 -> Data Type Conversion502/1
  Constant145/1 -> Data Type Conversion503/1
  Constant146/1 -> Data Type Conversion504/1
  Constant147/1 -> Data Type Conversion505/1
  Constant148/1 -> Data Type Conversion506/1
  Constant149/1 -> Data Type Conversion507/1
  Constant150/1 -> Data Type Conversion508/1
  Constant152/1 -> Data Type Conversion510/1
  Constant151/1 -> Data Type Conversion509/1
  Constant154/1 -> Data Type Conversion512/1
  Constant153/1 -> Data Type Conversion511/1
  Constant156/1 -> Data Type Conversion514/1
  Constant155/1 -> Data Type Conversion513/1
  Constant157/1 -> Data Type Conversion515/1
  Constant158/1 -> Data Type Conversion516/1
  SWINve_y_MP5_BSD_LCW_Activation/1 -> Data Type Conversion517/1
  Constant163/1 -> Data Type Conversion521/1
  Constant164/1 -> Data Type Conversion522/1
  SWINve_y_MP5_FCTAActivation/1 -> Data Type Conversion518/1
  SWINve_y_MP5_RCTAActivation/1 -> Data Type Conversion519/1
  SWINve_y_MP5_DOWActivation/1 -> Data Type Conversion520/1
  message_unpack/44(IFC_VD_CIPV_ID) -> Gain1/1
  message_unpack/144(IFC_Line04_Dy) -> Gain239/1
  Data Type Conversion389/1 -> Terminator385/1  "ob_IMAPva_d_ORI_Obj_TimeStamp"
  Gain443/1 -> Data Type Conversion389/1, IMAPva_d_ORI_Obj_TimeStamp/1  "IMAPva_d_ORI_Obj_TimeStamp"
  message_unpack/41(IFC_obj_timestamp) -> Gain443/1
  Data Type Conversion390/1 -> Terminator386/1  "ob_IMAPve_d_ORI_FS_OutOfCalib"
  Gain439/1 -> Data Type Conversion390/1, IMAPve_d_ORI_FS_OutOfCalib/1  "IMAPve_d_ORI_FS_OutOfCalib"
  message_unpack/45(FS_Out_Of_Calib) -> Gain439/1
  Data Type Conversion400/1 -> Terminator396/1  "ob_IMAPve_d_ORI_FS_OutOfFocus0"
  Data Type Conversion391/1 -> Terminator387/1  "ob_IMAPve_d_ORI_FS_Rain"
  Data Type Conversion399/1 -> Terminator395/1  "ob_IMAPve_d_ORI_FS_FrozenWindshield0"
  Data Type Conversion397/1 -> Terminator393/1  "ob_IMAPve_d_ORI_FS_PartialBlockage0"
  Gain438/1 -> Data Type Conversion391/1, IMAPve_d_ORI_FS_Rain/1  "IMAPve_d_ORI_FS_Rain"
  Gain435/1 -> IMAPve_d_ORI_FS_OutOfFocus0/1, Data Type Conversion400/1  "IMAPve_d_ORI_FS_OutOfFocus0"
  Gain430/1 -> Data Type Conversion396/1, IMAPve_d_ORI_FS_BlurImage0/1  "IMAPve_d_ORI_FS_BlurImage0"
  Gain441/1 -> IMAPve_d_ORI_FS_Fog/1, Data Type Conversion392/1  "IMAPve_d_ORI_FS_Fog"
  message_unpack/47(FS_Fog) -> Gain441/1
  Gain440/1 -> Data Type Conversion393/1, IMAPve_d_ORI_FS_Splashes0/1  "IMAPve_d_ORI_FS_Splashes0"
  Data Type Conversion392/1 -> Terminator388/1  "ob_IMAPve_d_ORI_FS_Fog"
  message_unpack/48(FS_Splashes_0) -> Gain440/1
  message_unpack/55(FS_Out_Of_Focus_0) -> Gain435/1
  message_unpack/52(FS_Partial_Blockage_0) -> Gain431/1
  message_unpack/46(FS_Rain) -> Gain438/1
  Data Type Conversion398/1 -> Terminator394/1  "ob_IMAPve_d_ORI_FS_FullBlockage0"
  message_unpack/50(FS_Low_Sun_0) -> Gain429/1
  Gain436/1 -> IMAPve_d_ORI_FS_FrozenWindshield0/1, Data Type Conversion399/1  "IMAPve_d_ORI_FS_FrozenWindshield0"
  Gain428/1 -> Data Type Conversion394/1, IMAPve_d_ORI_FS_SunRay0/1  "IMAPve_d_ORI_FS_SunRay0"
  message_unpack/49(FS_Sun_Ray_0) -> Gain428/1
  message_unpack/53(FS_Full_Blockage_0) -> Gain437/1
  message_unpack/51(FS_Blur_Image_0) -> Gain430/1
  Gain431/1 -> Data Type Conversion397/1, IMAPve_d_ORI_FS_PartialBlockage0/1  "IMAPve_d_ORI_FS_PartialBlockage0"
  Data Type Conversion394/1 -> Terminator390/1  "ob_IMAPve_d_ORI_FS_SunRay0"
  Gain437/1 -> IMAPve_d_ORI_FS_FullBlockage0/1, Data Type Conversion398/1  "IMAPve_d_ORI_FS_FullBlockage0"
  Gain429/1 -> Data Type Conversion395/1, IMAPve_d_ORI_FS_LowSun0/1  "IMAPve_d_ORI_FS_LowSun0"
  Data Type Conversion396/1 -> Terminator392/1  "ob_IMAPve_d_ORI_FS_BlurImage0"
  Data Type Conversion393/1 -> Terminator389/1  "ob_IMAPve_d_ORI_FS_Splashes0"
  message_unpack/54(FS_Frozen_Windshield_0) -> Gain436/1
  Data Type Conversion395/1 -> Terminator391/1  "ob_IMAPve_d_ORI_FS_LowSun0"
  Data Type Conversion401/1 -> Terminator397/1  "ob_IMAPva_g_ORI_Obj_TTIPCStdDev"
  Data Type Conversion403/1 -> Terminator398/1  "ob_IMAPva_g_ORI_Obj_AbsAx"
  Gain434/1 -> Data Type Conversion401/1, IMAPva_g_ORI_Obj_TTIPCStdDev/1  "IMAPva_g_ORI_Obj_TTIPCStdDev"
  Gain432/1 -> IMAPva_g_ORI_Obj_AbsAy/1, Data Type Conversion418/1  "IMAPva_g_ORI_Obj_AbsAy"
  Data Type Conversion418/1 -> Terminator399/1  "ob_IMAPva_g_ORI_Obj_AbsAy"
  Gain433/1 -> Data Type Conversion403/1, IMAPva_g_ORI_Obj_AbsAx/1  "IMAPva_g_ORI_Obj_AbsAx"
  message_unpack/56(IFC_obj_TTIPC_StdDev) -> Gain434/1
  message_unpack/57(IFC_obj_abs_Ax) -> Gain433/1
  message_unpack/58(IFC_obj_abs_Ay) -> Gain432/1
  Data Type Conversion419/1 -> Terminator400/1  "ob_IMAPva_g_ORI_Obj_RelVely"
  message_unpack/60(IFC_obj_Rel_Vy) -> Gain444/1
  Gain444/1 -> Data Type Conversion419/1, IMAPva_g_ORI_Obj_RelVely/1  "IMAPva_g_ORI_Obj_RelVely"
  Data Type Conversion420/1 -> Terminator401/1  "ob_IMAPva_g_ORI_Obj_LateralDis"
  Gain427/1 -> Data Type Conversion420/1, IMAPva_g_ORI_Obj_LateralDis/1  "IMAPva_g_ORI_Obj_LateralDis"
  message_unpack/62(IFC_obj_Dy) -> Gain427/1
  Data Type Conversion425/1 -> Terminator406/1  "ob_IMAPva_g_ORI_Obj_RelVelyStdDev"
  message_unpack/63(IFC_obj_abs_AxStdDev) -> Gain426/1
  Data Type Conversion523/1 -> Terminator416/1  "ob_IMAPva_d_ORI_Obj_RelVelyValid"
  Data Type Conversion426/1 -> Terminator407/1  "ob_IMAPva_g_ORI_Obj_LongDisStdDev"
  Gain425/1 -> Data Type Conversion422/1, IMAPva_g_ORI_Obj_AbsAyStdDev/1  "IMAPva_g_ORI_Obj_AbsAyStdDev"
  Data Type Conversion422/1 -> Terminator403/1  "ob_IMAPva_g_ORI_Obj_AbsAyStdDev"
  Gain424/1 -> Data Type Conversion423/1, IMAPva_g_ORI_Obj_RelVelStdDev/1  "IMAPva_g_ORI_Obj_RelVelStdDev"
  Gain421/1 -> Data Type Conversion427/1, IMAPva_g_ORI_Obj_LateralDisStdDev/1  "IMAPva_g_ORI_Obj_LateralDisStdDev"
  message_unpack/68(IFC_obj_DyStdDev) -> Gain421/1
  Gain420/1 -> Data Type Conversion428/1, IMAPva_d_ORI_Obj_RelVelValid/1  "IMAPva_d_ORI_Obj_RelVelValid"
  Data Type Conversion421/1 -> Terminator402/1  "ob_IMAPva_g_ORI_Obj_AbsAxStdDev"
  Gain418/1 -> Data Type Conversion524/1, IMAPva_d_ORI_Obj_RelVelStdDevValid/1  "IMAPva_d_ORI_Obj_RelVelStdDevValid"
  Gain423/1 -> Data Type Conversion425/1, IMAPva_g_ORI_Obj_RelVelyStdDev/1  "IMAPva_g_ORI_Obj_RelVelyStdDev"
  Gain422/1 -> Data Type Conversion426/1, IMAPva_g_ORI_Obj_LongDisStdDev/1  "IMAPva_g_ORI_Obj_LongDisStdDev"
  Gain426/1 -> Data Type Conversion421/1, IMAPva_g_ORI_Obj_AbsAxStdDev/1  "IMAPva_g_ORI_Obj_AbsAxStdDev"
  message_unpack/66(IFC_obj_Rel_VyStdDev) -> Gain423/1
  message_unpack/70(IFC_obj_Rel_VyValid) -> Gain419/1
  message_unpack/65(IFC_obj_Rel_VxStdDev) -> Gain424/1
  Gain417/1 -> Data Type Conversion525/1, IMAPva_d_ORI_Obj_RelVelyStdDevValid/1  "IMAPva_d_ORI_Obj_RelVelyStdDevValid"
  Gain419/1 -> Data Type Conversion523/1, IMAPva_d_ORI_Obj_RelVelyValid/1  "IMAPva_d_ORI_Obj_RelVelyValid"
  message_unpack/69(IFC_obj_Rel_VxValid) -> Gain420/1
  message_unpack/67(IFC_obj_DxStdDev) -> Gain422/1
  Data Type Conversion428/1 -> Terminator415/1  "ob_IMAPva_d_ORI_Obj_RelVelValid"
  Data Type Conversion525/1 -> Terminator418/1  "ob_IMAPva_d_ORI_Obj_RelVelyStdDevValid"
  Data Type Conversion427/1 -> Terminator408/1  "ob_IMAPva_g_ORI_Obj_LateralDisStdDev"
  Data Type Conversion423/1 -> Terminator405/1  "ob_IMAPva_g_ORI_Obj_RelVelStdDev"
  message_unpack/64(IFC_obj_abs_AyStdDev) -> Gain425/1
  message_unpack/72(IFC_obj_Rel_VyStdDevValid) -> Gain417/1
  Data Type Conversion524/1 -> Terminator417/1  "ob_IMAPva_d_ORI_Obj_RelVelStdDevValid"
  message_unpack/71(IFC_obj_Rel_VxStdDevValid) -> Gain418/1
  Data Type Conversion527/1 -> Terminator420/1  "ob_IMAPva_g_ORI_Obj_ClassProb"
  Data Type Conversion526/1 -> Terminator419/1  "ob_IMAPva_g_ORI_Obj_ExistProb"
  Gain416/1 -> Data Type Conversion526/1, IMAPva_g_ORI_Obj_ExistProb/1  "IMAPva_g_ORI_Obj_ExistProb"
  Gain415/1 -> Data Type Conversion527/1, IMAPva_g_ORI_Obj_ClassProb/1  "IMAPva_g_ORI_Obj_ClassProb"
  message_unpack/74(IFC_obj_TypeProb) -> Gain415/1
  message_unpack/73(IFC_obj_ExistProb) -> Gain416/1
  Data Type Conversion530/1 -> Terminator423/1  "ob_IMAPva_g_ORI_Obj_WidthStdDev"
  message_unpack/76(IFC_obj_Height) -> Gain411/1
  message_unpack/78(IFC_obj_WidthStdDev) -> Gain413/1
  message_unpack/77(IFC_obj_LengthStdDev) -> Gain412/1
  message_unpack/79(IFC_obj_HeightStdDev) -> Gain414/1
  Gain413/1 -> Data Type Conversion530/1, IMAPva_g_ORI_Obj_WidthStdDev/1  "IMAPva_g_ORI_Obj_WidthStdDev"
  Gain411/1 -> Data Type Conversion528/1, IMAPva_g_ORI_Obj_Height/1  "IMAPva_g_ORI_Obj_Height"
  Gain412/1 -> Data Type Conversion529/1, IMAPva_g_ORI_Obj_LengthStdDev/1  "IMAPva_g_ORI_Obj_LengthStdDev"
  Gain414/1 -> Data Type Conversion531/1, IMAPva_g_ORI_Obj_HeightStdDev/1  "IMAPva_g_ORI_Obj_HeightStdDev"
  Data Type Conversion531/1 -> Terminator424/1  "ob_IMAPva_g_ORI_Obj_HeightStdDev"
  Data Type Conversion529/1 -> Terminator422/1  "ob_IMAPva_g_ORI_Obj_LengthStdDev"
  Data Type Conversion528/1 -> Terminator421/1  "ob_IMAPva_g_ORI_Obj_Height"
  Data Type Conversion539/1 -> Terminator432/1  "ob_IMAPva_g_ORI_Obj_PhiBottomStdDev"
  Data Type Conversion536/1 -> Terminator429/1  "ob_IMAPva_g_ORI_Obj_AngleRate"
  Gain404/1 -> IMAPva_d_ORI_Obj_Measured/1, Data Type Conversion540/1  "IMAPva_d_ORI_Obj_Measured"
  Data Type Conversion535/1 -> Terminator428/1  "ob_IMAPva_g_ORI_Obj_3DAngleStdDev"
  Gain399/1 -> Data Type Conversion532/1, IMAPva_g_ORI_Obj_3DAngle/1  "IMAPva_g_ORI_Obj_3DAngle"
  Gain400/1 -> Data Type Conversion534/1, IMAPva_g_ORI_Obj_RAngleStdDev/1  "IMAPva_g_ORI_Obj_RAngleStdDev"
  message_unpack/85(IFC_obj_angle_3DStdDev) -> Gain401/1
  Data Type Conversion540/1 -> Terminator433/1  "ob_IMAPva_d_ORI_Obj_Measured"
  message_unpack/83(IFC_obj_PhiLeftStdDev) -> Gain409/1
  Gain408/1 -> Data Type Conversion536/1, IMAPva_g_ORI_Obj_AngleRate/1  "IMAPva_g_ORI_Obj_AngleRate"
  message_unpack/93(IFC_obj_HeadOrientation) -> Gain407/1
  message_unpack/90(IFC_obj_Measured) -> Gain404/1
  Data Type Conversion532/1 -> Terminator425/1  "ob_IMAPva_g_ORI_Obj_3DAngle"
  message_unpack/86(IFC_obj_angle_rate) -> Gain408/1
  Gain407/1 -> Data Type Conversion543/1, IMAPva_d_ORI_Obj_HeadOrientation/1  "IMAPva_d_ORI_Obj_HeadOrientation"
  Data Type Conversion541/1 -> Terminator434/1  "ob_IMAPva_g_ORI_Obj_Heading"
  Gain406/1 -> Data Type Conversion542/1, IMAPva_g_ORI_Obj_HeadingStdDev/1  "IMAPva_g_ORI_Obj_HeadingStdDev"
  message_unpack/92(IFC_obj_HeadingStdDev) -> Gain406/1
  Gain403/1 -> Data Type Conversion539/1, IMAPva_g_ORI_Obj_PhiBottomStdDev/1  "IMAPva_g_ORI_Obj_PhiBottomStdDev"
  Gain405/1 -> IMAPva_g_ORI_Obj_Heading/1, Data Type Conversion541/1  "IMAPva_g_ORI_Obj_Heading"
  Data Type Conversion534/1 -> Terminator427/1  "ob_IMAPva_g_ORI_Obj_RAngleStdDev"
  message_unpack/89(IFC_obj_PhiBottomStdDev) -> Gain403/1
  message_unpack/88(IFC_obj_PhiBottom) -> Gain402/1
  message_unpack/84(IFC_obj_PhiRightStdDev) -> Gain400/1
  Gain402/1 -> IMAPva_g_ORI_Obj_PhiBottom/1, Data Type Conversion538/1  "IMAPva_g_ORI_Obj_PhiBottom"
  Data Type Conversion542/1 -> Terminator435/1  "ob_IMAPva_g_ORI_Obj_HeadingStdDev"
  message_unpack/82(IFC_obj_angle_3D) -> Gain399/1
  message_unpack/91(IFC_obj_Heading) -> Gain405/1
  message_unpack/87(IFC_obj_angle_rate_StdDev) -> Gain410/1
  Gain409/1 -> Data Type Conversion533/1, IMAPva_g_ORI_Obj_LAngleStdDev/1  "IMAPva_g_ORI_Obj_LAngleStdDev"
  Gain410/1 -> Data Type Conversion537/1, IMAPva_g_ORI_Obj_AngleRateStdDev/1  "IMAPva_g_ORI_Obj_AngleRateStdDev"
  Data Type Conversion533/1 -> Terminator426/1  "ob_IMAPva_g_ORI_Obj_LAngleStdDev"
  Data Type Conversion543/1 -> Terminator436/1  "ob_IMAPva_d_ORI_Obj_HeadOrientation"
  Data Type Conversion537/1 -> Terminator430/1  "ob_IMAPva_g_ORI_Obj_AngleRateStdDev"
  Gain401/1 -> Data Type Conversion535/1, IMAPva_g_ORI_Obj_3DAngleStdDev/1  "IMAPva_g_ORI_Obj_3DAngleStdDev"
  Data Type Conversion538/1 -> Terminator431/1  "ob_IMAPva_g_ORI_Obj_PhiBottom"
  Data Type Conversion544/1 -> Terminator437/1  "ob_IMAPva_g_ORI_Obj_TTIPC"
  Data Type Conversion545/1 -> Terminator438/1  "ob_IMAPva_d_ORI_Obj_DirectionIndicator"
  Gain392/1 -> Data Type Conversion544/1, IMAPva_g_ORI_Obj_TTIPC/1  "IMAPva_g_ORI_Obj_TTIPC"
  Gain394/1 -> IMAPva_d_ORI_Obj_BrakeLight/1, Data Type Conversion546/1  "IMAPva_d_ORI_Obj_BrakeLight"
  message_unpack/97(IFC_obj_DirIndicator) -> Gain393/1
  Gain398/1 -> IMAPve_d_ORI_L0_ColorClass/1, Data Type Conversion550/1  "IMAPve_d_ORI_L0_ColorClass"
  Gain395/1 -> IMAPve_d_ORI_L0_ID/1, Data Type Conversion547/1  "IMAPve_d_ORI_L0_ID"
  message_unpack/98(IFC_obj_BrakeLight) -> Gain394/1
  Data Type Conversion547/1 -> Terminator440/1  "ob_IMAPve_d_ORI_L0_ID"
  message_unpack/101(IFC_Line01_DxStart) -> Gain397/1
  message_unpack/99(IFC_Line01_LineID) -> Gain395/1
  Gain396/1 -> IMAPve_g_ORI_L0_ExistProb/1, Data Type Conversion548/1  "IMAPve_g_ORI_L0_ExistProb"
  message_unpack/100(IFC_Line01_ExistProb) -> Gain396/1
  message_unpack/96(IFC_obj_TTIPC) -> Gain392/1
  message_unpack/102(IFC_Line01_ColorClass) -> Gain398/1
  Gain393/1 -> Data Type Conversion545/1, IMAPva_d_ORI_Obj_DirectionIndicator/1  "IMAPva_d_ORI_Obj_DirectionIndicator"
  Data Type Conversion550/1 -> Terminator443/1  "ob_IMAPve_d_ORI_L0_ColorClass"
  Gain397/1 -> IMAPve_g_ORI_L0_DxStart/1, Data Type Conversion549/1  "IMAPve_g_ORI_L0_DxStart"
  Data Type Conversion548/1 -> Terminator441/1  "ob_IMAPve_g_ORI_L0_ExistProb"
  Data Type Conversion546/1 -> Terminator439/1  "ob_IMAPva_d_ORI_Obj_BrakeLight"
  Data Type Conversion549/1 -> Terminator442/1  "ob_IMAPve_g_ORI_L0_DxStart"
  Gain391/1 -> Data Type Conversion551/1, IMAPve_d_ORI_L0_MeasureType/1  "IMAPve_d_ORI_L0_MeasureType"
  message_unpack/108(IFC_Line01_MeasureType) -> Gain391/1
  Data Type Conversion551/1 -> Terminator444/1  "ob_IMAPve_d_ORI_L0_MeasureType"
  message_unpack/115(IFC_Line02_ColorClass) -> Gain388/1
  Gain388/1 -> Data Type Conversion555/1, IMAPve_d_ORI_R0_ColorClass/1
  Gain389/1 -> Data Type Conversion552/1, IMAPve_d_ORI_R0_ID/1
  Gain387/1 -> Data Type Conversion554/1, IMAPve_g_ORI_R0_Dxstart/1
  Gain390/1 -> Data Type Conversion553/1, IMAPve_g_ORI_R0_ExistProb/1
  message_unpack/113(IFC_Line02_ExistProb) -> Gain390/1
  message_unpack/111(IFC_Line01_TypeConf) -> Gain386/1
  Gain386/1 -> Data Type Conversion556/1, IMAPve_g_ORI_L0_TypeConf/1
  message_unpack/112(IFC_Line02_LineID) -> Gain389/1
  Data Type Conversion553/1 -> Terminator446/1  "ob_IMAPve_g_ORI_R0_ExistProb"
  Data Type Conversion554/1 -> Terminator447/1  "ob_IMAPve_g_ORI_R0_Dxstart"
  message_unpack/114(IFC_Line02_DxStart) -> Gain387/1
  Data Type Conversion555/1 -> Terminator448/1  "ob_IMAPve_d_ORI_R0_ColorClass"
  Data Type Conversion552/1 -> Terminator445/1  "ob_IMAPve_d_ORI_R0_ID"
  Data Type Conversion556/1 -> Terminator449/1  "ob_IMAPve_g_ORI_L0_TypeConf"
  message_unpack/121(IFC_Line02_MeasureType) -> Gain385/1
  Gain385/1 -> Data Type Conversion558/1, IMAPve_d_ORI_R0_MeasureType/1  "IMAPve_d_ORI_R0_MeasureType"
  Data Type Conversion558/1 -> Terminator450/1  "ob_IMAPve_d_ORI_R0_MeasureType"
  message_unpack/126(IFC_Line03_ExistProb) -> Gain384/1
  Gain380/1 -> Data Type Conversion557/1, IMAPve_g_ORI_R0_TypeConf/1  "IMAPve_g_ORI_R0_TypeConf"
